simulink model "bu_abslut125_romvect_float"  (R2021b)
settings: Solver=VariableStepAuto  StartTime=0.0  StopTime=350  RelTol=1e-3
undefined symbols (not defined in the file or in its folder): figd2104, xcu250
libraries: hdlBasic x1696, vmcUtilities x1
(part 2 of 8)

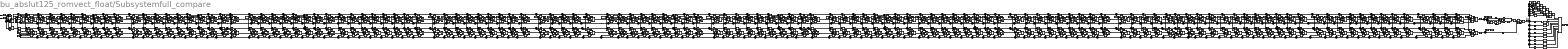
== system bu_abslut125_romvect_float/Subsystemfull_compare ==
  note: 120
  note: 110
  note: 100
  note: 90
  note: 80
  note: 70
  note: 30
  note: 01
  note: 50
  note: 40
  note: 20
  note: 10
  note: tiisai
  note: ooki
  note: 7874no13bit
  note: tmp_2
  note: tmp_3
  note: truthtable_out_x
  note: truthtable_out_y
  note: 1-1000
  note: 1001-2000
  note: 2001-3000
  note: 60
  note: 125
  note: 5001-6000
  note: 3001-4000
  note: 4001-5000
  note: 6001-7000
  note: 7001-7874
  In3 : Inport
  In4 : Inport  Port=2
  AddSub{,1..17,23..95,97..201,205..207,209..211,236,238,249..250,252,254..258,261..269,271..280,282..291,293..299} (248 alike) : hdlBasic/AddSub  mode=Addition  use_carryin=off  use_carryout=off  en=off  latency=1  precision=User Defined  arith_type="Signed  (2's comp)"  n_bits=32  bin_pt=0  quantization=Truncate  overflow=Wrap  use_behavioral_HDL=off  hw_selection=Fabric  pipelined=off  XmcBlockStatus=1  maskContainerNames=tabcontainer1  block_type=addsub  block_config=sysgen:Addsub_config
  AddSub18 : hdlBasic/AddSub  mode=Subtraction  use_carryin=off  use_carryout=off  en=off  latency=1  precision=Full  arith_type=Unsigned  n_bits=5  bin_pt=0  quantization=Truncate  overflow=Wrap  use_behavioral_HDL=off  hw_selection=Fabric  pipelined=off  XmcBlockStatus=1  maskContainerNames=tabcontainer1  block_type=addsub  block_config=sysgen:Addsub_config
  AddSub19 : hdlBasic/AddSub  mode=Addition  use_carryin=off  use_carryout=off  en=off  latency=1  precision=Full  arith_type=Unsigned  n_bits=16  bin_pt=14  quantization=Truncate  overflow=Wrap  use_behavioral_HDL=off  hw_selection=Fabric  pipelined=off  XmcBlockStatus=1  maskContainerNames=tabcontainer1  block_type=addsub  block_config=sysgen:Addsub_config
  AddSub20 : hdlBasic/AddSub  mode=Subtraction  use_carryin=off  use_carryout=off  en=off  latency=1  precision=User Defined  arith_type=Unsigned  n_bits=15  bin_pt=0  quantization="Round  (unbiased: +/- Inf)"  overflow=Saturate  use_behavioral_HDL=off  hw_selection=Fabric  pipelined=off  XmcBlockStatus=1  maskContainerNames=tabcontainer1  block_type=addsub  block_config=sysgen:Addsub_config
  AddSub{96,202..204,208,212} (6 alike) : hdlBasic/AddSub  mode=Addition  use_carryin=off  use_carryout=off  en=off  latency=1  precision=User Defined  arith_type=Unsigned  n_bits=3  bin_pt=0  quantization=Truncate  overflow=Wrap  use_behavioral_HDL=off  hw_selection=Fabric  pipelined=off  XmcBlockStatus=1  maskContainerNames=tabcontainer1  block_type=addsub  block_config=sysgen:Addsub_config
  AddSub21 : hdlBasic/AddSub  mode=Addition  use_carryin=off  use_carryout=off  en=off  latency=1  precision=Full  arith_type=Unsigned  n_bits=16  bin_pt=14  quantization=Truncate  overflow=Wrap  use_behavioral_HDL=off  hw_selection=Fabric  pipelined=off  XmcBlockStatus=1  maskContainerNames=tabcontainer1  block_type=addsub  block_config=sysgen:Addsub_config
  AddSub22 : hdlBasic/AddSub  mode=Subtraction  use_carryin=off  use_carryout=off  en=off  latency=1  precision=Full  arith_type=Unsigned  n_bits=17  bin_pt=0  quantization=Truncate  overflow=Wrap  use_behavioral_HDL=off  hw_selection=Fabric  pipelined=off  XmcBlockStatus=1  maskContainerNames=tabcontainer1  block_type=addsub  block_config=sysgen:Addsub_config
  Constant : hdlBasic/Constant  const=1.0  gui_display_data_type=Fixed-point  arith_type=Unsigned  n_bits=1  bin_pt=0  preci_type=Single  exp_width=8  frac_width=24  explicit_period=on  period=1  XmcBlockStatus=1  maskContainerNames=tabcontainer1  block_type=constant  block_config=sysgen:Constant_config
  Constant1 : hdlBasic/Constant  const=0  gui_display_data_type=Fixed-point  arith_type=Signed (2's comp)  n_bits=32  bin_pt=0  preci_type=Single  exp_width=8  frac_width=24  explicit_period=on  period=1  XmcBlockStatus=1  maskContainerNames=tabcontainer1  block_type=constant  block_config=sysgen:Constant_config
  Constant10 : hdlBasic/Constant  const=3000  gui_display_data_type=Fixed-point  arith_type=Unsigned  n_bits=12  bin_pt=0  preci_type=Single  exp_width=8  frac_width=24  explicit_period=on  period=1  XmcBlockStatus=1  maskContainerNames=tabcontainer1  block_type=constant  block_config=sysgen:Constant_config
  Constant11 : hdlBasic/Constant  const=4000  gui_display_data_type=Fixed-point  arith_type=Unsigned  n_bits=12  bin_pt=0  preci_type=Single  exp_width=8  frac_width=24  explicit_period=on  period=1  XmcBlockStatus=1  maskContainerNames=tabcontainer1  block_type=constant  block_config=sysgen:Constant_config
  Constant12 : hdlBasic/Constant  const=5000  gui_display_data_type=Fixed-point  arith_type=Unsigned  n_bits=13  bin_pt=0  preci_type=Single  exp_width=8  frac_width=24  explicit_period=on  period=1  XmcBlockStatus=1  maskContainerNames=tabcontainer1  block_type=constant  block_config=sysgen:Constant_config
  Constant13 : hdlBasic/Constant  const=6000  gui_display_data_type=Fixed-point  arith_type=Unsigned  n_bits=13  bin_pt=0  preci_type=Single  exp_width=8  frac_width=24  explicit_period=on  period=1  XmcBlockStatus=1  maskContainerNames=tabcontainer1  block_type=constant  block_config=sysgen:Constant_config
  Constant14 : hdlBasic/Constant  const=7000  gui_display_data_type=Fixed-point  arith_type=Unsigned  n_bits=13  bin_pt=0  preci_type=Single  exp_width=8  frac_width=24  explicit_period=on  period=1  XmcBlockStatus=1  maskContainerNames=tabcontainer1  block_type=constant  block_config=sysgen:Constant_config
  Constant2 : hdlBasic/Constant  const=1  gui_display_data_type=Fixed-point  arith_type=Signed (2's comp)  n_bits=32  bin_pt=0  preci_type=Single  exp_width=8  frac_width=24  explicit_period=on  period=1  XmcBlockStatus=1  maskContainerNames=tabcontainer1  block_type=constant  block_config=sysgen:Constant_config
  Constant3 : hdlBasic/Constant  const=248  gui_display_data_type=Fixed-point  arith_type=Unsigned  n_bits=8  bin_pt=0  preci_type=Single  exp_width=8  frac_width=24  explicit_period=on  period=1  XmcBlockStatus=1  maskContainerNames=tabcontainer1  block_type=constant  block_config=sysgen:Constant_config
  Constant4 : hdlBasic/Constant  const=125  gui_display_data_type=Fixed-point  arith_type=Unsigned  n_bits=7  bin_pt=0  preci_type=Single  exp_width=8  frac_width=24  explicit_period=on  period=1  XmcBlockStatus=1  maskContainerNames=tabcontainer1  block_type=constant  block_config=sysgen:Constant_config
  Constant5 : hdlBasic/Constant  const=1.0  gui_display_data_type=Fixed-point  arith_type=Unsigned  n_bits=10  bin_pt=0  preci_type=Single  exp_width=8  frac_width=24  explicit_period=on  period=1  XmcBlockStatus=1  maskContainerNames=tabcontainer1  block_type=constant  block_config=sysgen:Constant_config
  Constant6 : hdlBasic/Constant  const=0  gui_display_data_type=Fixed-point  arith_type=Signed (2's comp)  n_bits=32  bin_pt=0  preci_type=Single  exp_width=8  frac_width=24  explicit_period=on  period=1  XmcBlockStatus=1  maskContainerNames=tabcontainer1  block_type=constant  block_config=sysgen:Constant_config
  Constant7 : hdlBasic/Constant  const=1  gui_display_data_type=Fixed-point  arith_type=Signed (2's comp)  n_bits=32  bin_pt=0  preci_type=Single  exp_width=8  frac_width=24  explicit_period=on  period=1  XmcBlockStatus=1  maskContainerNames=tabcontainer1  block_type=constant  block_config=sysgen:Constant_config
  Constant8 : hdlBasic/Constant  const=1000  gui_display_data_type=Fixed-point  arith_type=Unsigned  n_bits=10  bin_pt=0  preci_type=Single  exp_width=8  frac_width=24  explicit_period=on  period=1  XmcBlockStatus=1  maskContainerNames=tabcontainer1  block_type=constant  block_config=sysgen:Constant_config
  Constant9 : hdlBasic/Constant  const=2000  gui_display_data_type=Fixed-point  arith_type=Unsigned  n_bits=11  bin_pt=0  preci_type=Single  exp_width=8  frac_width=24  explicit_period=on  period=1  XmcBlockStatus=1  maskContainerNames=tabcontainer1  block_type=constant  block_config=sysgen:Constant_config
  Convert23 : hdlBasic/Convert  Commented=on  gui_display_data_type=Fixed-point  arith_type=Unsigned  n_bits=13  bin_pt=0  float_type=Single  exp_bits=8  fraction_bits=24  quantization="Round  (unbiased: +/- Inf)"  overflow=Saturate  en=off  latency=1  pipeline=off  XmcBlockStatus=1  maskContainerNames=group2  block_type=convert  block_config=sysgen:Convert_config
  Delay{1..7,9..10,12..13,15..16,19..20,22..23,25..26,28..29,31..32,34..35,37..38,41..42,44..45,47..48,50..52,54..56,58,62,64..65,67..68,71..72,74..75,77..78,80..82,84..85,87..88,91..92,94..95,97..98,100..103,105..107,109..115,117..118,120..125,127..129,131,133..134,136..138,140..141,143..144,147..148,150..151,153..154,156..158,160..161,163..164,167..168,170..171,173..174,176..180,182..184,186,188..189,191..192,194..196,199..200,202..205,207,209..214,217..218,220..221,224..227,229,231..236,238..240,242..243,245,247..248,251..255,257..258,260..261,263..264,266..267,269..270,272..273,275..276,279..280,282..283,285..286,288..290,292..293,295..296,298..299,302..303,305..306,308..309,311..313,315..316,318..319,321,323..324,326..327,329..330,332..333,335..338,340,342..343,345..347,350..351,353..354,357..358,360..362,364..365,367..369,371..373,375..376,379..380,383..384,386..387,389..392,394,396..398,400,402..404,406..407,409..414,416..419,421,423,426..427,429..431,433..435,437..438,440,442..443,446,448..449,451..453,455..456,458..459,461,463,465..466,468..469,472..474,476..477,479..480,482..485,487..488,490..491,493..494,498..499,501..502,504..506,508..510,512..513,515..517,519,521..522,524..525,527,529,531..532,534..535,538..539,541..542,544..545,548..550,553..554,556..558,560..561,563..564,566,568..569,571..572,574..575,578..580,582..583,585..586,588,590..591,593..594,596..597,605,611..614,624..625,636..637,639..640,655..656,658..659,661..662,677..678,680..681,683..686,688,690..692,694,696..697,700..701,703..706,708,710..713,715,717,720..721,724..725,727,729,731..732,734,736..737,742..743,746..747,749..750,752..753,755,757,759..760,762..763,766,768,770..771,773..774,776..777,779,781..782,784..785,787..788,792..793,795..796,798..799,802..804,806..807,809..810,813,815..816,818..819,821,823} (503 alike) : hdlBasic/Delay  rst=off  en=off  latency=1  reg_retiming=off  XmcBlockStatus=1  maskContainerNames=group1  block_type=delay  block_config=sysgen:Delay_config
  Delay{8,11,14,17..18,21,24,27,30,33,36,39..40,43,46,49,53,57,63,66,69..70,73,76,79,83,86,89..90,93,96,99,104,108,116,119,126,130,132,135,139,142,145..146,149,152,155,159,162,165..166,169,172,175,181,185,187,190,193,201,206,215..216,219,222..223,228,230,237,241,244,246,249..250,256,259,262,265,268,271,274,277..278,281,284,287,291,294,297,300..301,304,307,310,314,317,320,322,325,328,331,334,339,341,344,348..349,352,355..356,359,363,366,370,374,377..378,381..382,385,388,393,395,399,401,405,408,415,420,422,424..425,428,432,436,439,441,444..445,447,450,454,457,460,462,464,467,470..471,475,478,481,486,489,492,495..497,500,503,507,511,514,518,520,523,526,528,530,533,536..537,540,543,546..547,551..552,555,559,562,565,567,570,573,576..577,581,584,587,589,592,595,598,606,610,615..617,635,638,657,660,679,682,689,693,695,699,702,709,714,718..719,722,726,730,735,738..739,741,744,748,751,754,758,761,764..765,769,772,775,780,783,786,790..791,794,797,801,805,808,812,814,817,820,824} (247 alike) : hdlBasic/Delay  rst=off  en=off  latency=2  reg_retiming=off  XmcBlockStatus=1  maskContainerNames=group1  block_type=delay  block_config=sysgen:Delay_config
  Delay{197..198,208,599..603} (8 alike) : hdlBasic/Delay  rst=off  en=off  latency=6  reg_retiming=off  XmcBlockStatus=1  maskContainerNames=group1  block_type=delay  block_config=sysgen:Delay_config
  Delay59 : hdlBasic/Delay  rst=off  en=off  latency=3  reg_retiming=off  XmcBlockStatus=1  maskContainerNames=group1  block_type=delay  block_config=sysgen:Delay_config
  Delay60 : hdlBasic/Delay  rst=off  en=off  latency=3  reg_retiming=off  XmcBlockStatus=1  maskContainerNames=group1  block_type=delay  block_config=sysgen:Delay_config
  Delay604 : hdlBasic/Delay  rst=off  en=off  latency=133  reg_retiming=off  XmcBlockStatus=1  maskContainerNames=group1  block_type=delay  block_config=sysgen:Delay_config
  Delay607 : hdlBasic/Delay  rst=off  en=off  latency=3  reg_retiming=off  XmcBlockStatus=1  maskContainerNames=group1  block_type=delay  block_config=sysgen:Delay_config
  Delay608 : hdlBasic/Delay  rst=off  en=off  latency=4  reg_retiming=off  XmcBlockStatus=1  maskContainerNames=group1  block_type=delay  block_config=sysgen:Delay_config
  Delay609 : hdlBasic/Delay  rst=off  en=off  latency=5  reg_retiming=off  XmcBlockStatus=1  maskContainerNames=group1  block_type=delay  block_config=sysgen:Delay_config
  Delay61 : hdlBasic/Delay  rst=off  en=off  latency=5  reg_retiming=off  XmcBlockStatus=1  maskContainerNames=group1  block_type=delay  block_config=sysgen:Delay_config
  Gate_In1 : hdlBasic/Gateway In  gui_display_data_type=Floating-point  arith_type=Floating-point  n_bits=16  bin_pt=15  preci_type=Double  exp_width=8  frac_width=24  rows=1  columns=1  quantization="Round  (unbiased: +/- Inf)"  overflow=Saturate  period=1  UseAsADC=off  ADCChannel='1'  interface=None  automatic_assignment=on  address_offset=hex2dec('00')  intf_name=''  intf_description=''  default_value=0  timing_constraint=None  locs_specified=off  LOCs={}  io_standard={}  inherit_from_input=off  hdl_port=on  XmcBlockStatus=1  maskContainerNames=group4  block_type=gatewayin  block_config=sysgen:gateway_in_config  block_width_w=590  block_height_w=620  block_width=640  block_height=850
  Gate_In2 : hdlBasic/Gateway In  gui_display_data_type=Floating-point  arith_type=Floating-point  n_bits=16  bin_pt=15  preci_type=Double  exp_width=8  frac_width=24  rows=1  columns=1  quantization="Round  (unbiased: +/- Inf)"  overflow=Saturate  period=1  UseAsADC=off  ADCChannel='1'  interface=None  automatic_assignment=on  address_offset=hex2dec('00')  intf_name=''  intf_description=''  default_value=0  timing_constraint=None  locs_specified=off  LOCs={}  io_standard={}  inherit_from_input=off  hdl_port=on  XmcBlockStatus=1  maskContainerNames=group4  block_type=gatewayin  block_config=sysgen:gateway_in_config  block_width_w=590  block_height_w=620  block_width=640  block_height=850
  Gateway Out : hdlBasic/Gateway Out  inherit_from_input=off  hdl_port=on  rows=1  columns=1  UseAsDAC=off  DACChannel='1'  interface=None  automatic_assignment=on  address_offset=hex2dec('00')  intf_name=''  intf_description=''  timing_constraint=None  locs_specified=off  LOCs={}  io_standard={}  XmcBlockStatus=1  maskContainerNames=group4  block_type=gatewayout  block_config=sysgen:gateway_out_config  block_width_w=590  block_height_w=620  block_width=620  block_height=750
  Gateway Out1 : hdlBasic/Gateway Out  inherit_from_input=off  hdl_port=on  rows=1  columns=1  UseAsDAC=off  DACChannel='1'  interface=None  automatic_assignment=on  address_offset=hex2dec('00')  intf_name=''  intf_description=''  timing_constraint=None  locs_specified=off  LOCs={}  io_standard={}  XmcBlockStatus=1  maskContainerNames=group4  block_type=gatewayout  block_config=sysgen:gateway_out_config  block_width_w=590  block_height_w=620  block_width=620  block_height=750
  Gateway Out2 : hdlBasic/Gateway Out  inherit_from_input=off  hdl_port=on  rows=1  columns=1  UseAsDAC=off  DACChannel='1'  interface=None  automatic_assignment=on  address_offset=hex2dec('00')  intf_name=''  intf_description=''  timing_constraint=None  locs_specified=off  LOCs={}  io_standard={}  XmcBlockStatus=1  maskContainerNames=group4  block_type=gatewayout  block_config=sysgen:gateway_out_config  block_width_w=590  block_height_w=620  block_width=620  block_height=750
  Mult : hdlBasic/Mult  precision=Full  arith_type="Signed  (2's comp)"  n_bits=30  bin_pt=16  quantization="Round  (unbiased: +/- Inf)"  overflow=Saturate  en=off  latency=1  use_behavioral_HDL=off  opt=Area  use_embedded=off  optimum_pipeline=off  pipeline=on  use_rpm=on  placement_style=Triangular  XmcBlockStatus=1  maskContainerNames=group1  block_type=mult  block_config=sysgen:Mult_config
  Mult1 : hdlBasic/Mult  precision=Full  arith_type="Signed  (2's comp)"  n_bits=16  bin_pt=14  quantization=Truncate  overflow=Wrap  en=off  latency=1  use_behavioral_HDL=off  opt=Area  use_embedded=off  optimum_pipeline=off  pipeline=on  use_rpm=on  placement_style=Triangular  XmcBlockStatus=1  maskContainerNames=group1  block_type=mult  block_config=sysgen:Mult_config
  Mux{,1..92,95..117,119..200,204..207,237..238,247..249,254..260,262..271,273..282,284..293,295..300} (250 alike) : hdlBasic/Mux  inputs=2  en=off  latency=1  precision=Full  arith_type=Unsigned  n_bits=16  bin_pt=14  quantization=Truncate  overflow=Wrap  XmcBlockStatus=1  maskContainerNames=tabcontainer1  block_type=mux  block_config=sysgen:Mux_config
  Mux93 : hdlBasic/Mux  inputs=8  en=off  latency=1  precision=Full  arith_type=Unsigned  n_bits=16  bin_pt=14  quantization=Truncate  overflow=Wrap  XmcBlockStatus=1  maskContainerNames=tabcontainer1  block_type=mux  block_config=sysgen:Mux_config
  Negate : hdlBasic/Negate  precision=Full  arith_type=Unsigned  n_bits=16  bin_pt=14  quantization=Truncate  overflow=Wrap  en=off  latency=1  XmcBlockStatus=1  maskContainerNames=tabcontainer1  block_type=negate  block_config=sysgen:Negate_config
  ROM : hdlBasic/ROM  depth=7874  initVector=[1.41421356237310,1.40285497510094,1.39140366620579,1.39159062000793,1.38004584520208,1.36859377003848,1.38042280392127,1.36878383930820,1.35723674105880,1.34578387387117,1.36935388882523,1.35762003300122,1.34597716419517,1.33442766399181,1.32297397770386,1.35838629242896,1.34655686869302,1.33481750556133,1.32317060012862,1.31161861541368,1.30016408153656,1.34752248865841,1.33559684733291,1.32376029217311,1.31201523429647,1.30036415295138,1.28880959683697,1.27735418536925,1.33676500806409,1.32474252892781,1.31280811258869,1.30096418258553,1.28921323279952,1.27755782892341,1.26600060988325,1.25454428920194,1.32611643813513,1.31399653297018,1.30196361745875,1.29002012584225,1.27816856491348,1.26641151564217,1.25475163475979,1.24319165629311,1.23173439303463,1.31557942351002,1.30336153876367,1.29122951997583,1.27918581025151,1.26723292744615,1.25537346595420,1.24361009846460,1.23194557767279,1.22038273793722,1.20892449686732,1.30515666607380,1.29284028563560,1.28060859621156,1.26846404780850,1.25640916736454,1.24444656070712,1.23257891448663,1.22080899807524,1.20913966541879,1.19757385682881,1.18611460070002,1.29485092493073,1.28243557302479,1.27010368532968,1.25785771666743,1.24570020094514,1.23363375328858,1.22166107216123,1.20978494145801,1.19800823256193,1.18633390635054,1.17476501513743,1.16330470453271,1.28466501624128,1.27215026043297,1.25971768966236,1.24736976135389,1.23510901413398,1.22293807014628,1.21085963736280,1.19887651188052,1.18699158019188,1.17520782141593,1.16352830947558,1.15195621520446,1.14049480836540,1.27460181291164,1.26198726722700,1.24945357463641,1.23700319282671,1.22463866275666,1.21236261115911,1.20017775305069,1.18808689423890,1.17609293381511,1.16419886662055,1.15240778567073,1.14072288452174,1.12914745956046,1.11768491219809,1.26466424412340,1.25194957227903,1.23931436853539,1.22676108837461,1.21429227256250,1.20191054984267,1.18961863965070,1.17741935483871,1.16531560439925,1.15331039617579,1.14140683954543,1.12960814805762,1.11791764201055,1.10633875094468,1.09487501603078,1.25485529469096,1.24204021343087,1.22930316208331,1.21664659133201,1.20407303908639,1.19158513337186,1.17918559525382,1.16687724178619,1.15466298897390,1.14254585473709,1.13052896186291,1.11861554092901,1.10680893318050,1.09511259333987,1.08353009232700,1.07206511986348,1.24517800423347,1.23226228676865,1.21942310783457,1.20666291059794,1.19398422731108,1.18138968240193,1.16888199561248,1.15646398517699,1.14413857103021,1.13190877803373,1.11977773920708,1.10774869894792,1.09582501622342,1.08401016771268,1.07230775087707,1.06072148693273,1.04925522369617,1.23563546614805,1.22261894569337,1.20967741935484,1.19681331994124,1.18402917111180,1.17132759066873,1.15871129391367,1.14618309706064,1.13374592069613,1.12140279327540,1.10915685464221,1.09701135955690,1.08496968121562,1.07303531474064,1.06121188061910,1.04950312806435,1.03791293827072,1.02644532752886,1.22623082637085,1.21311339977250,1.20006937017666,1.18710115707466,1.17421127246460,1.16140232434804,1.14867702030741,1.13603817115744,1.12348869466245,1.11103161930932,1.09867008812428,1.08640736251928,1.07424682615140,1.06219198877593,1.05024649007095,1.03841410340773,1.02669873953804,1.01510445016513,1.00363543136155,1.21696728191211,1.20374891335776,1.19060229251359,1.17752982248026,1.16453400039901,1.15161742115315,1.13878278116799,1.12603288230368,1.11337063583370,1.10079906650010,1.08832131663467,1.07594065033277,1.06366045766436,1.05148425890365,1.03941570875600,1.02745860055697,1.01561687041491,1.00389460126422,0.992296026791744,0.980825535194243,1.20784807915155,1.19452880395390,1.18127957571616,1.16810277796774,1.15500088967536,1.14197648914896,1.12903225806452,1.11617098559974,1.10339557267659,1.09070903630301,1.07811451400441,1.06561526833283,1.05321469143965,1.04091630969436,1.02872378832916,1.01664093608512,1.00467170983209,0.992820219129832,0.981090730693261,0.969487672719272,0.958015639026935,1.19887651188052,1.18545644032342,1.17210466445317 ...(+27333 chars)]  distributed_mem=Block RAM  rst=off  init_reg=0  en=off  latency=1  gui_display_data_type=Floating-point  arith_type=Floating-point  n_bits=16  bin_pt=15  preci_type=Double  exp_width=8  frac_width=24  optimize=Area  use_rpm=on  simulation_type=fast_sim  XmcBlockStatus=1  maskContainerNames=tabcontainer1  block_type=sprom  block_config=sysgen:SPROM_config
  ROM1 : hdlBasic/ROM  depth=7874  initVector=[0,0,0,0,0,0,0,0,0,0,0,0,0,0,0,0,0,0,0,0,0,0,0,0,0,0,0,0,0,0,0,0,0,0,0,0,0,0,0,0,0,0,0,0,0,0,0,0,0,0,0,0,0,0,0,0,0,0,0,0,0,0,0,0,0,0,0,0,0,0,0,0,0,0,0,0,0,0,0,0,0,0,0,0,0,0,0,0,0,0,0,0,0,0,0,0,0,0,0,0,0,0,0,0,0,0,0,0,0,0,0,0,0,0,0,0,0,0,0,0,0,0,0,0,0,0,0,0,0,0,0,0,0,0,0,0,0,0,0,0,0,0,0,0,0,0,0,0,0,0,0,0,0,0,0,0,0,0,0,0,0,0,0,0,0,0,0,0,0,0,0,0,0,0,0,0,0,0,0,0,0,0,0,0,0,0,0,0,0,0,0,0,0,0,0,0,0,0,0,0,0,0,0,0,0,0,0,0,0,0,0,0,0,0,0,0,0,0,0,0,0,0,0,0,0,0,0,0,0,0,0,0,0,0,0,0,0,0,0,0,0,0,0,0,0,0,0,0,0,0,0,0,0,0,0,0,0,0,0,0,0,0,0,0,0,0,0,0,0,0,0,0,0,0,0,0,0,0,0,0,0,0,0,0,0,0,0,0,0,0,0,0,0,0,0,0,0,0,0,0,0,0,0,0,0,0,0,0,0,0,0,0,0,0,0,0,0,0,0,0,0,0,0,0,0,0,0,0,0,0,0,0,0,0,0,0,0,0,0,0,0,0,0,0,0,0,0,0,0,0,0,0,0,0,0,0,0,0,0,0,0,0,0,0,0,0,0,0,0,0,0,0,0,0,0,0,0,0,0,0,0,0,0,0,0,0,0,0,0,0,0,0,0,0,0,0,0,0,0,0,0,0,0,0,0,0,0,0,0,0,0,0,0,0,0,0,0,0,0,0,0,0,0,0,0,0,0,0,0,0,0,0,0,0,0,0,0,0,0,0,0,0,0,0,0,0,0,0,0,0,0,0,0,0,0,0,0,0,0,0,0,0,0,0,0,0,0,0,0,0,0,0,0,0,0,0,0,0,0,0,0,0,0,0,0,0,0,0,0,0,0,0,0,0,0,0,0,0,0,0,0,0,0,0,0,0,0,0,0,0,0,0,0,0,0,0,0,0,0,0,0,0,0,0,0,0,0,0,0,0,0,0,0,0,0,0,0,0,0,0,0,0,0,0,0,0,0,0,0,0,0,0,0,0,0,0,0,0,0,0,0,0,0,0,0,0,0,0,0,0,0,0,0,0,0,0,0,0,0,0,0,0,0,0,0,0,0,0,0,0,0,0,0,0,0,0,0,0,0,0,0,0,0,0,0,0,0,0,0,0,0,0,0,0,0,0,0,0,0,0,0,0,0,0,0,0,0,0,0,0,0,0,0,0,0,0,0,0,0,0,0,0,0,0,0,0,0,0,0,0,0,0,0,0,0,0,0,0,0,0,0,0,0,0,0,0,0,0,0,0,0,0,0,0,0,0,0,0,0,0,0,0,0,0,0,0,0,0,0,0,0,0,0,0,0,0,0,0,0,0,0,0,0,0,0,0,0,0,0,0,0,0,0,0,0,0,0,0,0,0,0,0,0,0,0,0,0,0,0,0,0,0,0,0,0,0,0,0,0,0,0,0,0,0,0,0,0,0,0,0,0,0,0,0,0,0,0,0,0,0,0,0,0,0,0,0,0,0,0,0,0,0,0,0,0,0,0,0,0,0,0,0,0,0,0,0,0,0,0,0,0,0,0,0,0,0,0,0,0,0,0,0,0,0,0,0,0,0,0,0,0,0,0,0,0,0,0,0,0,0,0,0,0,0,0,0,0,0,0,0,0,0,0,0,0,0,0,0,0,0,0,0,0,0,0,0,0,0,0,0,0,0,0,0,0,0,0,0,0,0,0,0,0,0,0,0,0,0,0,0,0,0,0,0,0,0,0,0,0,0,0,0,0,0,0,0,0,0,0,0,0,0,0,0,0,0,0,0,0,0,0,0,0,0,0,0,0,0,0,0,0,0,0,0,0,0,0,0,0,0,0,0,0,0,0,0,0,0,0,0,0,0,0,0,0,0,0,0,0,0,0,0,0,0,0,0,0,0,0,0,0,0,0,0,0,0,0,0,0,0,0,0,0,0,0,0,0,0,0,0,0,0,0,0,0,0,0,0,0,0,0,0,0,0,0,0,0,0,0,0,0,0,0,0,0,0,0,0,0,0,0.887536547883716,0.872310792450965,0.857118081005576,0.841960202331496,0.826839072127503,0.811756744010427,0.796715421627643,0.781717472003396,0.766765440258369,0.751862065858495,0.737010300567475,0.722213328298004,0.707474587079397,0.692797793384340,0.678186969084795,0.663646471336806,0.649181025725745,0.634795763037240,0.620496260053914,0.606288584813307,0.592179346796317,0.578175752546288,0.564285667243094,0.550517682770194,0.536881192809459,0.523386475470579,0.510044783898126,0.496868445185463,0.483870967741935,0.471067156984201,0.458473238824255,0.446106989869011,0.433987872486249,0.422137171880723,0.410578131011544,1.03690988131906,1.02136388380565,1.00583624694638,0.990327834387661,0.974839563629779,0.959372410191165,0.943927412154809,0.928505675137049,0.913108377723752,0.897736777424242,0.882392217199350,0.867076132626814,0.851790059774896,0.836535643863867,0.821314648804775,0.806128967716116,0.790980634531563,0.775871836826174,0.760804930004565,0.745782453012703,0.730807145755432,0.715881968424908,0.701010122970991,0.686195076973634,0.671440590209634,0.656750744242011,0.642129975399819,0.627583111559475,0.613115413185426,0.598732619137761,0.584440997806240,0.570247404182700,0.556159343534409,0.542185042386181,0.528333527553523,0.514614713985285,0.501039502161583,0.487619885736483,0.474369069995250,0.461301601486293,0.448433508853479,0.435782454390526,0.423367895109893,0.411211251096192,0.399336077520643,0.387768234844236,1.03276197377949,1.01715258228565,1.00155965782323,0.985983981650189,0.970426384289763,0.954887749394560,0.939369017971680,0.923871193007722,0.908395344537337,0.892942615204284,0.877514226370029,0.862111484831792,0.846735790219786,0.831388643152250,0.816071654237001,0.800786554019768,0.785535203992640,0.770319608790939,0.755141929723847,0.740004499803514,0.724909840459491,0.709860680150496,0.694859975114130,0.679910932527677,0.665017036389945,0.650182076475690,0.635410180761039,0.620705851770770,0.606074007356643,0.591520026480395 ...(+27729 chars)]  distributed_mem=Block RAM  rst=off  init_reg=0  en=off  latency=1  gui_display_data_type=Floating-point  arith_type=Floating-point  n_bits=16  bin_pt=15  preci_type=Double  exp_width=8  frac_width=24  optimize=Area  use_rpm=on  simulation_type=fast_sim  XmcBlockStatus=1  maskContainerNames=tabcontainer1  block_type=sprom  block_config=sysgen:SPROM_config
  ROM2 : hdlBasic/ROM  depth=7874  initVector=[0,0,0,0,0,0,0,0,0,0,0,0,0,0,0,0,0,0,0,0,0,0,0,0,0,0,0,0,0,0,0,0,0,0,0,0,0,0,0,0,0,0,0,0,0,0,0,0,0,0,0,0,0,0,0,0,0,0,0,0,0,0,0,0,0,0,0,0,0,0,0,0,0,0,0,0,0,0,0,0,0,0,0,0,0,0,0,0,0,0,0,0,0,0,0,0,0,0,0,0,0,0,0,0,0,0,0,0,0,0,0,0,0,0,0,0,0,0,0,0,0,0,0,0,0,0,0,0,0,0,0,0,0,0,0,0,0,0,0,0,0,0,0,0,0,0,0,0,0,0,0,0,0,0,0,0,0,0,0,0,0,0,0,0,0,0,0,0,0,0,0,0,0,0,0,0,0,0,0,0,0,0,0,0,0,0,0,0,0,0,0,0,0,0,0,0,0,0,0,0,0,0,0,0,0,0,0,0,0,0,0,0,0,0,0,0,0,0,0,0,0,0,0,0,0,0,0,0,0,0,0,0,0,0,0,0,0,0,0,0,0,0,0,0,0,0,0,0,0,0,0,0,0,0,0,0,0,0,0,0,0,0,0,0,0,0,0,0,0,0,0,0,0,0,0,0,0,0,0,0,0,0,0,0,0,0,0,0,0,0,0,0,0,0,0,0,0,0,0,0,0,0,0,0,0,0,0,0,0,0,0,0,0,0,0,0,0,0,0,0,0,0,0,0,0,0,0,0,0,0,0,0,0,0,0,0,0,0,0,0,0,0,0,0,0,0,0,0,0,0,0,0,0,0,0,0,0,0,0,0,0,0,0,0,0,0,0,0,0,0,0,0,0,0,0,0,0,0,0,0,0,0,0,0,0,0,0,0,0,0,0,0,0,0,0,0,0,0,0,0,0,0,0,0,0,0,0,0,0,0,0,0,0,0,0,0,0,0,0,0,0,0,0,0,0,0,0,0,0,0,0,0,0,0,0,0,0,0,0,0,0,0,0,0,0,0,0,0,0,0,0,0,0,0,0,0,0,0,0,0,0,0,0,0,0,0,0,0,0,0,0,0,0,0,0,0,0,0,0,0,0,0,0,0,0,0,0,0,0,0,0,0,0,0,0,0,0,0,0,0,0,0,0,0,0,0,0,0,0,0,0,0,0,0,0,0,0,0,0,0,0,0,0,0,0,0,0,0,0,0,0,0,0,0,0,0,0,0,0,0,0,0,0,0,0,0,0,0,0,0,0,0,0,0,0,0,0,0,0,0,0,0,0,0,0,0,0,0,0,0,0,0,0,0,0,0,0,0,0,0,0,0,0,0,0,0,0,0,0,0,0,0,0,0,0,0,0,0,0,0,0,0,0,0,0,0,0,0,0,0,0,0,0,0,0,0,0,0,0,0,0,0,0,0,0,0,0,0,0,0,0,0,0,0,0,0,0,0,0,0,0,0,0,0,0,0,0,0,0,0,0,0,0,0,0,0,0,0,0,0,0,0,0,0,0,0,0,0,0,0,0,0,0,0,0,0,0,0,0,0,0,0,0,0,0,0,0,0,0,0,0,0,0,0,0,0,0,0,0,0,0,0,0,0,0,0,0,0,0,0,0,0,0,0,0,0,0,0,0,0,0,0,0,0,0,0,0,0,0,0,0,0,0,0,0,0,0,0,0,0,0,0,0,0,0,0,0,0,0,0,0,0,0,0,0,0,0,0,0,0,0,0,0,0,0,0,0,0,0,0,0,0,0,0,0,0,0,0,0,0,0,0,0,0,0,0,0,0,0,0,0,0,0,0,0,0,0,0,0,0,0,0,0,0,0,0,0,0,0,0,0,0,0,0,0,0,0,0,0,0,0,0,0,0,0,0,0,0,0,0,0,0,0,0,0,0,0,0,0,0,0,0,0,0,0,0,0,0,0,0,0,0,0,0,0,0,0,0,0,0,0,0,0,0,0,0,0,0,0,0,0,0,0,0,0,0,0,0,0,0,0,0,0,0,0,0,0,0,0,0,0,0,0,0,0,0,0,0,0,0,0,0,0,0,0,0,0,0,0,0,0,0,0,0,0,0,0,0,0,0,0,0,0,0,0,0,0,0,0,0,0,0,0,0,0,0,0,0,0,0,0,0,0,0,0,0,0,0,0,0,0,0,0,0,0,0,0,0,0,0,0,0,0,0,0,0,0,0,0,0,0,0,0,0,0,0,0,0,0,0,0,0,0,0,0,0,0,0,0,0,0,0,0,0,0,0,0,0,0,0,0,0,0,0,0,0,0,0,0,0,0,0,0,0,0,0,0,0,0,0,0,0,0,0,0,0,0,0,0,0,0,0,0,0,0,0,0,0,0,0,0,0,0,0,0,0,0,0,0,0,0,0,0,0,0,0,0,0,0,0,0,0,0,0,0,0,0,0,0,0,0,0,0,0,0,0,0,0,0,0,0,0,0,0,0,0,0,0,0,0,0,0,0,0,0,0,0,0,0,0,0,0,0,0,0,0,0,0,0,0,0,0,0,0,0,0,0,0,0,0,0,0,0,0,0,0,0,0,0,0,0,0,0,0,0,0,0,0,0,0,0,0,0,0,0,0,0,0,0,0,0,0,0,0,0,0,0,0,0,0,0,0,0,0,0,0,0,0,0,0,0,0,0,0,0,0,0,0,0,0,0,0,0,0,0,0,0,0,0,0,0,0,0,0,0,0,0,0,0,0,0,0,0,0,0,0,0,0,0,0,0,0,0,0,0,0,0,0,0,0,0,0,0,0,0,0,0,0,0,0,0,0,0,0,0,0,0,0,0,0,0,0,0,0,0,0,0,0,0,0,0,0,0,0,0,0,0,0,0,0,0,0,0,0,0,0,0,0,0,0,0,0,0,0,0,0,0,0,0,0,0,0,0,0,0,0,0,0,0,0,0,0,0,0,0,0,0,0,0,0,0,0,0,0,0,0,0,0,0,0,0,0,0,0,0,0,0,0,0,0,0,0,0,0,0,0,0,0,0,0,0,0,0,0,0,0,0,0,0,0,0,0,0,0,0,0,0,0,0,0,0,0,0,0,0,0,0,0,0,0,0,0,0,0,0,0,0,0,0,0,0,0,0,0,0,0,0,0,0,0,0,0,0,0,0,0,0,0,0,0,0,0,0,0,0,0,0,0,0,0,0,0,0,0,0,0,0,0,0,0,0,0,0,0,0,0,0,0,0,0,0,0,0,0,0,0,0,0,0,0,0,0,0,0,0,0,0,0,0,0,0,0,0,0,0,0,0,0,0,0,0,0,0,0,0,0,0,0,0,0,0,0,0,0,0,0,0,0,0,0,0,0,0,0,0,0,0,0,0,0,0,0,0,0,0,0,0,0,0,0,0,0,0,0,0,0,0,0,0,0,0,0,0,0,0,0,0,0,0,0,0,0,0,0,0,0,0,0,0,0,0,0,0,0,0,0,0,0,0,0,0,0,0,0,0,0,0,0,0,0,0,0,0,0,0,0,0,0,0,0,0,0,0,0,0,0,0,0,0,0,0,0,0,0,0,0,0,0,0,0,0,0,0,0,0,0,0,0,0,0,0,0,0,0,0,0,0,0,0,0,0,0,0,0,0,0,0,0,0,0,0,0,0,0,0,0,0,0,0,0,0,0,0,0,0,0,0,0,0,0,0,0,0,0,0,0,0,0,0,0,0,0,0,0,0,0,0,0,0,0,0,0,0,0,0,0,0,0,0,0,0,0,0,0,0,0,0,0,0,0,0,0,0,0,0,0,0,0,0,0,0,0,0,0,0,0,0,0,0,0,0,0,0,0,0,0,0,0,0,0,0,0,0,0,0,0,0,0,0,0,0,0,0,0,0,0,0,0,0,0,0,0,0,0,0,0,0,0,0,0,0,0,0,0,0,0,0,0,0,0,0,0,0,0,0,0,0,0,0,0,0,0,0,0,0,0,0,0,0,0,0,0,0,0,0,0,0,0,0,0,0,0,0,0,0,0,0,0,0,0,0,0,0,0,0,0,0,0,0,0,0,0,0,0,0,0,0,0,0,0,0,0,0,0,0,0,0,0,0,0,0,0,0,0,0,0,0,0,0,0,0,0,0,0,0,0,0,0,0,0,0,0,0,0,0,0,0,0,0,0,0,0,0,0,0,0,0,0,0,0,0,0,0,0,0,0,0,0,0,0,0,0,0,0,0,0,0,0,0,0,0,0,0,0,0,0,0,0,0,0,0,0,0,0,0,0,0,0,0,0,0,0,0,0,0,0,0,0,0,0,0,0,0,0,0,0,0,0,0,0,0,0,0,0,0,0,0,0,0,0,0,0,0,0,0,0,0,0,0,0,0,0,0,0,0,0,0,0,0,0,0,0,0,0,0,0,0,0,0,0,0,0,0,0,0,0,0,0,0,0,0,0,0,0,0,0,0,0,0,0,0,0,0,0,0,0,0,0,0,0,0,0,0,0,0,0,0,0,0,0,0,0,0,0,0,0,0,0,0,0,0,0,0,0,0,0,0,0,0 ...(+27783 chars)]  distributed_mem=Block RAM  rst=off  init_reg=0  en=off  latency=1  gui_display_data_type=Floating-point  arith_type=Floating-point  n_bits=16  bin_pt=15  preci_type=Double  exp_width=8  frac_width=24  optimize=Area  use_rpm=on  simulation_type=fast_sim  XmcBlockStatus=1  maskContainerNames=tabcontainer1  block_type=sprom  block_config=sysgen:SPROM_config
  ROM3 : hdlBasic/ROM  depth=7874  initVector=[0,0,0,0,0,0,0,0,0,0,0,0,0,0,0,0,0,0,0,0,0,0,0,0,0,0,0,0,0,0,0,0,0,0,0,0,0,0,0,0,0,0,0,0,0,0,0,0,0,0,0,0,0,0,0,0,0,0,0,0,0,0,0,0,0,0,0,0,0,0,0,0,0,0,0,0,0,0,0,0,0,0,0,0,0,0,0,0,0,0,0,0,0,0,0,0,0,0,0,0,0,0,0,0,0,0,0,0,0,0,0,0,0,0,0,0,0,0,0,0,0,0,0,0,0,0,0,0,0,0,0,0,0,0,0,0,0,0,0,0,0,0,0,0,0,0,0,0,0,0,0,0,0,0,0,0,0,0,0,0,0,0,0,0,0,0,0,0,0,0,0,0,0,0,0,0,0,0,0,0,0,0,0,0,0,0,0,0,0,0,0,0,0,0,0,0,0,0,0,0,0,0,0,0,0,0,0,0,0,0,0,0,0,0,0,0,0,0,0,0,0,0,0,0,0,0,0,0,0,0,0,0,0,0,0,0,0,0,0,0,0,0,0,0,0,0,0,0,0,0,0,0,0,0,0,0,0,0,0,0,0,0,0,0,0,0,0,0,0,0,0,0,0,0,0,0,0,0,0,0,0,0,0,0,0,0,0,0,0,0,0,0,0,0,0,0,0,0,0,0,0,0,0,0,0,0,0,0,0,0,0,0,0,0,0,0,0,0,0,0,0,0,0,0,0,0,0,0,0,0,0,0,0,0,0,0,0,0,0,0,0,0,0,0,0,0,0,0,0,0,0,0,0,0,0,0,0,0,0,0,0,0,0,0,0,0,0,0,0,0,0,0,0,0,0,0,0,0,0,0,0,0,0,0,0,0,0,0,0,0,0,0,0,0,0,0,0,0,0,0,0,0,0,0,0,0,0,0,0,0,0,0,0,0,0,0,0,0,0,0,0,0,0,0,0,0,0,0,0,0,0,0,0,0,0,0,0,0,0,0,0,0,0,0,0,0,0,0,0,0,0,0,0,0,0,0,0,0,0,0,0,0,0,0,0,0,0,0,0,0,0,0,0,0,0,0,0,0,0,0,0,0,0,0,0,0,0,0,0,0,0,0,0,0,0,0,0,0,0,0,0,0,0,0,0,0,0,0,0,0,0,0,0,0,0,0,0,0,0,0,0,0,0,0,0,0,0,0,0,0,0,0,0,0,0,0,0,0,0,0,0,0,0,0,0,0,0,0,0,0,0,0,0,0,0,0,0,0,0,0,0,0,0,0,0,0,0,0,0,0,0,0,0,0,0,0,0,0,0,0,0,0,0,0,0,0,0,0,0,0,0,0,0,0,0,0,0,0,0,0,0,0,0,0,0,0,0,0,0,0,0,0,0,0,0,0,0,0,0,0,0,0,0,0,0,0,0,0,0,0,0,0,0,0,0,0,0,0,0,0,0,0,0,0,0,0,0,0,0,0,0,0,0,0,0,0,0,0,0,0,0,0,0,0,0,0,0,0,0,0,0,0,0,0,0,0,0,0,0,0,0,0,0,0,0,0,0,0,0,0,0,0,0,0,0,0,0,0,0,0,0,0,0,0,0,0,0,0,0,0,0,0,0,0,0,0,0,0,0,0,0,0,0,0,0,0,0,0,0,0,0,0,0,0,0,0,0,0,0,0,0,0,0,0,0,0,0,0,0,0,0,0,0,0,0,0,0,0,0,0,0,0,0,0,0,0,0,0,0,0,0,0,0,0,0,0,0,0,0,0,0,0,0,0,0,0,0,0,0,0,0,0,0,0,0,0,0,0,0,0,0,0,0,0,0,0,0,0,0,0,0,0,0,0,0,0,0,0,0,0,0,0,0,0,0,0,0,0,0,0,0,0,0,0,0,0,0,0,0,0,0,0,0,0,0,0,0,0,0,0,0,0,0,0,0,0,0,0,0,0,0,0,0,0,0,0,0,0,0,0,0,0,0,0,0,0,0,0,0,0,0,0,0,0,0,0,0,0,0,0,0,0,0,0,0,0,0,0,0,0,0,0,0,0,0,0,0,0,0,0,0,0,0,0,0,0,0,0,0,0,0,0,0,0,0,0,0,0,0,0,0,0,0,0,0,0,0,0,0,0,0,0,0,0,0,0,0,0,0,0,0,0,0,0,0,0,0,0,0,0,0,0,0,0,0,0,0,0,0,0,0,0,0,0,0,0,0,0,0,0,0,0,0,0,0,0,0,0,0,0,0,0,0,0,0,0,0,0,0,0,0,0,0,0,0,0,0,0,0,0,0,0,0,0,0,0,0,0,0,0,0,0,0,0,0,0,0,0,0,0,0,0,0,0,0,0,0,0,0,0,0,0,0,0,0,0,0,0,0,0,0,0,0,0,0,0,0,0,0,0,0,0,0,0,0,0,0,0,0,0,0,0,0,0,0,0,0,0,0,0,0,0,0,0,0,0,0,0,0,0,0,0,0,0,0,0,0,0,0,0,0,0,0,0,0,0,0,0,0,0,0,0,0,0,0,0,0,0,0,0,0,0,0,0,0,0,0,0,0,0,0,0,0,0,0,0,0,0,0,0,0,0,0,0,0,0,0,0,0,0,0,0,0,0,0,0,0,0,0,0,0,0,0,0,0,0,0,0,0,0,0,0,0,0,0,0,0,0,0,0,0,0,0,0,0,0,0,0,0,0,0,0,0,0,0,0,0,0,0,0,0,0,0,0,0,0,0,0,0,0,0,0,0,0,0,0,0,0,0,0,0,0,0,0,0,0,0,0,0,0,0,0,0,0,0,0,0,0,0,0,0,0,0,0,0,0,0,0,0,0,0,0,0,0,0,0,0,0,0,0,0,0,0,0,0,0,0,0,0,0,0,0,0,0,0,0,0,0,0,0,0,0,0,0,0,0,0,0,0,0,0,0,0,0,0,0,0,0,0,0,0,0,0,0,0,0,0,0,0,0,0,0,0,0,0,0,0,0,0,0,0,0,0,0,0,0,0,0,0,0,0,0,0,0,0,0,0,0,0,0,0,0,0,0,0,0,0,0,0,0,0,0,0,0,0,0,0,0,0,0,0,0,0,0,0,0,0,0,0,0,0,0,0,0,0,0,0,0,0,0,0,0,0,0,0,0,0,0,0,0,0,0,0,0,0,0,0,0,0,0,0,0,0,0,0,0,0,0,0,0,0,0,0,0,0,0,0,0,0,0,0,0,0,0,0,0,0,0,0,0,0,0,0,0,0,0,0,0,0,0,0,0,0,0,0,0,0,0,0,0,0,0,0,0,0,0,0,0,0,0,0,0,0,0,0,0,0,0,0,0,0,0,0,0,0,0,0,0,0,0,0,0,0,0,0,0,0,0,0,0,0,0,0,0,0,0,0,0,0,0,0,0,0,0,0,0,0,0,0,0,0,0,0,0,0,0,0,0,0,0,0,0,0,0,0,0,0,0,0,0,0,0,0,0,0,0,0,0,0,0,0,0,0,0,0,0,0,0,0,0,0,0,0,0,0,0,0,0,0,0,0,0,0,0,0,0,0,0,0,0,0,0,0,0,0,0,0,0,0,0,0,0,0,0,0,0,0,0,0,0,0,0,0,0,0,0,0,0,0,0,0,0,0,0,0,0,0,0,0,0,0,0,0,0,0,0,0,0,0,0,0,0,0,0,0,0,0,0,0,0,0,0,0,0,0,0,0,0,0,0,0,0,0,0,0,0,0,0,0,0,0,0,0,0,0,0,0,0,0,0,0,0,0,0,0,0,0,0,0,0,0,0,0,0,0,0,0,0,0,0,0,0,0,0,0,0,0,0,0,0,0,0,0,0,0,0,0,0,0,0,0,0,0,0,0,0,0,0,0,0,0,0,0,0,0,0,0,0,0,0,0,0,0,0,0,0,0,0,0,0,0,0,0,0,0,0,0,0,0,0,0,0,0,0,0,0,0,0,0,0,0,0,0,0,0,0,0,0,0,0,0,0,0,0,0,0,0,0,0,0,0,0,0,0,0,0,0,0,0,0,0,0,0,0,0,0,0,0,0,0,0,0,0,0,0,0,0,0,0,0,0,0,0,0,0,0,0,0,0,0,0,0,0,0,0,0,0,0,0,0,0,0,0,0,0,0,0,0,0,0,0,0,0,0,0,0,0,0,0,0,0,0,0,0,0,0,0,0,0,0,0,0,0,0,0,0,0,0,0,0,0,0,0,0,0,0,0,0,0,0,0,0,0,0,0,0,0,0,0,0,0,0,0,0,0,0,0,0,0,0,0,0,0,0,0,0,0,0,0,0,0,0,0,0,0,0,0,0,0,0,0,0,0,0,0,0,0,0,0,0,0,0,0,0,0,0,0,0,0,0,0,0,0,0,0,0,0,0,0,0,0,0,0,0,0,0,0,0,0,0,0,0,0,0,0,0,0,0,0,0,0,0,0,0,0,0,0,0,0,0,0,0,0,0,0,0,0,0,0,0,0,0,0,0,0,0,0,0,0,0,0,0,0,0,0,0,0,0,0 ...(+27701 chars)]  distributed_mem=Block RAM  rst=off  init_reg=0  en=off  latency=1  gui_display_data_type=Floating-point  arith_type=Floating-point  n_bits=16  bin_pt=15  preci_type=Double  exp_width=8  frac_width=24  optimize=Area  use_rpm=on  simulation_type=fast_sim  XmcBlockStatus=1  maskContainerNames=tabcontainer1  block_type=sprom  block_config=sysgen:SPROM_config
  ROM4 : hdlBasic/ROM  depth=7874  initVector=[0,0,0,0,0,0,0,0,0,0,0,0,0,0,0,0,0,0,0,0,0,0,0,0,0,0,0,0,0,0,0,0,0,0,0,0,0,0,0,0,0,0,0,0,0,0,0,0,0,0,0,0,0,0,0,0,0,0,0,0,0,0,0,0,0,0,0,0,0,0,0,0,0,0,0,0,0,0,0,0,0,0,0,0,0,0,0,0,0,0,0,0,0,0,0,0,0,0,0,0,0,0,0,0,0,0,0,0,0,0,0,0,0,0,0,0,0,0,0,0,0,0,0,0,0,0,0,0,0,0,0,0,0,0,0,0,0,0,0,0,0,0,0,0,0,0,0,0,0,0,0,0,0,0,0,0,0,0,0,0,0,0,0,0,0,0,0,0,0,0,0,0,0,0,0,0,0,0,0,0,0,0,0,0,0,0,0,0,0,0,0,0,0,0,0,0,0,0,0,0,0,0,0,0,0,0,0,0,0,0,0,0,0,0,0,0,0,0,0,0,0,0,0,0,0,0,0,0,0,0,0,0,0,0,0,0,0,0,0,0,0,0,0,0,0,0,0,0,0,0,0,0,0,0,0,0,0,0,0,0,0,0,0,0,0,0,0,0,0,0,0,0,0,0,0,0,0,0,0,0,0,0,0,0,0,0,0,0,0,0,0,0,0,0,0,0,0,0,0,0,0,0,0,0,0,0,0,0,0,0,0,0,0,0,0,0,0,0,0,0,0,0,0,0,0,0,0,0,0,0,0,0,0,0,0,0,0,0,0,0,0,0,0,0,0,0,0,0,0,0,0,0,0,0,0,0,0,0,0,0,0,0,0,0,0,0,0,0,0,0,0,0,0,0,0,0,0,0,0,0,0,0,0,0,0,0,0,0,0,0,0,0,0,0,0,0,0,0,0,0,0,0,0,0,0,0,0,0,0,0,0,0,0,0,0,0,0,0,0,0,0,0,0,0,0,0,0,0,0,0,0,0,0,0,0,0,0,0,0,0,0,0,0,0,0,0,0,0,0,0,0,0,0,0,0,0,0,0,0,0,0,0,0,0,0,0,0,0,0,0,0,0,0,0,0,0,0,0,0,0,0,0,0,0,0,0,0,0,0,0,0,0,0,0,0,0,0,0,0,0,0,0,0,0,0,0,0,0,0,0,0,0,0,0,0,0,0,0,0,0,0,0,0,0,0,0,0,0,0,0,0,0,0,0,0,0,0,0,0,0,0,0,0,0,0,0,0,0,0,0,0,0,0,0,0,0,0,0,0,0,0,0,0,0,0,0,0,0,0,0,0,0,0,0,0,0,0,0,0,0,0,0,0,0,0,0,0,0,0,0,0,0,0,0,0,0,0,0,0,0,0,0,0,0,0,0,0,0,0,0,0,0,0,0,0,0,0,0,0,0,0,0,0,0,0,0,0,0,0,0,0,0,0,0,0,0,0,0,0,0,0,0,0,0,0,0,0,0,0,0,0,0,0,0,0,0,0,0,0,0,0,0,0,0,0,0,0,0,0,0,0,0,0,0,0,0,0,0,0,0,0,0,0,0,0,0,0,0,0,0,0,0,0,0,0,0,0,0,0,0,0,0,0,0,0,0,0,0,0,0,0,0,0,0,0,0,0,0,0,0,0,0,0,0,0,0,0,0,0,0,0,0,0,0,0,0,0,0,0,0,0,0,0,0,0,0,0,0,0,0,0,0,0,0,0,0,0,0,0,0,0,0,0,0,0,0,0,0,0,0,0,0,0,0,0,0,0,0,0,0,0,0,0,0,0,0,0,0,0,0,0,0,0,0,0,0,0,0,0,0,0,0,0,0,0,0,0,0,0,0,0,0,0,0,0,0,0,0,0,0,0,0,0,0,0,0,0,0,0,0,0,0,0,0,0,0,0,0,0,0,0,0,0,0,0,0,0,0,0,0,0,0,0,0,0,0,0,0,0,0,0,0,0,0,0,0,0,0,0,0,0,0,0,0,0,0,0,0,0,0,0,0,0,0,0,0,0,0,0,0,0,0,0,0,0,0,0,0,0,0,0,0,0,0,0,0,0,0,0,0,0,0,0,0,0,0,0,0,0,0,0,0,0,0,0,0,0,0,0,0,0,0,0,0,0,0,0,0,0,0,0,0,0,0,0,0,0,0,0,0,0,0,0,0,0,0,0,0,0,0,0,0,0,0,0,0,0,0,0,0,0,0,0,0,0,0,0,0,0,0,0,0,0,0,0,0,0,0,0,0,0,0,0,0,0,0,0,0,0,0,0,0,0,0,0,0,0,0,0,0,0,0,0,0,0,0,0,0,0,0,0,0,0,0,0,0,0,0,0,0,0,0,0,0,0,0,0,0,0,0,0,0,0,0,0,0,0,0,0,0,0,0,0,0,0,0,0,0,0,0,0,0,0,0,0,0,0,0,0,0,0,0,0,0,0,0,0,0,0,0,0,0,0,0,0,0,0,0,0,0,0,0,0,0,0,0,0,0,0,0,0,0,0,0,0,0,0,0,0,0,0,0,0,0,0,0,0,0,0,0,0,0,0,0,0,0,0,0,0,0,0,0,0,0,0,0,0,0,0,0,0,0,0,0,0,0,0,0,0,0,0,0,0,0,0,0,0,0,0,0,0,0,0,0,0,0,0,0,0,0,0,0,0,0,0,0,0,0,0,0,0,0,0,0,0,0,0,0,0,0,0,0,0,0,0,0,0,0,0,0,0,0,0,0,0,0,0,0,0,0,0,0,0,0,0,0,0,0,0,0,0,0,0,0,0,0,0,0,0,0,0,0,0,0,0,0,0,0,0,0,0,0,0,0,0,0,0,0,0,0,0,0,0,0,0,0,0,0,0,0,0,0,0,0,0,0,0,0,0,0,0,0,0,0,0,0,0,0,0,0,0,0,0,0,0,0,0,0,0,0,0,0,0,0,0,0,0,0,0,0,0,0,0,0,0,0,0,0,0,0,0,0,0,0,0,0,0,0,0,0,0,0,0,0,0,0,0,0,0,0,0,0,0,0,0,0,0,0,0,0,0,0,0,0,0,0,0,0,0,0,0,0,0,0,0,0,0,0,0,0,0,0,0,0,0,0,0,0,0,0,0,0,0,0,0,0,0,0,0,0,0,0,0,0,0,0,0,0,0,0,0,0,0,0,0,0,0,0,0,0,0,0,0,0,0,0,0,0,0,0,0,0,0,0,0,0,0,0,0,0,0,0,0,0,0,0,0,0,0,0,0,0,0,0,0,0,0,0,0,0,0,0,0,0,0,0,0,0,0,0,0,0,0,0,0,0,0,0,0,0,0,0,0,0,0,0,0,0,0,0,0,0,0,0,0,0,0,0,0,0,0,0,0,0,0,0,0,0,0,0,0,0,0,0,0,0,0,0,0,0,0,0,0,0,0,0,0,0,0,0,0,0,0,0,0,0,0,0,0,0,0,0,0,0,0,0,0,0,0,0,0,0,0,0,0,0,0,0,0,0,0,0,0,0,0,0,0,0,0,0,0,0,0,0,0,0,0,0,0,0,0,0,0,0,0,0,0,0,0,0,0,0,0,0,0,0,0,0,0,0,0,0,0,0,0,0,0,0,0,0,0,0,0,0,0,0,0,0,0,0,0,0,0,0,0,0,0,0,0,0,0,0,0,0,0,0,0,0,0,0,0,0,0,0,0,0,0,0,0,0,0,0,0,0,0,0,0,0,0,0,0,0,0,0,0,0,0,0,0,0,0,0,0,0,0,0,0,0,0,0,0,0,0,0,0,0,0,0,0,0,0,0,0,0,0,0,0,0,0,0,0,0,0,0,0,0,0,0,0,0,0,0,0,0,0,0,0,0,0,0,0,0,0,0,0,0,0,0,0,0,0,0,0,0,0,0,0,0,0,0,0,0,0,0,0,0,0,0,0,0,0,0,0,0,0,0,0,0,0,0,0,0,0,0,0,0,0,0,0,0,0,0,0,0,0,0,0,0,0,0,0,0,0,0,0,0,0,0,0,0,0,0,0,0,0,0,0,0,0,0,0,0,0,0,0,0,0,0,0,0,0,0,0,0,0,0,0,0,0,0,0,0,0,0,0,0,0,0,0,0,0,0,0,0,0,0,0,0,0,0,0,0,0,0,0,0,0,0,0,0,0,0,0,0,0,0,0,0,0,0,0,0,0,0,0,0,0,0,0,0,0,0,0,0,0,0,0,0,0,0,0,0,0,0,0,0,0,0,0,0,0,0,0,0,0,0,0,0,0,0,0,0,0,0,0,0,0,0,0,0,0,0,0,0,0,0,0,0,0,0,0,0,0,0,0,0,0,0,0,0,0,0,0,0,0,0,0,0,0,0,0,0,0,0,0,0,0,0,0,0,0,0,0,0,0,0,0,0,0,0,0,0,0,0,0,0,0,0,0,0,0,0,0,0,0,0,0,0,0,0,0,0,0,0,0,0,0,0,0,0,0,0,0,0,0,0,0,0,0,0,0,0,0,0,0,0,0,0,0,0,0,0,0,0,0,0,0,0,0 ...(+27645 chars)]  distributed_mem=Block RAM  rst=off  init_reg=0  en=off  latency=1  gui_display_data_type=Floating-point  arith_type=Floating-point  n_bits=16  bin_pt=15  preci_type=Double  exp_width=8  frac_width=24  optimize=Area  use_rpm=on  simulation_type=fast_sim  XmcBlockStatus=1  maskContainerNames=tabcontainer1  block_type=sprom  block_config=sysgen:SPROM_config
  ROM5 : hdlBasic/ROM  depth=7874  initVector=[0,0,0,0,0,0,0,0,0,0,0,0,0,0,0,0,0,0,0,0,0,0,0,0,0,0,0,0,0,0,0,0,0,0,0,0,0,0,0,0,0,0,0,0,0,0,0,0,0,0,0,0,0,0,0,0,0,0,0,0,0,0,0,0,0,0,0,0,0,0,0,0,0,0,0,0,0,0,0,0,0,0,0,0,0,0,0,0,0,0,0,0,0,0,0,0,0,0,0,0,0,0,0,0,0,0,0,0,0,0,0,0,0,0,0,0,0,0,0,0,0,0,0,0,0,0,0,0,0,0,0,0,0,0,0,0,0,0,0,0,0,0,0,0,0,0,0,0,0,0,0,0,0,0,0,0,0,0,0,0,0,0,0,0,0,0,0,0,0,0,0,0,0,0,0,0,0,0,0,0,0,0,0,0,0,0,0,0,0,0,0,0,0,0,0,0,0,0,0,0,0,0,0,0,0,0,0,0,0,0,0,0,0,0,0,0,0,0,0,0,0,0,0,0,0,0,0,0,0,0,0,0,0,0,0,0,0,0,0,0,0,0,0,0,0,0,0,0,0,0,0,0,0,0,0,0,0,0,0,0,0,0,0,0,0,0,0,0,0,0,0,0,0,0,0,0,0,0,0,0,0,0,0,0,0,0,0,0,0,0,0,0,0,0,0,0,0,0,0,0,0,0,0,0,0,0,0,0,0,0,0,0,0,0,0,0,0,0,0,0,0,0,0,0,0,0,0,0,0,0,0,0,0,0,0,0,0,0,0,0,0,0,0,0,0,0,0,0,0,0,0,0,0,0,0,0,0,0,0,0,0,0,0,0,0,0,0,0,0,0,0,0,0,0,0,0,0,0,0,0,0,0,0,0,0,0,0,0,0,0,0,0,0,0,0,0,0,0,0,0,0,0,0,0,0,0,0,0,0,0,0,0,0,0,0,0,0,0,0,0,0,0,0,0,0,0,0,0,0,0,0,0,0,0,0,0,0,0,0,0,0,0,0,0,0,0,0,0,0,0,0,0,0,0,0,0,0,0,0,0,0,0,0,0,0,0,0,0,0,0,0,0,0,0,0,0,0,0,0,0,0,0,0,0,0,0,0,0,0,0,0,0,0,0,0,0,0,0,0,0,0,0,0,0,0,0,0,0,0,0,0,0,0,0,0,0,0,0,0,0,0,0,0,0,0,0,0,0,0,0,0,0,0,0,0,0,0,0,0,0,0,0,0,0,0,0,0,0,0,0,0,0,0,0,0,0,0,0,0,0,0,0,0,0,0,0,0,0,0,0,0,0,0,0,0,0,0,0,0,0,0,0,0,0,0,0,0,0,0,0,0,0,0,0,0,0,0,0,0,0,0,0,0,0,0,0,0,0,0,0,0,0,0,0,0,0,0,0,0,0,0,0,0,0,0,0,0,0,0,0,0,0,0,0,0,0,0,0,0,0,0,0,0,0,0,0,0,0,0,0,0,0,0,0,0,0,0,0,0,0,0,0,0,0,0,0,0,0,0,0,0,0,0,0,0,0,0,0,0,0,0,0,0,0,0,0,0,0,0,0,0,0,0,0,0,0,0,0,0,0,0,0,0,0,0,0,0,0,0,0,0,0,0,0,0,0,0,0,0,0,0,0,0,0,0,0,0,0,0,0,0,0,0,0,0,0,0,0,0,0,0,0,0,0,0,0,0,0,0,0,0,0,0,0,0,0,0,0,0,0,0,0,0,0,0,0,0,0,0,0,0,0,0,0,0,0,0,0,0,0,0,0,0,0,0,0,0,0,0,0,0,0,0,0,0,0,0,0,0,0,0,0,0,0,0,0,0,0,0,0,0,0,0,0,0,0,0,0,0,0,0,0,0,0,0,0,0,0,0,0,0,0,0,0,0,0,0,0,0,0,0,0,0,0,0,0,0,0,0,0,0,0,0,0,0,0,0,0,0,0,0,0,0,0,0,0,0,0,0,0,0,0,0,0,0,0,0,0,0,0,0,0,0,0,0,0,0,0,0,0,0,0,0,0,0,0,0,0,0,0,0,0,0,0,0,0,0,0,0,0,0,0,0,0,0,0,0,0,0,0,0,0,0,0,0,0,0,0,0,0,0,0,0,0,0,0,0,0,0,0,0,0,0,0,0,0,0,0,0,0,0,0,0,0,0,0,0,0,0,0,0,0,0,0,0,0,0,0,0,0,0,0,0,0,0,0,0,0,0,0,0,0,0,0,0,0,0,0,0,0,0,0,0,0,0,0,0,0,0,0,0,0,0,0,0,0,0,0,0,0,0,0,0,0,0,0,0,0,0,0,0,0,0,0,0,0,0,0,0,0,0,0,0,0,0,0,0,0,0,0,0,0,0,0,0,0,0,0,0,0,0,0,0,0,0,0,0,0,0,0,0,0,0,0,0,0,0,0,0,0,0,0,0,0,0,0,0,0,0,0,0,0,0,0,0,0,0,0,0,0,0,0,0,0,0,0,0,0,0,0,0,0,0,0,0,0,0,0,0,0,0,0,0,0,0,0,0,0,0,0,0,0,0,0,0,0,0,0,0,0,0,0,0,0,0,0,0,0,0,0,0,0,0,0,0,0,0,0,0,0,0,0,0,0,0,0,0,0,0,0,0,0,0,0,0,0,0,0,0,0,0,0,0,0,0,0,0,0,0,0,0,0,0,0,0,0,0,0,0,0,0,0,0,0,0,0,0,0,0,0,0,0,0,0,0,0,0,0,0,0,0,0,0,0,0,0,0,0,0,0,0,0,0,0,0,0,0,0,0,0,0,0,0,0,0,0,0,0,0,0,0,0,0,0,0,0,0,0,0,0,0,0,0,0,0,0,0,0,0,0,0,0,0,0,0,0,0,0,0,0,0,0,0,0,0,0,0,0,0,0,0,0,0,0,0,0,0,0,0,0,0,0,0,0,0,0,0,0,0,0,0,0,0,0,0,0,0,0,0,0,0,0,0,0,0,0,0,0,0,0,0,0,0,0,0,0,0,0,0,0,0,0,0,0,0,0,0,0,0,0,0,0,0,0,0,0,0,0,0,0,0,0,0,0,0,0,0,0,0,0,0,0,0,0,0,0,0,0,0,0,0,0,0,0,0,0,0,0,0,0,0,0,0,0,0,0,0,0,0,0,0,0,0,0,0,0,0,0,0,0,0,0,0,0,0,0,0,0,0,0,0,0,0,0,0,0,0,0,0,0,0,0,0,0,0,0,0,0,0,0,0,0,0,0,0,0,0,0,0,0,0,0,0,0,0,0,0,0,0,0,0,0,0,0,0,0,0,0,0,0,0,0,0,0,0,0,0,0,0,0,0,0,0,0,0,0,0,0,0,0,0,0,0,0,0,0,0,0,0,0,0,0,0,0,0,0,0,0,0,0,0,0,0,0,0,0,0,0,0,0,0,0,0,0,0,0,0,0,0,0,0,0,0,0,0,0,0,0,0,0,0,0,0,0,0,0,0,0,0,0,0,0,0,0,0,0,0,0,0,0,0,0,0,0,0,0,0,0,0,0,0,0,0,0,0,0,0,0,0,0,0,0,0,0,0,0,0,0,0,0,0,0,0,0,0,0,0,0,0,0,0,0,0,0,0,0,0,0,0,0,0,0,0,0,0,0,0,0,0,0,0,0,0,0,0,0,0,0,0,0,0,0,0,0,0,0,0,0,0,0,0,0,0,0,0,0,0,0,0,0,0,0,0,0,0,0,0,0,0,0,0,0,0,0,0,0,0,0,0,0,0,0,0,0,0,0,0,0,0,0,0,0,0,0,0,0,0,0,0,0,0,0,0,0,0,0,0,0,0,0,0,0,0,0,0,0,0,0,0,0,0,0,0,0,0,0,0,0,0,0,0,0,0,0,0,0,0,0,0,0,0,0,0,0,0,0,0,0,0,0,0,0,0,0,0,0,0,0,0,0,0,0,0,0,0,0,0,0,0,0,0,0,0,0,0,0,0,0,0,0,0,0,0,0,0,0,0,0,0,0,0,0,0,0,0,0,0,0,0,0,0,0,0,0,0,0,0,0,0,0,0,0,0,0,0,0,0,0,0,0,0,0,0,0,0,0,0,0,0,0,0,0,0,0,0,0,0,0,0,0,0,0,0,0,0,0,0,0,0,0,0,0,0,0,0,0,0,0,0,0,0,0,0,0,0,0,0,0,0,0,0,0,0,0,0,0,0,0,0,0,0,0,0,0,0,0,0,0,0,0,0,0,0,0,0,0,0,0,0,0,0,0,0,0,0,0,0,0,0,0,0,0,0,0,0,0,0,0,0,0,0,0,0,0,0,0,0,0,0,0,0,0,0,0,0,0,0,0,0,0,0,0,0,0,0,0,0,0,0,0,0,0,0,0,0,0,0,0,0,0,0,0,0,0,0,0,0,0,0,0,0,0,0,0,0,0,0,0,0,0,0,0,0,0,0,0,0,0,0,0,0,0,0,0,0,0,0,0,0,0,0,0,0,0,0,0,0,0,0,0,0,0,0,0,0,0,0,0,0 ...(+27581 chars)]  distributed_mem=Block RAM  rst=off  init_reg=0  en=off  latency=1  gui_display_data_type=Floating-point  arith_type=Floating-point  n_bits=16  bin_pt=15  preci_type=Double  exp_width=8  frac_width=24  optimize=Area  use_rpm=on  simulation_type=fast_sim  XmcBlockStatus=1  maskContainerNames=tabcontainer1  block_type=sprom  block_config=sysgen:SPROM_config
  ROM6 : hdlBasic/ROM  depth=7874  initVector=[0,0,0,0,0,0,0,0,0,0,0,0,0,0,0,0,0,0,0,0,0,0,0,0,0,0,0,0,0,0,0,0,0,0,0,0,0,0,0,0,0,0,0,0,0,0,0,0,0,0,0,0,0,0,0,0,0,0,0,0,0,0,0,0,0,0,0,0,0,0,0,0,0,0,0,0,0,0,0,0,0,0,0,0,0,0,0,0,0,0,0,0,0,0,0,0,0,0,0,0,0,0,0,0,0,0,0,0,0,0,0,0,0,0,0,0,0,0,0,0,0,0,0,0,0,0,0,0,0,0,0,0,0,0,0,0,0,0,0,0,0,0,0,0,0,0,0,0,0,0,0,0,0,0,0,0,0,0,0,0,0,0,0,0,0,0,0,0,0,0,0,0,0,0,0,0,0,0,0,0,0,0,0,0,0,0,0,0,0,0,0,0,0,0,0,0,0,0,0,0,0,0,0,0,0,0,0,0,0,0,0,0,0,0,0,0,0,0,0,0,0,0,0,0,0,0,0,0,0,0,0,0,0,0,0,0,0,0,0,0,0,0,0,0,0,0,0,0,0,0,0,0,0,0,0,0,0,0,0,0,0,0,0,0,0,0,0,0,0,0,0,0,0,0,0,0,0,0,0,0,0,0,0,0,0,0,0,0,0,0,0,0,0,0,0,0,0,0,0,0,0,0,0,0,0,0,0,0,0,0,0,0,0,0,0,0,0,0,0,0,0,0,0,0,0,0,0,0,0,0,0,0,0,0,0,0,0,0,0,0,0,0,0,0,0,0,0,0,0,0,0,0,0,0,0,0,0,0,0,0,0,0,0,0,0,0,0,0,0,0,0,0,0,0,0,0,0,0,0,0,0,0,0,0,0,0,0,0,0,0,0,0,0,0,0,0,0,0,0,0,0,0,0,0,0,0,0,0,0,0,0,0,0,0,0,0,0,0,0,0,0,0,0,0,0,0,0,0,0,0,0,0,0,0,0,0,0,0,0,0,0,0,0,0,0,0,0,0,0,0,0,0,0,0,0,0,0,0,0,0,0,0,0,0,0,0,0,0,0,0,0,0,0,0,0,0,0,0,0,0,0,0,0,0,0,0,0,0,0,0,0,0,0,0,0,0,0,0,0,0,0,0,0,0,0,0,0,0,0,0,0,0,0,0,0,0,0,0,0,0,0,0,0,0,0,0,0,0,0,0,0,0,0,0,0,0,0,0,0,0,0,0,0,0,0,0,0,0,0,0,0,0,0,0,0,0,0,0,0,0,0,0,0,0,0,0,0,0,0,0,0,0,0,0,0,0,0,0,0,0,0,0,0,0,0,0,0,0,0,0,0,0,0,0,0,0,0,0,0,0,0,0,0,0,0,0,0,0,0,0,0,0,0,0,0,0,0,0,0,0,0,0,0,0,0,0,0,0,0,0,0,0,0,0,0,0,0,0,0,0,0,0,0,0,0,0,0,0,0,0,0,0,0,0,0,0,0,0,0,0,0,0,0,0,0,0,0,0,0,0,0,0,0,0,0,0,0,0,0,0,0,0,0,0,0,0,0,0,0,0,0,0,0,0,0,0,0,0,0,0,0,0,0,0,0,0,0,0,0,0,0,0,0,0,0,0,0,0,0,0,0,0,0,0,0,0,0,0,0,0,0,0,0,0,0,0,0,0,0,0,0,0,0,0,0,0,0,0,0,0,0,0,0,0,0,0,0,0,0,0,0,0,0,0,0,0,0,0,0,0,0,0,0,0,0,0,0,0,0,0,0,0,0,0,0,0,0,0,0,0,0,0,0,0,0,0,0,0,0,0,0,0,0,0,0,0,0,0,0,0,0,0,0,0,0,0,0,0,0,0,0,0,0,0,0,0,0,0,0,0,0,0,0,0,0,0,0,0,0,0,0,0,0,0,0,0,0,0,0,0,0,0,0,0,0,0,0,0,0,0,0,0,0,0,0,0,0,0,0,0,0,0,0,0,0,0,0,0,0,0,0,0,0,0,0,0,0,0,0,0,0,0,0,0,0,0,0,0,0,0,0,0,0,0,0,0,0,0,0,0,0,0,0,0,0,0,0,0,0,0,0,0,0,0,0,0,0,0,0,0,0,0,0,0,0,0,0,0,0,0,0,0,0,0,0,0,0,0,0,0,0,0,0,0,0,0,0,0,0,0,0,0,0,0,0,0,0,0,0,0,0,0,0,0,0,0,0,0,0,0,0,0,0,0,0,0,0,0,0,0,0,0,0,0,0,0,0,0,0,0,0,0,0,0,0,0,0,0,0,0,0,0,0,0,0,0,0,0,0,0,0,0,0,0,0,0,0,0,0,0,0,0,0,0,0,0,0,0,0,0,0,0,0,0,0,0,0,0,0,0,0,0,0,0,0,0,0,0,0,0,0,0,0,0,0,0,0,0,0,0,0,0,0,0,0,0,0,0,0,0,0,0,0,0,0,0,0,0,0,0,0,0,0,0,0,0,0,0,0,0,0,0,0,0,0,0,0,0,0,0,0,0,0,0,0,0,0,0,0,0,0,0,0,0,0,0,0,0,0,0,0,0,0,0,0,0,0,0,0,0,0,0,0,0,0,0,0,0,0,0,0,0,0,0,0,0,0,0,0,0,0,0,0,0,0,0,0,0,0,0,0,0,0,0,0,0,0,0,0,0,0,0,0,0,0,0,0,0,0,0,0,0,0,0,0,0,0,0,0,0,0,0,0,0,0,0,0,0,0,0,0,0,0,0,0,0,0,0,0,0,0,0,0,0,0,0,0,0,0,0,0,0,0,0,0,0,0,0,0,0,0,0,0,0,0,0,0,0,0,0,0,0,0,0,0,0,0,0,0,0,0,0,0,0,0,0,0,0,0,0,0,0,0,0,0,0,0,0,0,0,0,0,0,0,0,0,0,0,0,0,0,0,0,0,0,0,0,0,0,0,0,0,0,0,0,0,0,0,0,0,0,0,0,0,0,0,0,0,0,0,0,0,0,0,0,0,0,0,0,0,0,0,0,0,0,0,0,0,0,0,0,0,0,0,0,0,0,0,0,0,0,0,0,0,0,0,0,0,0,0,0,0,0,0,0,0,0,0,0,0,0,0,0,0,0,0,0,0,0,0,0,0,0,0,0,0,0,0,0,0,0,0,0,0,0,0,0,0,0,0,0,0,0,0,0,0,0,0,0,0,0,0,0,0,0,0,0,0,0,0,0,0,0,0,0,0,0,0,0,0,0,0,0,0,0,0,0,0,0,0,0,0,0,0,0,0,0,0,0,0,0,0,0,0,0,0,0,0,0,0,0,0,0,0,0,0,0,0,0,0,0,0,0,0,0,0,0,0,0,0,0,0,0,0,0,0,0,0,0,0,0,0,0,0,0,0,0,0,0,0,0,0,0,0,0,0,0,0,0,0,0,0,0,0,0,0,0,0,0,0,0,0,0,0,0,0,0,0,0,0,0,0,0,0,0,0,0,0,0,0,0,0,0,0,0,0,0,0,0,0,0,0,0,0,0,0,0,0,0,0,0,0,0,0,0,0,0,0,0,0,0,0,0,0,0,0,0,0,0,0,0,0,0,0,0,0,0,0,0,0,0,0,0,0,0,0,0,0,0,0,0,0,0,0,0,0,0,0,0,0,0,0,0,0,0,0,0,0,0,0,0,0,0,0,0,0,0,0,0,0,0,0,0,0,0,0,0,0,0,0,0,0,0,0,0,0,0,0,0,0,0,0,0,0,0,0,0,0,0,0,0,0,0,0,0,0,0,0,0,0,0,0,0,0,0,0,0,0,0,0,0,0,0,0,0,0,0,0,0,0,0,0,0,0,0,0,0,0,0,0,0,0,0,0,0,0,0,0,0,0,0,0,0,0,0,0,0,0,0,0,0,0,0,0,0,0,0,0,0,0,0,0,0,0,0,0,0,0,0,0,0,0,0,0,0,0,0,0,0,0,0,0,0,0,0,0,0,0,0,0,0,0,0,0,0,0,0,0,0,0,0,0,0,0,0,0,0,0,0,0,0,0,0,0,0,0,0,0,0,0,0,0,0,0,0,0,0,0,0,0,0,0,0,0,0,0,0,0,0,0,0,0,0,0,0,0,0,0,0,0,0,0,0,0,0,0,0,0,0,0,0,0,0,0,0,0,0,0,0,0,0,0,0,0,0,0,0,0,0,0,0,0,0,0,0,0,0,0,0,0,0,0,0,0,0,0,0,0,0,0,0,0,0,0,0,0,0,0,0,0,0,0,0,0,0,0,0,0,0,0,0,0,0,0,0,0,0,0,0,0,0,0,0,0,0,0,0,0,0,0,0,0,0,0,0,0,0,0,0,0,0,0,0,0,0,0,0,0,0,0,0,0,0,0,0,0,0,0,0,0,0,0,0,0,0,0,0,0,0,0,0,0,0,0,0,0,0,0,0,0,0,0,0,0,0,0,0,0,0,0,0,0,0,0,0,0,0,0,0,0,0,0,0,0,0,0,0,0,0,0,0,0,0,0,0,0,0,0,0 ...(+27379 chars)]  distributed_mem=Block RAM  rst=off  init_reg=0  en=off  latency=1  gui_display_data_type=Floating-point  arith_type=Floating-point  n_bits=16  bin_pt=15  preci_type=Double  exp_width=8  frac_width=24  optimize=Area  use_rpm=on  simulation_type=fast_sim  XmcBlockStatus=1  maskContainerNames=tabcontainer1  block_type=sprom  block_config=sysgen:SPROM_config
  ROM7 : hdlBasic/ROM  depth=7874  initVector=[0,0,0,0,0,0,0,0,0,0,0,0,0,0,0,0,0,0,0,0,0,0,0,0,0,0,0,0,0,0,0,0,0,0,0,0,0,0,0,0,0,0,0,0,0,0,0,0,0,0,0,0,0,0,0,0,0,0,0,0,0,0,0,0,0,0,0,0,0,0,0,0,0,0,0,0,0,0,0,0,0,0,0,0,0,0,0,0,0,0,0,0,0,0,0,0,0,0,0,0,0,0,0,0,0,0,0,0,0,0,0,0,0,0,0,0,0,0,0,0,0,0,0,0,0,0,0,0,0,0,0,0,0,0,0,0,0,0,0,0,0,0,0,0,0,0,0,0,0,0,0,0,0,0,0,0,0,0,0,0,0,0,0,0,0,0,0,0,0,0,0,0,0,0,0,0,0,0,0,0,0,0,0,0,0,0,0,0,0,0,0,0,0,0,0,0,0,0,0,0,0,0,0,0,0,0,0,0,0,0,0,0,0,0,0,0,0,0,0,0,0,0,0,0,0,0,0,0,0,0,0,0,0,0,0,0,0,0,0,0,0,0,0,0,0,0,0,0,0,0,0,0,0,0,0,0,0,0,0,0,0,0,0,0,0,0,0,0,0,0,0,0,0,0,0,0,0,0,0,0,0,0,0,0,0,0,0,0,0,0,0,0,0,0,0,0,0,0,0,0,0,0,0,0,0,0,0,0,0,0,0,0,0,0,0,0,0,0,0,0,0,0,0,0,0,0,0,0,0,0,0,0,0,0,0,0,0,0,0,0,0,0,0,0,0,0,0,0,0,0,0,0,0,0,0,0,0,0,0,0,0,0,0,0,0,0,0,0,0,0,0,0,0,0,0,0,0,0,0,0,0,0,0,0,0,0,0,0,0,0,0,0,0,0,0,0,0,0,0,0,0,0,0,0,0,0,0,0,0,0,0,0,0,0,0,0,0,0,0,0,0,0,0,0,0,0,0,0,0,0,0,0,0,0,0,0,0,0,0,0,0,0,0,0,0,0,0,0,0,0,0,0,0,0,0,0,0,0,0,0,0,0,0,0,0,0,0,0,0,0,0,0,0,0,0,0,0,0,0,0,0,0,0,0,0,0,0,0,0,0,0,0,0,0,0,0,0,0,0,0,0,0,0,0,0,0,0,0,0,0,0,0,0,0,0,0,0,0,0,0,0,0,0,0,0,0,0,0,0,0,0,0,0,0,0,0,0,0,0,0,0,0,0,0,0,0,0,0,0,0,0,0,0,0,0,0,0,0,0,0,0,0,0,0,0,0,0,0,0,0,0,0,0,0,0,0,0,0,0,0,0,0,0,0,0,0,0,0,0,0,0,0,0,0,0,0,0,0,0,0,0,0,0,0,0,0,0,0,0,0,0,0,0,0,0,0,0,0,0,0,0,0,0,0,0,0,0,0,0,0,0,0,0,0,0,0,0,0,0,0,0,0,0,0,0,0,0,0,0,0,0,0,0,0,0,0,0,0,0,0,0,0,0,0,0,0,0,0,0,0,0,0,0,0,0,0,0,0,0,0,0,0,0,0,0,0,0,0,0,0,0,0,0,0,0,0,0,0,0,0,0,0,0,0,0,0,0,0,0,0,0,0,0,0,0,0,0,0,0,0,0,0,0,0,0,0,0,0,0,0,0,0,0,0,0,0,0,0,0,0,0,0,0,0,0,0,0,0,0,0,0,0,0,0,0,0,0,0,0,0,0,0,0,0,0,0,0,0,0,0,0,0,0,0,0,0,0,0,0,0,0,0,0,0,0,0,0,0,0,0,0,0,0,0,0,0,0,0,0,0,0,0,0,0,0,0,0,0,0,0,0,0,0,0,0,0,0,0,0,0,0,0,0,0,0,0,0,0,0,0,0,0,0,0,0,0,0,0,0,0,0,0,0,0,0,0,0,0,0,0,0,0,0,0,0,0,0,0,0,0,0,0,0,0,0,0,0,0,0,0,0,0,0,0,0,0,0,0,0,0,0,0,0,0,0,0,0,0,0,0,0,0,0,0,0,0,0,0,0,0,0,0,0,0,0,0,0,0,0,0,0,0,0,0,0,0,0,0,0,0,0,0,0,0,0,0,0,0,0,0,0,0,0,0,0,0,0,0,0,0,0,0,0,0,0,0,0,0,0,0,0,0,0,0,0,0,0,0,0,0,0,0,0,0,0,0,0,0,0,0,0,0,0,0,0,0,0,0,0,0,0,0,0,0,0,0,0,0,0,0,0,0,0,0,0,0,0,0,0,0,0,0,0,0,0,0,0,0,0,0,0,0,0,0,0,0,0,0,0,0,0,0,0,0,0,0,0,0,0,0,0,0,0,0,0,0,0,0,0,0,0,0,0,0,0,0,0,0,0,0,0,0,0,0,0,0,0,0,0,0,0,0,0,0,0,0,0,0,0,0,0,0,0,0,0,0,0,0,0,0,0,0,0,0,0,0,0,0,0,0,0,0,0,0,0,0,0,0,0,0,0,0,0,0,0,0,0,0,0,0,0,0,0,0,0,0,0,0,0,0,0,0,0,0,0,0,0,0,0,0,0,0,0,0,0,0,0,0,0,0,0,0,0,0,0,0,0,0,0,0,0,0,0,0,0,0,0,0,0,0,0,0,0,0,0,0,0,0,0,0,0,0,0,0,0,0,0,0,0,0,0,0,0,0,0,0,0,0,0,0,0,0,0,0,0,0,0,0,0,0,0,0,0,0,0,0,0,0,0,0,0,0,0,0,0,0,0,0,0,0,0,0,0,0,0,0,0,0,0,0,0,0,0,0,0,0,0,0,0,0,0,0,0,0,0,0,0,0,0,0,0,0,0,0,0,0,0,0,0,0,0,0,0,0,0,0,0,0,0,0,0,0,0,0,0,0,0,0,0,0,0,0,0,0,0,0,0,0,0,0,0,0,0,0,0,0,0,0,0,0,0,0,0,0,0,0,0,0,0,0,0,0,0,0,0,0,0,0,0,0,0,0,0,0,0,0,0,0,0,0,0,0,0,0,0,0,0,0,0,0,0,0,0,0,0,0,0,0,0,0,0,0,0,0,0,0,0,0,0,0,0,0,0,0,0,0,0,0,0,0,0,0,0,0,0,0,0,0,0,0,0,0,0,0,0,0,0,0,0,0,0,0,0,0,0,0,0,0,0,0,0,0,0,0,0,0,0,0,0,0,0,0,0,0,0,0,0,0,0,0,0,0,0,0,0,0,0,0,0,0,0,0,0,0,0,0,0,0,0,0,0,0,0,0,0,0,0,0,0,0,0,0,0,0,0,0,0,0,0,0,0,0,0,0,0,0,0,0,0,0,0,0,0,0,0,0,0,0,0,0,0,0,0,0,0,0,0,0,0,0,0,0,0,0,0,0,0,0,0,0,0,0,0,0,0,0,0,0,0,0,0,0,0,0,0,0,0,0,0,0,0,0,0,0,0,0,0,0,0,0,0,0,0,0,0,0,0,0,0,0,0,0,0,0,0,0,0,0,0,0,0,0,0,0,0,0,0,0,0,0,0,0,0,0,0,0,0,0,0,0,0,0,0,0,0,0,0,0,0,0,0,0,0,0,0,0,0,0,0,0,0,0,0,0,0,0,0,0,0,0,0,0,0,0,0,0,0,0,0,0,0,0,0,0,0,0,0,0,0,0,0,0,0,0,0,0,0,0,0,0,0,0,0,0,0,0,0,0,0,0,0,0,0,0,0,0,0,0,0,0,0,0,0,0,0,0,0,0,0,0,0,0,0,0,0,0,0,0,0,0,0,0,0,0,0,0,0,0,0,0,0,0,0,0,0,0,0,0,0,0,0,0,0,0,0,0,0,0,0,0,0,0,0,0,0,0,0,0,0,0,0,0,0,0,0,0,0,0,0,0,0,0,0,0,0,0,0,0,0,0,0,0,0,0,0,0,0,0,0,0,0,0,0,0,0,0,0,0,0,0,0,0,0,0,0,0,0,0,0,0,0,0,0,0,0,0,0,0,0,0,0,0,0,0,0,0,0,0,0,0,0,0,0,0,0,0,0,0,0,0,0,0,0,0,0,0,0,0,0,0,0,0,0,0,0,0,0,0,0,0,0,0,0,0,0,0,0,0,0,0,0,0,0,0,0,0,0,0,0,0,0,0,0,0,0,0,0,0,0,0,0,0,0,0,0,0,0,0,0,0,0,0,0,0,0,0,0,0,0,0,0,0,0,0,0,0,0,0,0,0,0,0,0,0,0,0,0,0,0,0,0,0,0,0,0,0,0,0,0,0,0,0,0,0,0,0,0,0,0,0,0,0,0,0,0,0,0,0,0,0,0,0,0,0,0,0,0,0,0,0,0,0,0,0,0,0,0,0,0,0,0,0,0,0,0,0,0,0,0,0,0,0,0,0,0,0,0,0,0,0,0,0,0,0,0,0,0,0,0,0,0,0,0,0,0,0,0,0,0,0,0,0,0,0,0,0,0,0,0,0,0,0,0,0,0,0,0,0,0,0,0,0,0,0,0,0,0,0,0 ...(+25083 chars)]  distributed_mem=Block RAM  rst=off  init_reg=0  en=off  latency=1  gui_display_data_type=Floating-point  arith_type=Floating-point  n_bits=16  bin_pt=15  preci_type=Double  exp_width=8  frac_width=24  optimize=Area  use_rpm=on  simulation_type=fast_sim  XmcBlockStatus=1  maskContainerNames=tabcontainer1  block_type=sprom  block_config=sysgen:SPROM_config
  Relational : hdlBasic/Relational  mode=a<b  op_type=Bool  en=off  latency=1  XmcBlockStatus=1  maskContainerNames=tabcontainer1  block_type=relational  block_config=sysgen:Relational_config
  Relational{1..92,95..118,120..122,124..208,210,238..239,250,253,258..262,264..273,275..284,286..295,297..302} (250 alike) : hdlBasic/Relational  mode=a>=b  op_type=Bool  en=off  latency=1  XmcBlockStatus=1  maskContainerNames=tabcontainer1  block_type=relational  block_config=sysgen:Relational_config
  Relational{93..94,119,123,209,211..212} (7 alike) : hdlBasic/Relational  mode=a>b  op_type=Unsigned Fix  en=off  latency=1  XmcBlockStatus=1  maskContainerNames=tabcontainer1  block_type=relational  block_config=sysgen:Relational_config
  Slice : hdlBasic/Slice  nbits=7  boolean_output=off  mode=Lower Bit Location + Width  bit1=-1  base1=MSB of Input  bit0=0  base0=LSB of Input  XmcBlockStatus=1  maskContainerNames=group1  block_type=slice  block_config=sysgen:Slice_config
  Slice1 : hdlBasic/Slice  nbits=7  boolean_output=off  mode=Lower Bit Location + Width  bit1=-1  base1=MSB of Input  bit0=0  base0=LSB of Input  XmcBlockStatus=1  maskContainerNames=group1  block_type=slice  block_config=sysgen:Slice_config
  Slice2 : hdlBasic/Slice  nbits=21  boolean_output=off  mode=Two Bit Locations  bit1=-1  base1=MSB of Input  bit0=1  base0=LSB of Input  XmcBlockStatus=1  maskContainerNames=group1  block_type=slice  block_config=sysgen:Slice_config
  Slice3 : hdlBasic/Slice  nbits=21  boolean_output=off  mode=Two Bit Locations  bit1=-4  base1=MSB of Input  bit0=0  base0=LSB of Input  XmcBlockStatus=1  maskContainerNames=group1  block_type=slice  block_config=sysgen:Slice_config
  To Workspace1 : ToWorkspace  VariableName=xx  SaveFormat=Structure With Time  SampleTime=1
  To Workspace3 : ToWorkspace  VariableName=yy  SaveFormat=Structure With Time  SampleTime=1
  logi_b0 : hdlBasic/Constant  const=-1.0000000000000000000000000000000000000000000000000000000  gui_display_data_type=Floating-point  arith_type=Floating-point  n_bits=8  bin_pt=8  preci_type=Double  exp_width=8  frac_width=24  explicit_period=on  period=1  XmcBlockStatus=1  maskContainerNames=tabcontainer1  block_type=constant  block_config=sysgen:Constant_config
  logi_b1 : hdlBasic/Constant  const=-0.9838709677419354981964261241955682635307312011718750000  gui_display_data_type=Floating-point  arith_type=Floating-point  n_bits=8  bin_pt=8  preci_type=Double  exp_width=8  frac_width=24  explicit_period=on  period=1  XmcBlockStatus=1  maskContainerNames=tabcontainer1  block_type=constant  block_config=sysgen:Constant_config
  logi_b10 : hdlBasic/Constant  const=-0.8387096774193547599196563169243745505809783935546875000  gui_display_data_type=Floating-point  arith_type=Floating-point  n_bits=8  bin_pt=8  preci_type=Double  exp_width=8  frac_width=24  explicit_period=on  period=1  XmcBlockStatus=1  maskContainerNames=tabcontainer1  block_type=constant  block_config=sysgen:Constant_config
  logi_b100 : hdlBasic/Constant  const=0.6129032258064516236473195931466761976480484008789062500  gui_display_data_type=Floating-point  arith_type=Floating-point  n_bits=8  bin_pt=8  preci_type=Double  exp_width=8  frac_width=24  explicit_period=on  period=1  XmcBlockStatus=1  maskContainerNames=tabcontainer1  block_type=constant  block_config=sysgen:Constant_config
  logi_b101 : hdlBasic/Constant  const=0.6290322580645161254508934689511079341173171997070312500  gui_display_data_type=Floating-point  arith_type=Floating-point  n_bits=8  bin_pt=8  preci_type=Double  exp_width=8  frac_width=24  explicit_period=on  period=1  XmcBlockStatus=1  maskContainerNames=tabcontainer1  block_type=constant  block_config=sysgen:Constant_config
  logi_b102 : hdlBasic/Constant  const=0.6451612903225806272544673447555396705865859985351562500  gui_display_data_type=Floating-point  arith_type=Floating-point  n_bits=8  bin_pt=8  preci_type=Double  exp_width=8  frac_width=24  explicit_period=on  period=1  XmcBlockStatus=1  maskContainerNames=tabcontainer1  block_type=constant  block_config=sysgen:Constant_config
  logi_b103 : hdlBasic/Constant  const=0.6612903225806451290580412205599714070558547973632812500  gui_display_data_type=Floating-point  arith_type=Floating-point  n_bits=8  bin_pt=8  preci_type=Double  exp_width=8  frac_width=24  explicit_period=on  period=1  XmcBlockStatus=1  maskContainerNames=tabcontainer1  block_type=constant  block_config=sysgen:Constant_config
  logi_b104 : hdlBasic/Constant  const=0.6774193548387096308616150963644031435251235961914062500  gui_display_data_type=Floating-point  arith_type=Floating-point  n_bits=8  bin_pt=8  preci_type=Double  exp_width=8  frac_width=24  explicit_period=on  period=1  XmcBlockStatus=1  maskContainerNames=tabcontainer1  block_type=constant  block_config=sysgen:Constant_config
  logi_b105 : hdlBasic/Constant  const=0.6935483870967741326651889721688348799943923950195312500  gui_display_data_type=Floating-point  arith_type=Floating-point  n_bits=8  bin_pt=8  preci_type=Double  exp_width=8  frac_width=24  explicit_period=on  period=1  XmcBlockStatus=1  maskContainerNames=tabcontainer1  block_type=constant  block_config=sysgen:Constant_config
  logi_b106 : hdlBasic/Constant  const=0.7096774193548387454910653104889206588268280029296875000  gui_display_data_type=Floating-point  arith_type=Floating-point  n_bits=8  bin_pt=8  preci_type=Double  exp_width=8  frac_width=24  explicit_period=on  period=1  XmcBlockStatus=1  maskContainerNames=tabcontainer1  block_type=constant  block_config=sysgen:Constant_config
  logi_b107 : hdlBasic/Constant  const=0.7258064516129032472946391862933523952960968017578125000  gui_display_data_type=Floating-point  arith_type=Floating-point  n_bits=8  bin_pt=8  preci_type=Double  exp_width=8  frac_width=24  explicit_period=on  period=1  XmcBlockStatus=1  maskContainerNames=tabcontainer1  block_type=constant  block_config=sysgen:Constant_config
  logi_b108 : hdlBasic/Constant  const=0.7419354838709677490982130620977841317653656005859375000  gui_display_data_type=Floating-point  arith_type=Floating-point  n_bits=8  bin_pt=8  preci_type=Double  exp_width=8  frac_width=24  explicit_period=on  period=1  XmcBlockStatus=1  maskContainerNames=tabcontainer1  block_type=constant  block_config=sysgen:Constant_config
  logi_b109 : hdlBasic/Constant  const=0.7580645161290322509017869379022158682346343994140625000  gui_display_data_type=Floating-point  arith_type=Floating-point  n_bits=8  bin_pt=8  preci_type=Double  exp_width=8  frac_width=24  explicit_period=on  period=1  XmcBlockStatus=1  maskContainerNames=tabcontainer1  block_type=constant  block_config=sysgen:Constant_config
  logi_b11 : hdlBasic/Constant  const=-0.8225806451612902581160824411199428141117095947265625000  gui_display_data_type=Floating-point  arith_type=Floating-point  n_bits=8  bin_pt=8  preci_type=Double  exp_width=8  frac_width=24  explicit_period=on  period=1  XmcBlockStatus=1  maskContainerNames=tabcontainer1  block_type=constant  block_config=sysgen:Constant_config
  logi_b110 : hdlBasic/Constant  const=0.7741935483870967527053608137066476047039031982421875000  gui_display_data_type=Floating-point  arith_type=Floating-point  n_bits=8  bin_pt=8  preci_type=Double  exp_width=8  frac_width=24  explicit_period=on  period=1  XmcBlockStatus=1  maskContainerNames=tabcontainer1  block_type=constant  block_config=sysgen:Constant_config
  logi_b111 : hdlBasic/Constant  const=0.7903225806451612545089346895110793411731719970703125000  gui_display_data_type=Floating-point  arith_type=Floating-point  n_bits=8  bin_pt=8  preci_type=Double  exp_width=8  frac_width=24  explicit_period=on  period=1  XmcBlockStatus=1  maskContainerNames=tabcontainer1  block_type=constant  block_config=sysgen:Constant_config
  logi_b112 : hdlBasic/Constant  const=0.8064516129032257563125085653155110776424407958984375000  gui_display_data_type=Floating-point  arith_type=Floating-point  n_bits=8  bin_pt=8  preci_type=Double  exp_width=8  frac_width=24  explicit_period=on  period=1  XmcBlockStatus=1  maskContainerNames=tabcontainer1  block_type=constant  block_config=sysgen:Constant_config
  logi_b113 : hdlBasic/Constant  const=0.8225806451612902581160824411199428141117095947265625000  gui_display_data_type=Floating-point  arith_type=Floating-point  n_bits=8  bin_pt=8  preci_type=Double  exp_width=8  frac_width=24  explicit_period=on  period=1  XmcBlockStatus=1  maskContainerNames=tabcontainer1  block_type=constant  block_config=sysgen:Constant_config
  logi_b114 : hdlBasic/Constant  const=0.8387096774193547599196563169243745505809783935546875000  gui_display_data_type=Floating-point  arith_type=Floating-point  n_bits=8  bin_pt=8  preci_type=Double  exp_width=8  frac_width=24  explicit_period=on  period=1  XmcBlockStatus=1  maskContainerNames=tabcontainer1  block_type=constant  block_config=sysgen:Constant_config
  logi_b115 : hdlBasic/Constant  const=0.8548387096774193727455326552444603294134140014648437500  gui_display_data_type=Floating-point  arith_type=Floating-point  n_bits=8  bin_pt=8  preci_type=Double  exp_width=8  frac_width=24  explicit_period=on  period=1  XmcBlockStatus=1  maskContainerNames=tabcontainer1  block_type=constant  block_config=sysgen:Constant_config
  logi_b116 : hdlBasic/Constant  const=0.8709677419354838745491065310488920658826828002929687500  gui_display_data_type=Floating-point  arith_type=Floating-point  n_bits=8  bin_pt=8  preci_type=Double  exp_width=8  frac_width=24  explicit_period=on  period=1  XmcBlockStatus=1  maskContainerNames=tabcontainer1  block_type=constant  block_config=sysgen:Constant_config
  logi_b117 : hdlBasic/Constant  const=0.8870967741935483763526804068533238023519515991210937500  gui_display_data_type=Floating-point  arith_type=Floating-point  n_bits=8  bin_pt=8  preci_type=Double  exp_width=8  frac_width=24  explicit_period=on  period=1  XmcBlockStatus=1  maskContainerNames=tabcontainer1  block_type=constant  block_config=sysgen:Constant_config
  logi_b118 : hdlBasic/Constant  const=0.9032258064516128781562542826577555388212203979492187500  gui_display_data_type=Floating-point  arith_type=Floating-point  n_bits=8  bin_pt=8  preci_type=Double  exp_width=8  frac_width=24  explicit_period=on  period=1  XmcBlockStatus=1  maskContainerNames=tabcontainer1  block_type=constant  block_config=sysgen:Constant_config
  logi_b119 : hdlBasic/Constant  const=0.9193548387096773799598281584621872752904891967773437500  gui_display_data_type=Floating-point  arith_type=Floating-point  n_bits=8  bin_pt=8  preci_type=Double  exp_width=8  frac_width=24  explicit_period=on  period=1  XmcBlockStatus=1  maskContainerNames=tabcontainer1  block_type=constant  block_config=sysgen:Constant_config
  logi_b12 : hdlBasic/Constant  const=-0.8064516129032257563125085653155110776424407958984375000  gui_display_data_type=Floating-point  arith_type=Floating-point  n_bits=8  bin_pt=8  preci_type=Double  exp_width=8  frac_width=24  explicit_period=on  period=1  XmcBlockStatus=1  maskContainerNames=tabcontainer1  block_type=constant  block_config=sysgen:Constant_config
  logi_b120 : hdlBasic/Constant  const=0.9354838709677418817634020342666190117597579956054687500  gui_display_data_type=Floating-point  arith_type=Floating-point  n_bits=8  bin_pt=8  preci_type=Double  exp_width=8  frac_width=24  explicit_period=on  period=1  XmcBlockStatus=1  maskContainerNames=tabcontainer1  block_type=constant  block_config=sysgen:Constant_config
  logi_b121 : hdlBasic/Constant  const=0.9516129032258063835669759100710507482290267944335937500  gui_display_data_type=Floating-point  arith_type=Floating-point  n_bits=8  bin_pt=8  preci_type=Double  exp_width=8  frac_width=24  explicit_period=on  period=1  XmcBlockStatus=1  maskContainerNames=tabcontainer1  block_type=constant  block_config=sysgen:Constant_config
  logi_b122 : hdlBasic/Constant  const=0.9677419354838709963928522483911365270614624023437500000  gui_display_data_type=Floating-point  arith_type=Floating-point  n_bits=8  bin_pt=8  preci_type=Double  exp_width=8  frac_width=24  explicit_period=on  period=1  XmcBlockStatus=1  maskContainerNames=tabcontainer1  block_type=constant  block_config=sysgen:Constant_config
  logi_b123 : hdlBasic/Constant  const=0.9838709677419354981964261241955682635307312011718750000  gui_display_data_type=Floating-point  arith_type=Floating-point  n_bits=8  bin_pt=8  preci_type=Double  exp_width=8  frac_width=24  explicit_period=on  period=1  XmcBlockStatus=1  maskContainerNames=tabcontainer1  block_type=constant  block_config=sysgen:Constant_config
  logi_b124 : hdlBasic/Constant  const=1.0000000000000000000000000000000000000000000000000000000  gui_display_data_type=Floating-point  arith_type=Floating-point  n_bits=8  bin_pt=8  preci_type=Double  exp_width=8  frac_width=24  explicit_period=on  period=1  XmcBlockStatus=1  maskContainerNames=tabcontainer1  block_type=constant  block_config=sysgen:Constant_config
  logi_b13 : hdlBasic/Constant  const=-0.7903225806451612545089346895110793411731719970703125000  gui_display_data_type=Floating-point  arith_type=Floating-point  n_bits=8  bin_pt=8  preci_type=Double  exp_width=8  frac_width=24  explicit_period=on  period=1  XmcBlockStatus=1  maskContainerNames=tabcontainer1  block_type=constant  block_config=sysgen:Constant_config
  logi_b14 : hdlBasic/Constant  const=-0.7741935483870967527053608137066476047039031982421875000  gui_display_data_type=Floating-point  arith_type=Floating-point  n_bits=8  bin_pt=8  preci_type=Double  exp_width=8  frac_width=24  explicit_period=on  period=1  XmcBlockStatus=1  maskContainerNames=tabcontainer1  block_type=constant  block_config=sysgen:Constant_config
  logi_b15 : hdlBasic/Constant  const=-0.7580645161290322509017869379022158682346343994140625000  gui_display_data_type=Floating-point  arith_type=Floating-point  n_bits=8  bin_pt=8  preci_type=Double  exp_width=8  frac_width=24  explicit_period=on  period=1  XmcBlockStatus=1  maskContainerNames=tabcontainer1  block_type=constant  block_config=sysgen:Constant_config
  logi_b16 : hdlBasic/Constant  const=-0.7419354838709677490982130620977841317653656005859375000  gui_display_data_type=Floating-point  arith_type=Floating-point  n_bits=8  bin_pt=8  preci_type=Double  exp_width=8  frac_width=24  explicit_period=on  period=1  XmcBlockStatus=1  maskContainerNames=tabcontainer1  block_type=constant  block_config=sysgen:Constant_config
  logi_b17 : hdlBasic/Constant  const=-0.7258064516129032472946391862933523952960968017578125000  gui_display_data_type=Floating-point  arith_type=Floating-point  n_bits=8  bin_pt=8  preci_type=Double  exp_width=8  frac_width=24  explicit_period=on  period=1  XmcBlockStatus=1  maskContainerNames=tabcontainer1  block_type=constant  block_config=sysgen:Constant_config
  logi_b18 : hdlBasic/Constant  const=-0.7096774193548387454910653104889206588268280029296875000  gui_display_data_type=Floating-point  arith_type=Floating-point  n_bits=8  bin_pt=8  preci_type=Double  exp_width=8  frac_width=24  explicit_period=on  period=1  XmcBlockStatus=1  maskContainerNames=tabcontainer1  block_type=constant  block_config=sysgen:Constant_config
  logi_b19 : hdlBasic/Constant  const=-0.6935483870967741326651889721688348799943923950195312500  gui_display_data_type=Floating-point  arith_type=Floating-point  n_bits=8  bin_pt=8  preci_type=Double  exp_width=8  frac_width=24  explicit_period=on  period=1  XmcBlockStatus=1  maskContainerNames=tabcontainer1  block_type=constant  block_config=sysgen:Constant_config
  logi_b2 : hdlBasic/Constant  const=-0.9677419354838709963928522483911365270614624023437500000  gui_display_data_type=Floating-point  arith_type=Floating-point  n_bits=8  bin_pt=8  preci_type=Double  exp_width=8  frac_width=24  explicit_period=on  period=1  XmcBlockStatus=1  maskContainerNames=tabcontainer1  block_type=constant  block_config=sysgen:Constant_config
  logi_b20 : hdlBasic/Constant  const=-0.6774193548387096308616150963644031435251235961914062500  gui_display_data_type=Floating-point  arith_type=Floating-point  n_bits=8  bin_pt=8  preci_type=Double  exp_width=8  frac_width=24  explicit_period=on  period=1  XmcBlockStatus=1  maskContainerNames=tabcontainer1  block_type=constant  block_config=sysgen:Constant_config
  logi_b21 : hdlBasic/Constant  const=-0.6612903225806451290580412205599714070558547973632812500  gui_display_data_type=Floating-point  arith_type=Floating-point  n_bits=8  bin_pt=8  preci_type=Double  exp_width=8  frac_width=24  explicit_period=on  period=1  XmcBlockStatus=1  maskContainerNames=tabcontainer1  block_type=constant  block_config=sysgen:Constant_config
  logi_b22 : hdlBasic/Constant  const=-0.6451612903225806272544673447555396705865859985351562500  gui_display_data_type=Floating-point  arith_type=Floating-point  n_bits=8  bin_pt=8  preci_type=Double  exp_width=8  frac_width=24  explicit_period=on  period=1  XmcBlockStatus=1  maskContainerNames=tabcontainer1  block_type=constant  block_config=sysgen:Constant_config
  logi_b23 : hdlBasic/Constant  const=-0.6290322580645161254508934689511079341173171997070312500  gui_display_data_type=Floating-point  arith_type=Floating-point  n_bits=8  bin_pt=8  preci_type=Double  exp_width=8  frac_width=24  explicit_period=on  period=1  XmcBlockStatus=1  maskContainerNames=tabcontainer1  block_type=constant  block_config=sysgen:Constant_config
  logi_b24 : hdlBasic/Constant  const=-0.6129032258064516236473195931466761976480484008789062500  gui_display_data_type=Floating-point  arith_type=Floating-point  n_bits=8  bin_pt=8  preci_type=Double  exp_width=8  frac_width=24  explicit_period=on  period=1  XmcBlockStatus=1  maskContainerNames=tabcontainer1  block_type=constant  block_config=sysgen:Constant_config
  logi_b25 : hdlBasic/Constant  const=-0.5967741935483871218437457173422444611787796020507812500  gui_display_data_type=Floating-point  arith_type=Floating-point  n_bits=8  bin_pt=8  preci_type=Double  exp_width=8  frac_width=24  explicit_period=on  period=1  XmcBlockStatus=1  maskContainerNames=tabcontainer1  block_type=constant  block_config=sysgen:Constant_config
  logi_b26 : hdlBasic/Constant  const=-0.5806451612903225090178693790221586823463439941406250000  gui_display_data_type=Floating-point  arith_type=Floating-point  n_bits=8  bin_pt=8  preci_type=Double  exp_width=8  frac_width=24  explicit_period=on  period=1  XmcBlockStatus=1  maskContainerNames=tabcontainer1  block_type=constant  block_config=sysgen:Constant_config
  logi_b27 : hdlBasic/Constant  const=-0.5645161290322580072142955032177269458770751953125000000  gui_display_data_type=Floating-point  arith_type=Floating-point  n_bits=8  bin_pt=8  preci_type=Double  exp_width=8  frac_width=24  explicit_period=on  period=1  XmcBlockStatus=1  maskContainerNames=tabcontainer1  block_type=constant  block_config=sysgen:Constant_config
  logi_b28 : hdlBasic/Constant  const=-0.5483870967741935054107216274132952094078063964843750000  gui_display_data_type=Floating-point  arith_type=Floating-point  n_bits=8  bin_pt=8  preci_type=Double  exp_width=8  frac_width=24  explicit_period=on  period=1  XmcBlockStatus=1  maskContainerNames=tabcontainer1  block_type=constant  block_config=sysgen:Constant_config
  logi_b29 : hdlBasic/Constant  const=-0.5322580645161290036071477516088634729385375976562500000  gui_display_data_type=Floating-point  arith_type=Floating-point  n_bits=8  bin_pt=8  preci_type=Double  exp_width=8  frac_width=24  explicit_period=on  period=1  XmcBlockStatus=1  maskContainerNames=tabcontainer1  block_type=constant  block_config=sysgen:Constant_config
  logi_b3 : hdlBasic/Constant  const=-0.9516129032258063835669759100710507482290267944335937500  gui_display_data_type=Floating-point  arith_type=Floating-point  n_bits=8  bin_pt=8  preci_type=Double  exp_width=8  frac_width=24  explicit_period=on  period=1  XmcBlockStatus=1  maskContainerNames=tabcontainer1  block_type=constant  block_config=sysgen:Constant_config
  logi_b30 : hdlBasic/Constant  const=-0.5161290322580645018035738758044317364692687988281250000  gui_display_data_type=Floating-point  arith_type=Floating-point  n_bits=8  bin_pt=8  preci_type=Double  exp_width=8  frac_width=24  explicit_period=on  period=1  XmcBlockStatus=1  maskContainerNames=tabcontainer1  block_type=constant  block_config=sysgen:Constant_config
  logi_b31 : hdlBasic/Constant  const=-0.5000000000000000000000000000000000000000000000000000000  gui_display_data_type=Floating-point  arith_type=Floating-point  n_bits=8  bin_pt=8  preci_type=Double  exp_width=8  frac_width=24  explicit_period=on  period=1  XmcBlockStatus=1  maskContainerNames=tabcontainer1  block_type=constant  block_config=sysgen:Constant_config
  logi_b32 : hdlBasic/Constant  const=-0.4838709677419354981964261241955682635307312011718750000  gui_display_data_type=Floating-point  arith_type=Floating-point  n_bits=8  bin_pt=8  preci_type=Double  exp_width=8  frac_width=24  explicit_period=on  period=1  XmcBlockStatus=1  maskContainerNames=tabcontainer1  block_type=constant  block_config=sysgen:Constant_config
  logi_b33 : hdlBasic/Constant  const=-0.4677419354838709408817010171333095058798789978027343750  gui_display_data_type=Floating-point  arith_type=Floating-point  n_bits=8  bin_pt=8  preci_type=Double  exp_width=8  frac_width=24  explicit_period=on  period=1  XmcBlockStatus=1  maskContainerNames=tabcontainer1  block_type=constant  block_config=sysgen:Constant_config
  logi_b34 : hdlBasic/Constant  const=-0.4516129032258064390781271413288777694106101989746093750  gui_display_data_type=Floating-point  arith_type=Floating-point  n_bits=8  bin_pt=8  preci_type=Double  exp_width=8  frac_width=24  explicit_period=on  period=1  XmcBlockStatus=1  maskContainerNames=tabcontainer1  block_type=constant  block_config=sysgen:Constant_config
  logi_b35 : hdlBasic/Constant  const=-0.4354838709677419372745532655244460329413414001464843750  gui_display_data_type=Floating-point  arith_type=Floating-point  n_bits=8  bin_pt=8  preci_type=Double  exp_width=8  frac_width=24  explicit_period=on  period=1  XmcBlockStatus=1  maskContainerNames=tabcontainer1  block_type=constant  block_config=sysgen:Constant_config
  logi_b36 : hdlBasic/Constant  const=-0.4193548387096773799598281584621872752904891967773437500  gui_display_data_type=Floating-point  arith_type=Floating-point  n_bits=8  bin_pt=8  preci_type=Double  exp_width=8  frac_width=24  explicit_period=on  period=1  XmcBlockStatus=1  maskContainerNames=tabcontainer1  block_type=constant  block_config=sysgen:Constant_config
  logi_b37 : hdlBasic/Constant  const=-0.4032258064516128781562542826577555388212203979492187500  gui_display_data_type=Floating-point  arith_type=Floating-point  n_bits=8  bin_pt=8  preci_type=Double  exp_width=8  frac_width=24  explicit_period=on  period=1  XmcBlockStatus=1  maskContainerNames=tabcontainer1  block_type=constant  block_config=sysgen:Constant_config
  logi_b38 : hdlBasic/Constant  const=-0.3870967741935483763526804068533238023519515991210937500  gui_display_data_type=Floating-point  arith_type=Floating-point  n_bits=8  bin_pt=8  preci_type=Double  exp_width=8  frac_width=24  explicit_period=on  period=1  XmcBlockStatus=1  maskContainerNames=tabcontainer1  block_type=constant  block_config=sysgen:Constant_config
  logi_b39 : hdlBasic/Constant  const=-0.3709677419354838745491065310488920658826828002929687500  gui_display_data_type=Floating-point  arith_type=Floating-point  n_bits=8  bin_pt=8  preci_type=Double  exp_width=8  frac_width=24  explicit_period=on  period=1  XmcBlockStatus=1  maskContainerNames=tabcontainer1  block_type=constant  block_config=sysgen:Constant_config
  logi_b4 : hdlBasic/Constant  const=-0.9354838709677418817634020342666190117597579956054687500  gui_display_data_type=Floating-point  arith_type=Floating-point  n_bits=8  bin_pt=8  preci_type=Double  exp_width=8  frac_width=24  explicit_period=on  period=1  XmcBlockStatus=1  maskContainerNames=tabcontainer1  block_type=constant  block_config=sysgen:Constant_config
  logi_b40 : hdlBasic/Constant  const=-0.3548387096774193727455326552444603294134140014648437500  gui_display_data_type=Floating-point  arith_type=Floating-point  n_bits=8  bin_pt=8  preci_type=Double  exp_width=8  frac_width=24  explicit_period=on  period=1  XmcBlockStatus=1  maskContainerNames=tabcontainer1  block_type=constant  block_config=sysgen:Constant_config
  logi_b41 : hdlBasic/Constant  const=-0.3387096774193548154308075481822015717625617980957031250  gui_display_data_type=Floating-point  arith_type=Floating-point  n_bits=8  bin_pt=8  preci_type=Double  exp_width=8  frac_width=24  explicit_period=on  period=1  XmcBlockStatus=1  maskContainerNames=tabcontainer1  block_type=constant  block_config=sysgen:Constant_config
  logi_b42 : hdlBasic/Constant  const=-0.3225806451612903136272336723777698352932929992675781250  gui_display_data_type=Floating-point  arith_type=Floating-point  n_bits=8  bin_pt=8  preci_type=Double  exp_width=8  frac_width=24  explicit_period=on  period=1  XmcBlockStatus=1  maskContainerNames=tabcontainer1  block_type=constant  block_config=sysgen:Constant_config
  logi_b43 : hdlBasic/Constant  const=-0.3064516129032258118236597965733380988240242004394531250  gui_display_data_type=Floating-point  arith_type=Floating-point  n_bits=8  bin_pt=8  preci_type=Double  exp_width=8  frac_width=24  explicit_period=on  period=1  XmcBlockStatus=1  maskContainerNames=tabcontainer1  block_type=constant  block_config=sysgen:Constant_config
  logi_b44 : hdlBasic/Constant  const=-0.2903225806451612545089346895110793411731719970703125000  gui_display_data_type=Floating-point  arith_type=Floating-point  n_bits=8  bin_pt=8  preci_type=Double  exp_width=8  frac_width=24  explicit_period=on  period=1  XmcBlockStatus=1  maskContainerNames=tabcontainer1  block_type=constant  block_config=sysgen:Constant_config
  logi_b45 : hdlBasic/Constant  const=-0.2741935483870967527053608137066476047039031982421875000  gui_display_data_type=Floating-point  arith_type=Floating-point  n_bits=8  bin_pt=8  preci_type=Double  exp_width=8  frac_width=24  explicit_period=on  period=1  XmcBlockStatus=1  maskContainerNames=tabcontainer1  block_type=constant  block_config=sysgen:Constant_config
  logi_b46 : hdlBasic/Constant  const=-0.2580645161290322509017869379022158682346343994140625000  gui_display_data_type=Floating-point  arith_type=Floating-point  n_bits=8  bin_pt=8  preci_type=Double  exp_width=8  frac_width=24  explicit_period=on  period=1  XmcBlockStatus=1  maskContainerNames=tabcontainer1  block_type=constant  block_config=sysgen:Constant_config
  logi_b47 : hdlBasic/Constant  const=-0.2419354838709677490982130620977841317653656005859375000  gui_display_data_type=Floating-point  arith_type=Floating-point  n_bits=8  bin_pt=8  preci_type=Double  exp_width=8  frac_width=24  explicit_period=on  period=1  XmcBlockStatus=1  maskContainerNames=tabcontainer1  block_type=constant  block_config=sysgen:Constant_config
  logi_b48 : hdlBasic/Constant  const=-0.2258064516129032195390635706644388847053050994873046875  gui_display_data_type=Floating-point  arith_type=Floating-point  n_bits=8  bin_pt=8  preci_type=Double  exp_width=8  frac_width=24  explicit_period=on  period=1  XmcBlockStatus=1  maskContainerNames=tabcontainer1  block_type=constant  block_config=sysgen:Constant_config
  logi_b49 : hdlBasic/Constant  const=-0.2096774193548386899799140792310936376452445983886718750  gui_display_data_type=Floating-point  arith_type=Floating-point  n_bits=8  bin_pt=8  preci_type=Double  exp_width=8  frac_width=24  explicit_period=on  period=1  XmcBlockStatus=1  maskContainerNames=tabcontainer1  block_type=constant  block_config=sysgen:Constant_config
  logi_b5 : hdlBasic/Constant  const=-0.9193548387096773799598281584621872752904891967773437500  gui_display_data_type=Floating-point  arith_type=Floating-point  n_bits=8  bin_pt=8  preci_type=Double  exp_width=8  frac_width=24  explicit_period=on  period=1  XmcBlockStatus=1  maskContainerNames=tabcontainer1  block_type=constant  block_config=sysgen:Constant_config
  logi_b50 : hdlBasic/Constant  const=-0.1935483870967741881763402034266619011759757995605468750  gui_display_data_type=Floating-point  arith_type=Floating-point  n_bits=8  bin_pt=8  preci_type=Double  exp_width=8  frac_width=24  explicit_period=on  period=1  XmcBlockStatus=1  maskContainerNames=tabcontainer1  block_type=constant  block_config=sysgen:Constant_config
  logi_b51 : hdlBasic/Constant  const=-0.1774193548387096863727663276222301647067070007324218750  gui_display_data_type=Floating-point  arith_type=Floating-point  n_bits=8  bin_pt=8  preci_type=Double  exp_width=8  frac_width=24  explicit_period=on  period=1  XmcBlockStatus=1  maskContainerNames=tabcontainer1  block_type=constant  block_config=sysgen:Constant_config
  logi_b52 : hdlBasic/Constant  const=-0.1612903225806451568136168361888849176466464996337890625  gui_display_data_type=Floating-point  arith_type=Floating-point  n_bits=8  bin_pt=8  preci_type=Double  exp_width=8  frac_width=24  explicit_period=on  period=1  XmcBlockStatus=1  maskContainerNames=tabcontainer1  block_type=constant  block_config=sysgen:Constant_config
  logi_b53 : hdlBasic/Constant  const=-0.1451612903225806272544673447555396705865859985351562500  gui_display_data_type=Floating-point  arith_type=Floating-point  n_bits=8  bin_pt=8  preci_type=Double  exp_width=8  frac_width=24  explicit_period=on  period=1  XmcBlockStatus=1  maskContainerNames=tabcontainer1  block_type=constant  block_config=sysgen:Constant_config
  logi_b54 : hdlBasic/Constant  const=-0.1290322580645161254508934689511079341173171997070312500  gui_display_data_type=Floating-point  arith_type=Floating-point  n_bits=8  bin_pt=8  preci_type=Double  exp_width=8  frac_width=24  explicit_period=on  period=1  XmcBlockStatus=1  maskContainerNames=tabcontainer1  block_type=constant  block_config=sysgen:Constant_config
  logi_b55 : hdlBasic/Constant  const=-0.1129032258064516097695317853322194423526525497436523438  gui_display_data_type=Floating-point  arith_type=Floating-point  n_bits=8  bin_pt=8  preci_type=Double  exp_width=8  frac_width=24  explicit_period=on  period=1  XmcBlockStatus=1  maskContainerNames=tabcontainer1  block_type=constant  block_config=sysgen:Constant_config
  logi_b56 : hdlBasic/Constant  const=-0.0967741935483870940881701017133309505879878997802734375  gui_display_data_type=Floating-point  arith_type=Floating-point  n_bits=8  bin_pt=8  preci_type=Double  exp_width=8  frac_width=24  explicit_period=on  period=1  XmcBlockStatus=1  maskContainerNames=tabcontainer1  block_type=constant  block_config=sysgen:Constant_config
  logi_b57 : hdlBasic/Constant  const=-0.0806451612903225784068084180944424588233232498168945312  gui_display_data_type=Floating-point  arith_type=Floating-point  n_bits=8  bin_pt=8  preci_type=Double  exp_width=8  frac_width=24  explicit_period=on  period=1  XmcBlockStatus=1  maskContainerNames=tabcontainer1  block_type=constant  block_config=sysgen:Constant_config
  logi_b58 : hdlBasic/Constant  const=-0.0645161290322580627254467344755539670586585998535156250  gui_display_data_type=Floating-point  arith_type=Floating-point  n_bits=8  bin_pt=8  preci_type=Double  exp_width=8  frac_width=24  explicit_period=on  period=1  XmcBlockStatus=1  maskContainerNames=tabcontainer1  block_type=constant  block_config=sysgen:Constant_config
  logi_b59 : hdlBasic/Constant  const=-0.0483870967741935470440850508566654752939939498901367188  gui_display_data_type=Floating-point  arith_type=Floating-point  n_bits=8  bin_pt=8  preci_type=Double  exp_width=8  frac_width=24  explicit_period=on  period=1  XmcBlockStatus=1  maskContainerNames=tabcontainer1  block_type=constant  block_config=sysgen:Constant_config
  logi_b6 : hdlBasic/Constant  const=-0.9032258064516128781562542826577555388212203979492187500  gui_display_data_type=Floating-point  arith_type=Floating-point  n_bits=8  bin_pt=8  preci_type=Double  exp_width=8  frac_width=24  explicit_period=on  period=1  XmcBlockStatus=1  maskContainerNames=tabcontainer1  block_type=constant  block_config=sysgen:Constant_config
  logi_b60 : hdlBasic/Constant  const=-0.0322580645161290313627233672377769835293292999267578125  gui_display_data_type=Floating-point  arith_type=Floating-point  n_bits=8  bin_pt=8  preci_type=Double  exp_width=8  frac_width=24  explicit_period=on  period=1  XmcBlockStatus=1  maskContainerNames=tabcontainer1  block_type=constant  block_config=sysgen:Constant_config
  logi_b61 : hdlBasic/Constant  const=-0.0161290322580645156813616836188884917646646499633789062  gui_display_data_type=Floating-point  arith_type=Floating-point  n_bits=8  bin_pt=8  preci_type=Double  exp_width=8  frac_width=24  explicit_period=on  period=1  XmcBlockStatus=1  maskContainerNames=tabcontainer1  block_type=constant  block_config=sysgen:Constant_config
  logi_b62 : hdlBasic/Constant  const=0.0000000000000000000000000000000000000000000000000000000  gui_display_data_type=Floating-point  arith_type=Floating-point  n_bits=8  bin_pt=8  preci_type=Double  exp_width=8  frac_width=24  explicit_period=on  period=1  XmcBlockStatus=1  maskContainerNames=tabcontainer1  block_type=constant  block_config=sysgen:Constant_config
  logi_b63 : hdlBasic/Constant  const=0.0161290322580645156813616836188884917646646499633789062  gui_display_data_type=Floating-point  arith_type=Floating-point  n_bits=8  bin_pt=8  preci_type=Double  exp_width=8  frac_width=24  explicit_period=on  period=1  XmcBlockStatus=1  maskContainerNames=tabcontainer1  block_type=constant  block_config=sysgen:Constant_config
  logi_b64 : hdlBasic/Constant  const=0.0322580645161290313627233672377769835293292999267578125  gui_display_data_type=Floating-point  arith_type=Floating-point  n_bits=8  bin_pt=8  preci_type=Double  exp_width=8  frac_width=24  explicit_period=on  period=1  XmcBlockStatus=1  maskContainerNames=tabcontainer1  block_type=constant  block_config=sysgen:Constant_config
  logi_b65 : hdlBasic/Constant  const=0.0483870967741935470440850508566654752939939498901367188  gui_display_data_type=Floating-point  arith_type=Floating-point  n_bits=8  bin_pt=8  preci_type=Double  exp_width=8  frac_width=24  explicit_period=on  period=1  XmcBlockStatus=1  maskContainerNames=tabcontainer1  block_type=constant  block_config=sysgen:Constant_config
  logi_b66 : hdlBasic/Constant  const=0.0645161290322580627254467344755539670586585998535156250  gui_display_data_type=Floating-point  arith_type=Floating-point  n_bits=8  bin_pt=8  preci_type=Double  exp_width=8  frac_width=24  explicit_period=on  period=1  XmcBlockStatus=1  maskContainerNames=tabcontainer1  block_type=constant  block_config=sysgen:Constant_config
  logi_b67 : hdlBasic/Constant  const=0.0806451612903225784068084180944424588233232498168945312  gui_display_data_type=Floating-point  arith_type=Floating-point  n_bits=8  bin_pt=8  preci_type=Double  exp_width=8  frac_width=24  explicit_period=on  period=1  XmcBlockStatus=1  maskContainerNames=tabcontainer1  block_type=constant  block_config=sysgen:Constant_config
  logi_b68 : hdlBasic/Constant  const=0.0967741935483870940881701017133309505879878997802734375  gui_display_data_type=Floating-point  arith_type=Floating-point  n_bits=8  bin_pt=8  preci_type=Double  exp_width=8  frac_width=24  explicit_period=on  period=1  XmcBlockStatus=1  maskContainerNames=tabcontainer1  block_type=constant  block_config=sysgen:Constant_config
  logi_b69 : hdlBasic/Constant  const=0.1129032258064516097695317853322194423526525497436523438  gui_display_data_type=Floating-point  arith_type=Floating-point  n_bits=8  bin_pt=8  preci_type=Double  exp_width=8  frac_width=24  explicit_period=on  period=1  XmcBlockStatus=1  maskContainerNames=tabcontainer1  block_type=constant  block_config=sysgen:Constant_config
  logi_b7 : hdlBasic/Constant  const=-0.8870967741935483763526804068533238023519515991210937500  gui_display_data_type=Floating-point  arith_type=Floating-point  n_bits=8  bin_pt=8  preci_type=Double  exp_width=8  frac_width=24  explicit_period=on  period=1  XmcBlockStatus=1  maskContainerNames=tabcontainer1  block_type=constant  block_config=sysgen:Constant_config
  logi_b70 : hdlBasic/Constant  const=0.1290322580645161254508934689511079341173171997070312500  gui_display_data_type=Floating-point  arith_type=Floating-point  n_bits=8  bin_pt=8  preci_type=Double  exp_width=8  frac_width=24  explicit_period=on  period=1  XmcBlockStatus=1  maskContainerNames=tabcontainer1  block_type=constant  block_config=sysgen:Constant_config
  logi_b71 : hdlBasic/Constant  const=0.1451612903225806272544673447555396705865859985351562500  gui_display_data_type=Floating-point  arith_type=Floating-point  n_bits=8  bin_pt=8  preci_type=Double  exp_width=8  frac_width=24  explicit_period=on  period=1  XmcBlockStatus=1  maskContainerNames=tabcontainer1  block_type=constant  block_config=sysgen:Constant_config
  logi_b72 : hdlBasic/Constant  const=0.1612903225806451568136168361888849176466464996337890625  gui_display_data_type=Floating-point  arith_type=Floating-point  n_bits=8  bin_pt=8  preci_type=Double  exp_width=8  frac_width=24  explicit_period=on  period=1  XmcBlockStatus=1  maskContainerNames=tabcontainer1  block_type=constant  block_config=sysgen:Constant_config
  logi_b73 : hdlBasic/Constant  const=0.1774193548387096863727663276222301647067070007324218750  gui_display_data_type=Floating-point  arith_type=Floating-point  n_bits=8  bin_pt=8  preci_type=Double  exp_width=8  frac_width=24  explicit_period=on  period=1  XmcBlockStatus=1  maskContainerNames=tabcontainer1  block_type=constant  block_config=sysgen:Constant_config
  logi_b74 : hdlBasic/Constant  const=0.1935483870967741881763402034266619011759757995605468750  gui_display_data_type=Floating-point  arith_type=Floating-point  n_bits=8  bin_pt=8  preci_type=Double  exp_width=8  frac_width=24  explicit_period=on  period=1  XmcBlockStatus=1  maskContainerNames=tabcontainer1  block_type=constant  block_config=sysgen:Constant_config
  logi_b75 : hdlBasic/Constant  const=0.2096774193548386899799140792310936376452445983886718750  gui_display_data_type=Floating-point  arith_type=Floating-point  n_bits=8  bin_pt=8  preci_type=Double  exp_width=8  frac_width=24  explicit_period=on  period=1  XmcBlockStatus=1  maskContainerNames=tabcontainer1  block_type=constant  block_config=sysgen:Constant_config
  logi_b76 : hdlBasic/Constant  const=0.2258064516129032195390635706644388847053050994873046875  gui_display_data_type=Floating-point  arith_type=Floating-point  n_bits=8  bin_pt=8  preci_type=Double  exp_width=8  frac_width=24  explicit_period=on  period=1  XmcBlockStatus=1  maskContainerNames=tabcontainer1  block_type=constant  block_config=sysgen:Constant_config
  logi_b77 : hdlBasic/Constant  const=0.2419354838709677490982130620977841317653656005859375000  gui_display_data_type=Floating-point  arith_type=Floating-point  n_bits=8  bin_pt=8  preci_type=Double  exp_width=8  frac_width=24  explicit_period=on  period=1  XmcBlockStatus=1  maskContainerNames=tabcontainer1  block_type=constant  block_config=sysgen:Constant_config
  logi_b78 : hdlBasic/Constant  const=0.2580645161290322509017869379022158682346343994140625000  gui_display_data_type=Floating-point  arith_type=Floating-point  n_bits=8  bin_pt=8  preci_type=Double  exp_width=8  frac_width=24  explicit_period=on  period=1  XmcBlockStatus=1  maskContainerNames=tabcontainer1  block_type=constant  block_config=sysgen:Constant_config
  logi_b79 : hdlBasic/Constant  const=0.2741935483870967527053608137066476047039031982421875000  gui_display_data_type=Floating-point  arith_type=Floating-point  n_bits=8  bin_pt=8  preci_type=Double  exp_width=8  frac_width=24  explicit_period=on  period=1  XmcBlockStatus=1  maskContainerNames=tabcontainer1  block_type=constant  block_config=sysgen:Constant_config
  logi_b8 : hdlBasic/Constant  const=-0.8709677419354838745491065310488920658826828002929687500  gui_display_data_type=Floating-point  arith_type=Floating-point  n_bits=8  bin_pt=8  preci_type=Double  exp_width=8  frac_width=24  explicit_period=on  period=1  XmcBlockStatus=1  maskContainerNames=tabcontainer1  block_type=constant  block_config=sysgen:Constant_config
  logi_b80 : hdlBasic/Constant  const=0.2903225806451612545089346895110793411731719970703125000  gui_display_data_type=Floating-point  arith_type=Floating-point  n_bits=8  bin_pt=8  preci_type=Double  exp_width=8  frac_width=24  explicit_period=on  period=1  XmcBlockStatus=1  maskContainerNames=tabcontainer1  block_type=constant  block_config=sysgen:Constant_config
  logi_b81 : hdlBasic/Constant  const=0.3064516129032258118236597965733380988240242004394531250  gui_display_data_type=Floating-point  arith_type=Floating-point  n_bits=8  bin_pt=8  preci_type=Double  exp_width=8  frac_width=24  explicit_period=on  period=1  XmcBlockStatus=1  maskContainerNames=tabcontainer1  block_type=constant  block_config=sysgen:Constant_config
  logi_b82 : hdlBasic/Constant  const=0.3225806451612903136272336723777698352932929992675781250  gui_display_data_type=Floating-point  arith_type=Floating-point  n_bits=8  bin_pt=8  preci_type=Double  exp_width=8  frac_width=24  explicit_period=on  period=1  XmcBlockStatus=1  maskContainerNames=tabcontainer1  block_type=constant  block_config=sysgen:Constant_config
  logi_b83 : hdlBasic/Constant  const=0.3387096774193548154308075481822015717625617980957031250  gui_display_data_type=Floating-point  arith_type=Floating-point  n_bits=8  bin_pt=8  preci_type=Double  exp_width=8  frac_width=24  explicit_period=on  period=1  XmcBlockStatus=1  maskContainerNames=tabcontainer1  block_type=constant  block_config=sysgen:Constant_config
  logi_b84 : hdlBasic/Constant  const=0.3548387096774193727455326552444603294134140014648437500  gui_display_data_type=Floating-point  arith_type=Floating-point  n_bits=8  bin_pt=8  preci_type=Double  exp_width=8  frac_width=24  explicit_period=on  period=1  XmcBlockStatus=1  maskContainerNames=tabcontainer1  block_type=constant  block_config=sysgen:Constant_config
  logi_b85 : hdlBasic/Constant  const=0.3709677419354838745491065310488920658826828002929687500  gui_display_data_type=Floating-point  arith_type=Floating-point  n_bits=8  bin_pt=8  preci_type=Double  exp_width=8  frac_width=24  explicit_period=on  period=1  XmcBlockStatus=1  maskContainerNames=tabcontainer1  block_type=constant  block_config=sysgen:Constant_config
  logi_b86 : hdlBasic/Constant  const=0.3870967741935483763526804068533238023519515991210937500  gui_display_data_type=Floating-point  arith_type=Floating-point  n_bits=8  bin_pt=8  preci_type=Double  exp_width=8  frac_width=24  explicit_period=on  period=1  XmcBlockStatus=1  maskContainerNames=tabcontainer1  block_type=constant  block_config=sysgen:Constant_config
  logi_b87 : hdlBasic/Constant  const=0.4032258064516128781562542826577555388212203979492187500  gui_display_data_type=Floating-point  arith_type=Floating-point  n_bits=8  bin_pt=8  preci_type=Double  exp_width=8  frac_width=24  explicit_period=on  period=1  XmcBlockStatus=1  maskContainerNames=tabcontainer1  block_type=constant  block_config=sysgen:Constant_config
  logi_b88 : hdlBasic/Constant  const=0.4193548387096773799598281584621872752904891967773437500  gui_display_data_type=Floating-point  arith_type=Floating-point  n_bits=8  bin_pt=8  preci_type=Double  exp_width=8  frac_width=24  explicit_period=on  period=1  XmcBlockStatus=1  maskContainerNames=tabcontainer1  block_type=constant  block_config=sysgen:Constant_config
  logi_b89 : hdlBasic/Constant  const=0.4354838709677419372745532655244460329413414001464843750  gui_display_data_type=Floating-point  arith_type=Floating-point  n_bits=8  bin_pt=8  preci_type=Double  exp_width=8  frac_width=24  explicit_period=on  period=1  XmcBlockStatus=1  maskContainerNames=tabcontainer1  block_type=constant  block_config=sysgen:Constant_config
  logi_b9 : hdlBasic/Constant  const=-0.8548387096774193727455326552444603294134140014648437500  gui_display_data_type=Floating-point  arith_type=Floating-point  n_bits=8  bin_pt=8  preci_type=Double  exp_width=8  frac_width=24  explicit_period=on  period=1  XmcBlockStatus=1  maskContainerNames=tabcontainer1  block_type=constant  block_config=sysgen:Constant_config
  logi_b90 : hdlBasic/Constant  const=0.4516129032258064390781271413288777694106101989746093750  gui_display_data_type=Floating-point  arith_type=Floating-point  n_bits=8  bin_pt=8  preci_type=Double  exp_width=8  frac_width=24  explicit_period=on  period=1  XmcBlockStatus=1  maskContainerNames=tabcontainer1  block_type=constant  block_config=sysgen:Constant_config
  logi_b91 : hdlBasic/Constant  const=0.4677419354838709408817010171333095058798789978027343750  gui_display_data_type=Floating-point  arith_type=Floating-point  n_bits=8  bin_pt=8  preci_type=Double  exp_width=8  frac_width=24  explicit_period=on  period=1  XmcBlockStatus=1  maskContainerNames=tabcontainer1  block_type=constant  block_config=sysgen:Constant_config
  logi_b92 : hdlBasic/Constant  const=0.4838709677419354981964261241955682635307312011718750000  gui_display_data_type=Floating-point  arith_type=Floating-point  n_bits=8  bin_pt=8  preci_type=Double  exp_width=8  frac_width=24  explicit_period=on  period=1  XmcBlockStatus=1  maskContainerNames=tabcontainer1  block_type=constant  block_config=sysgen:Constant_config
  logi_b93 : hdlBasic/Constant  const=0.5000000000000000000000000000000000000000000000000000000  gui_display_data_type=Floating-point  arith_type=Floating-point  n_bits=8  bin_pt=8  preci_type=Double  exp_width=8  frac_width=24  explicit_period=on  period=1  XmcBlockStatus=1  maskContainerNames=tabcontainer1  block_type=constant  block_config=sysgen:Constant_config
  logi_b94 : hdlBasic/Constant  const=0.5161290322580645018035738758044317364692687988281250000  gui_display_data_type=Floating-point  arith_type=Floating-point  n_bits=8  bin_pt=8  preci_type=Double  exp_width=8  frac_width=24  explicit_period=on  period=1  XmcBlockStatus=1  maskContainerNames=tabcontainer1  block_type=constant  block_config=sysgen:Constant_config
  logi_b95 : hdlBasic/Constant  const=0.5322580645161290036071477516088634729385375976562500000  gui_display_data_type=Floating-point  arith_type=Floating-point  n_bits=8  bin_pt=8  preci_type=Double  exp_width=8  frac_width=24  explicit_period=on  period=1  XmcBlockStatus=1  maskContainerNames=tabcontainer1  block_type=constant  block_config=sysgen:Constant_config
  logi_b96 : hdlBasic/Constant  const=0.5483870967741935054107216274132952094078063964843750000  gui_display_data_type=Floating-point  arith_type=Floating-point  n_bits=8  bin_pt=8  preci_type=Double  exp_width=8  frac_width=24  explicit_period=on  period=1  XmcBlockStatus=1  maskContainerNames=tabcontainer1  block_type=constant  block_config=sysgen:Constant_config
  logi_b97 : hdlBasic/Constant  const=0.5645161290322580072142955032177269458770751953125000000  gui_display_data_type=Floating-point  arith_type=Floating-point  n_bits=8  bin_pt=8  preci_type=Double  exp_width=8  frac_width=24  explicit_period=on  period=1  XmcBlockStatus=1  maskContainerNames=tabcontainer1  block_type=constant  block_config=sysgen:Constant_config
  logi_b98 : hdlBasic/Constant  const=0.5806451612903225090178693790221586823463439941406250000  gui_display_data_type=Floating-point  arith_type=Floating-point  n_bits=8  bin_pt=8  preci_type=Double  exp_width=8  frac_width=24  explicit_period=on  period=1  XmcBlockStatus=1  maskContainerNames=tabcontainer1  block_type=constant  block_config=sysgen:Constant_config
  logi_b99 : hdlBasic/Constant  const=0.5967741935483871218437457173422444611787796020507812500  gui_display_data_type=Floating-point  arith_type=Floating-point  n_bits=8  bin_pt=8  preci_type=Double  exp_width=8  frac_width=24  explicit_period=on  period=1  XmcBlockStatus=1  maskContainerNames=tabcontainer1  block_type=constant  block_config=sysgen:Constant_config
  logical_x0 : hdlBasic/Mux  inputs=2  en=off  latency=1  precision=Full  arith_type=Unsigned  n_bits=16  bin_pt=14  quantization=Truncate  overflow=Wrap  XmcBlockStatus=1  maskContainerNames=tabcontainer1  block_type=mux  block_config=sysgen:Mux_config
  logical_y0 : hdlBasic/Mux  inputs=2  en=off  latency=1  precision=Full  arith_type=Unsigned  n_bits=16  bin_pt=14  quantization=Truncate  overflow=Wrap  XmcBlockStatus=1  maskContainerNames=tabcontainer1  block_type=mux  block_config=sysgen:Mux_config
  Output : Outport
  wires:
  Mux1/1 -> AddSub1/1, Delay10/1
  AddSub4/1 -> Mux5/3
  In4/1 -> Gate_In2/1
  Mux3/1 -> AddSub3/1, Delay16/1
  Relational3/1 -> Delay9/1
  Mux2/1 -> AddSub2/1, Delay13/1
  Gate_In2/1 -> Relational/2, Delay3/1, Delay2/1
  Mux6/1 -> AddSub6/1, Delay26/1
  AddSub6/1 -> Mux7/3
  In3/1 -> Gate_In1/1
  AddSub/1 -> Mux1/3
  Relational6/1 -> Delay19/1
  AddSub2/1 -> Mux3/3
  Mux/1 -> Delay7/1, AddSub/1
  AddSub1/1 -> Mux2/3
  Relational7/1 -> Delay22/1
  Mux4/1 -> AddSub4/1, Delay20/1
  Relational2/1 -> Mux/1
  AddSub3/1 -> Mux4/3
  Mux7/1 -> AddSub7/1, Delay29/1
  Relational5/1 -> Delay15/1
  Relational4/1 -> Delay12/1
  AddSub5/1 -> Mux6/3
  Mux5/1 -> AddSub5/1, Delay23/1
  AddSub7/1 -> Mux8/3
  Relational8/1 -> Delay25/1
  Gate_In1/1 -> Relational/1, Delay4/1, Delay1/1
  Relational1/1 -> Delay6/1
  Relational9/1 -> Delay28/1
  logical_y0/1 -> Relational2/1, Delay5/1
  Relational/1 -> logical_x0/1, logical_y0/1
  Constant3/1 -> AddSub19/2
  Constant/1 -> AddSub18/2
  AddSub19/1 -> Mult/2
  AddSub18/1 -> Negate/1
  Constant4/1 -> Mult1/2
  AddSub22/1 -> Slice3/1
  AddSub21/1 -> AddSub22/1
  AddSub20/1 -> AddSub21/1
  Mult1/1 -> AddSub20/1
  Negate/1 -> AddSub19/1
  Mult/1 -> Slice2/1
  Delay1/1 -> logical_y0/2
  Delay2/1 -> logical_y0/3
  Delay3/1 -> logical_x0/2
  Delay4/1 -> logical_x0/3
  Delay5/1 -> Relational1/1, Delay8/1
  Delay6/1 -> Mux1/1
  Delay7/1 -> Mux1/2
  Delay8/1 -> Relational3/1, Delay11/1
  Delay9/1 -> Mux2/1
  Delay10/1 -> Mux2/2
  Delay11/1 -> Relational4/1, Delay14/1
  Delay12/1 -> Mux3/1
  Delay13/1 -> Mux3/2
  Delay14/1 -> Relational5/1, Delay17/1
  Delay15/1 -> Mux4/1
  Delay16/1 -> Mux4/2
  Delay17/1 -> Delay18/1, Relational6/1
  Delay18/1 -> Delay21/1, Relational7/1
  Delay19/1 -> Mux5/1
  Delay20/1 -> Mux5/2
  Delay21/1 -> Delay24/1, Relational8/1
  Delay22/1 -> Mux6/1
  Delay23/1 -> Mux6/2
  Delay24/1 -> Relational9/1, Delay27/1
  Delay25/1 -> Mux7/1
  Delay26/1 -> Mux7/2
  Delay28/1 -> Mux8/1
  Delay29/1 -> Mux8/2
  Delay32/1 -> Mux22/2
  Delay48/1 -> Mux27/2
  Relational30/1 -> Delay50/1
  Delay50/1 -> Mux28/1
  Delay36/1 -> Relational26/1, Delay39/1
  Mux24/1 -> AddSub27/1, Delay42/1
  Delay37/1 -> Mux24/1
  logi_b3/1 -> Relational25/2, Relational4/2
  AddSub24/1 -> Mux22/3
  AddSub28/1 -> Mux26/3
  Delay46/1 -> Relational30/1, Delay49/1
  Delay54/1 -> Delay57/1, Relational21/1
  Delay41/1 -> Mux25/1
  logi_b1/1 -> Relational21/2, Relational1/2
  Relational23/1 -> Mux20/1
  AddSub25/1 -> Mux23/3
  Delay35/1 -> Mux23/2
  Delay44/1 -> Mux26/1
  Relational27/1 -> Delay41/1
  logi_b4/1 -> Relational26/2, Relational5/2
  Delay38/1 -> Mux24/2
  logi_b7/1 -> Relational29/2, Relational8/2
  Delay47/1 -> Mux27/1
  Relational24/1 -> Delay58/1
  logi_b0/1 -> Relational23/2, Relational2/2
  Delay51/1 -> Mux28/2
  Delay57/1 -> Delay33/1, Relational24/1
  logi_b5/1 -> Relational27/2, Relational6/2
  Delay56/1 -> Mux21/2
  Delay34/1 -> Mux23/1
  Mux21/1 -> AddSub24/1, Delay32/1
  Relational21/1 -> Delay55/1
  Delay33/1 -> Relational25/1, Delay36/1
  Delay40/1 -> Delay43/1, Relational28/1
  Delay45/1 -> Mux26/2
  Delay43/1 -> Delay46/1, Relational29/1
  Delay58/1 -> Mux22/1
  logi_b2/1 -> Relational3/2, Relational24/2
  AddSub26/1 -> Mux24/3
  Mux22/1 -> AddSub25/1, Delay35/1
  AddSub29/1 -> Mux27/3
  Relational26/1 -> Delay37/1
  Delay42/1 -> Mux25/2
  logi_b6/1 -> Relational28/2, Relational7/2
  Delay55/1 -> Mux21/1
  Delay39/1 -> Delay40/1, Relational27/1
  Mux23/1 -> AddSub26/1, Delay38/1
  Mux20/1 -> Delay56/1, AddSub23/1
  Mux25/1 -> AddSub28/1, Delay45/1
  Mux27/1 -> AddSub30/1, Delay51/1
  Relational29/1 -> Delay47/1
  AddSub27/1 -> Mux25/3
  AddSub30/1 -> Mux28/3
  Relational28/1 -> Delay44/1
  logi_b8/1 -> Relational30/2, Relational9/2
  AddSub23/1 -> Mux21/3
  Mux26/1 -> AddSub29/1, Delay48/1
  logical_x0/1 -> Relational23/1, Delay54/1
  Constant6/1 -> Mux20/2
  Relational25/1 -> Delay34/1
  Constant1/1 -> Mux/2
  Delay59/1 -> Mult1/1
  Delay60/1 -> Mult/1
  Delay61/1 -> AddSub21/2
  Delay100/1 -> Mux31/1
  Delay94/1 -> Mux19/1
  Delay75/1 -> Mux35/2
  Delay87/1 -> Mux17/1
  Delay73/1 -> Delay76/1, Relational35/1
  Delay91/1 -> Mux18/1
  Mux32/1 -> AddSub33/1, Delay68/1
  Delay92/1 -> Mux18/2
  Relational18/1 -> Delay97/1
  AddSub16/1 -> Mux18/3
  Mux12/1 -> AddSub11/1, Delay65/1
  Delay105/1 -> Mux15/1
  Relational14/1 -> Delay84/1
  Delay85/1 -> Mux16/2
  Delay104/1 -> Delay83/1, Relational13/1
  Delay93/1 -> Delay96/1, Relational18/1
  Mux29/1 -> Delay107/1, AddSub9/1
  Relational13/1 -> Delay105/1
  Mux15/1 -> AddSub14/1, Delay85/1
  Relational12/1 -> Delay102/1
  Mux18/1 -> AddSub17/1, Delay95/1
  AddSub9/1 -> Mux11/3
  Delay96/1 -> Relational20/1, Delay99/1
  AddSub33/1 -> Mux33/3
  Delay108/1 -> Delay63/1, Relational19/1
  Relational19/1 -> Delay109/1
  Mux30/1 -> AddSub34/1, Delay101/1
  logi_b11/1 -> Relational13/2, Relational19/2
  Mux11/1 -> AddSub10/1, Delay62/1
  Delay80/1 -> Mux37/1
  Delay71/1 -> Mux34/1
  AddSub32/1 -> Mux30/3
  Delay97/1 -> Mux30/1
  Delay67/1 -> Mux33/1
  Relational16/1 -> Delay91/1
  Relational17/1 -> Delay94/1
  logi_b13/1 -> Relational15/2, Relational32/2
  Delay69/1 -> Delay70/1, Relational33/1
  logi_b15/1 -> Relational17/2, Relational34/2
  Mux19/1 -> AddSub32/1, Delay98/1
  Mux36/1 -> AddSub38/1, Delay81/1
  Relational20/1 -> Delay100/1
  Relational15/1 -> Delay87/1
  Delay76/1 -> Relational36/1, Delay79/1
  Delay84/1 -> Mux16/1
  Mux34/1 -> AddSub36/1, Delay75/1
  AddSub13/1 -> Mux15/3
  logi_b17/1 -> Relational20/2, Relational36/2
  AddSub36/1 -> Mux35/3
  Mux33/1 -> AddSub35/1, Delay72/1
  Mux35/1 -> AddSub37/1, Delay78/1
  Mux17/1 -> AddSub16/1, Delay92/1
  Delay88/1 -> Mux17/2
  Delay66/1 -> Relational32/1, Delay69/1
  AddSub15/1 -> Mux17/3
  Delay89/1 -> Delay90/1, Relational16/1
  Delay109/1 -> Mux12/1
  Delay77/1 -> Mux36/1
  Delay98/1 -> Mux30/2
  AddSub38/1 -> Mux37/3
  Delay72/1 -> Mux34/2
  AddSub35/1 -> Mux34/3
  Mux9/1 -> Delay103/1, AddSub12/1
  AddSub14/1 -> Mux16/3
  Delay95/1 -> Mux19/2
  logi_b12/1 -> Relational14/2, Relational31/2
  Relational34/1 -> Delay74/1
  Delay102/1 -> Mux14/1
  Delay83/1 -> Relational14/1, Delay86/1
  Delay74/1 -> Mux35/1
  Delay81/1 -> Mux37/2
  logi_b10/1 -> Relational12/2, Relational11/2
  logi_b16/1 -> Relational18/2, Relational35/2
  Mux14/1 -> AddSub13/1, Delay82/1
  Delay90/1 -> Delay93/1, Relational17/1
  AddSub12/1 -> Mux14/3
  Relational33/1 -> Delay71/1
  Relational36/1 -> Delay80/1
  Relational11/1 -> Delay106/1
  AddSub34/1 -> Mux31/3
  Delay86/1 -> Relational15/1, Delay89/1
  Delay68/1 -> Mux33/2
  Relational35/1 -> Delay77/1
  Mux16/1 -> AddSub15/1, Delay88/1
  AddSub11/1 -> Mux32/3
  Relational31/1 -> Delay64/1
  Relational32/1 -> Delay67/1
  Delay107/1 -> Mux11/2
  AddSub10/1 -> Mux12/3
  Delay101/1 -> Mux31/2
  Delay103/1 -> Mux14/2
  Delay65/1 -> Mux32/2
  Delay62/1 -> Mux12/2
  AddSub17/1 -> Mux19/3
  AddSub37/1 -> Mux36/3
  Delay70/1 -> Delay73/1, Relational34/1
  logi_b14/1 -> Relational16/2, Relational33/2
  Delay106/1 -> Mux11/1
  Delay82/1 -> Mux15/2
  Delay78/1 -> Mux36/2
  Delay64/1 -> Mux32/1
  Delay63/1 -> Relational31/1, Delay66/1
  Delay111/1 -> Mux39/2
  logi_b49/1 -> Relational38/2, Relational37/2
  Relational37/1 -> Delay110/1
  Delay110/1 -> Mux39/1
  Mux99/1 -> AddSub40/1, Delay111/1
  AddSub39/1 -> Mux38/3
  Delay112/1 -> Mux38/1
  Mux92/1 -> AddSub39/1, Delay113/1
  AddSub40/1 -> Mux39/3
  Relational38/1 -> Delay112/1
  Delay113/1 -> Mux38/2
  AddSub8/1 -> Mux9/3
  AddSub31/1 -> Mux29/3
  Delay49/1 -> Relational10/1, Delay53/1
  Relational10/1 -> Delay114/1
  Delay31/1 -> Mux29/1
  Relational22/1 -> Delay31/1
  Mux28/1 -> AddSub8/1, Delay115/1
  Delay115/1 -> Mux9/2
  Delay52/1 -> Mux29/2
  Delay114/1 -> Mux9/1
  Mux8/1 -> AddSub31/1, Delay52/1
  logi_b9/1 -> Relational10/2, Relational22/2
  Delay27/1 -> Relational22/1, Delay30/1
  AddSub41/1 -> Mux40/3
  AddSub42/1 -> Mux41/3
  Delay99/1 -> Relational39/1, Delay119/1
  Relational39/1 -> Delay120/1
  Delay117/1 -> Mux41/1
  Relational40/1 -> Delay117/1
  Mux31/1 -> AddSub41/1, Delay121/1
  Delay121/1 -> Mux40/2
  Delay118/1 -> Mux41/2
  Delay120/1 -> Mux40/1
  Mux37/1 -> AddSub42/1, Delay118/1
  logi_b18/1 -> Relational39/2, Relational40/2
  Delay79/1 -> Relational40/1, Delay116/1
  Delay30/1 -> Relational11/1, Delay108/1
  Delay53/1 -> Relational12/1, Delay104/1
  Delay116/1 -> Relational41/1, Delay130/1
  Delay154/1 -> Mux54/2
  AddSub50/1 -> Mux47/3
  Delay125/1 -> Mux42/2
  AddSub56/1 -> Mux54/3
  Relational58/1 -> Delay133/1
  Delay123/1 -> Mux49/2
  Mux43/1 -> AddSub47/1, Delay161/1
  Relational42/1 -> Delay124/1
  Delay140/1 -> Mux50/1
  Relational52/1 -> Delay143/1
  Mux53/1 -> AddSub56/1, Delay154/1
  Relational55/1 -> Delay153/1
  Delay144/1 -> Mux51/2
  Relational51/1 -> Delay140/1
  AddSub53/1 -> Mux49/3
  Relational41/1 -> Delay128/1
  Delay145/1 -> Delay146/1, Relational53/1
  logi_b25/1 -> Relational48/2, Relational55/2
  Relational43/1 -> Delay127/1
  Delay142/1 -> Relational52/1, Delay145/1
  Mux45/1 -> AddSub49/1, Delay168/1
  Mux51/1 -> AddSub54/1, Delay148/1
  Delay170/1 -> Mux47/1
  Delay138/1 -> Mux13/2
  Delay162/1 -> Relational45/1, Delay165/1
  logi_b26/1 -> Relational50/2, Relational56/2
  AddSub46/1 -> Mux43/3
  Relational56/1 -> Delay156/1
  Relational53/1 -> Delay147/1
  Delay167/1 -> Mux46/1
  Relational57/1 -> Delay136/1
  Delay130/1 -> Delay139/1, Relational49/1
  Delay134/1 -> Mux57/2
  Delay164/1 -> Mux45/2
  Delay173/1 -> Mux48/1
  AddSub58/1 -> Mux56/3
  Relational45/1 -> Delay163/1
  logi_b22/1 -> Relational45/2, Relational52/2
  Relational50/1 -> Delay122/1
  Relational47/1 -> Delay170/1
  AddSub59/1 -> Mux57/3
  Delay122/1 -> Mux49/1
  Delay137/1 -> Mux56/2
  Relational46/1 -> Delay167/1
  AddSub51/1 -> Mux48/3
  Mux10/1 -> AddSub43/1, Delay138/1
  Delay128/1 -> Mux10/1
  Delay129/1 -> Mux10/2
  AddSub55/1 -> Mux53/3
  Mux54/1 -> AddSub57/1, Delay157/1
  Delay161/1 -> Mux44/2
  logi_b23/1 -> Relational46/2, Relational53/2
  Delay139/1 -> Relational51/1, Delay142/1
  Delay143/1 -> Mux51/1
  Mux48/1 -> AddSub53/1, Delay123/1
  Delay175/1 -> Relational57/1, Delay135/1
  logi_b24/1 -> Relational47/2, Relational54/2
  Mux40/1 -> Delay125/1, AddSub45/1
  AddSub48/1 -> Mux45/3
  Delay168/1 -> Mux46/2
  Delay152/1 -> Relational56/1, Delay155/1
  Mux42/1 -> AddSub46/1, Delay158/1
  AddSub43/1 -> Mux13/3
  Delay133/1 -> Mux57/1
  AddSub52/1 -> Mux51/3
  Delay126/1 -> Delay159/1, Relational43/1
  Mux49/1 -> AddSub58/1, Delay137/1
  AddSub44/1 -> Mux50/3
  Delay165/1 -> Delay166/1, Relational46/1
  Delay147/1 -> Mux52/1
  Mux13/1 -> AddSub44/1, Delay141/1
  AddSub45/1 -> Mux42/3
  logi_b19/1 -> Relational42/2, Relational41/2
  AddSub60/1 -> Mux10/3
  Delay127/1 -> Mux43/1
  Delay166/1 -> Delay169/1, Relational47/1
  logi_b27/1 -> Relational57/2, Relational58/2
  Mux46/1 -> AddSub50/1, Delay171/1
  Delay141/1 -> Mux50/2
  logi_b21/1 -> Relational44/2, Relational51/2
  Relational49/1 -> Delay131/1
  Mux47/1 -> AddSub51/1, Delay174/1
  Delay160/1 -> Mux44/1
  Delay146/1 -> Delay149/1, Relational54/1
  Mux44/1 -> AddSub48/1, Delay164/1
  AddSub47/1 -> Mux44/3
  Mux50/1 -> AddSub52/1, Delay144/1
  Delay157/1 -> Mux55/2
  Delay149/1 -> Delay152/1, Relational55/1
  Mux52/1 -> AddSub55/1, Delay151/1
  Mux41/1 -> Delay129/1, AddSub60/1
  Delay172/1 -> Relational50/1, Delay175/1
  Delay153/1 -> Mux54/1
  Delay156/1 -> Mux55/1
  AddSub49/1 -> Mux46/3
  Delay155/1 -> Relational58/1, Delay132/1
  Relational44/1 -> Delay160/1
  Delay169/1 -> Delay172/1, Relational48/1
  Delay151/1 -> Mux53/2
  Delay163/1 -> Mux45/1
  Relational48/1 -> Delay173/1
  Delay171/1 -> Mux47/2
  Relational54/1 -> Delay150/1
  Delay124/1 -> Mux42/1
  Delay159/1 -> Relational44/1, Delay162/1
  logi_b20/1 -> Relational43/2, Relational49/2
  Delay150/1 -> Mux53/1
  Delay131/1 -> Mux13/1
  Delay174/1 -> Mux48/2
  AddSub57/1 -> Mux55/3
  Delay148/1 -> Mux52/2
  AddSub54/1 -> Mux52/3
  Mux55/1 -> AddSub59/1, Delay134/1
  Delay119/1 -> Relational42/1, Delay126/1
  Delay136/1 -> Mux56/1
  Delay158/1 -> Mux43/2
  AddSub77/1 -> Mux86/3
  Mux75/1 -> AddSub111/1, Delay189/1
  Delay271/1 -> Relational72/1, Delay274/1
  AddSub97/1 -> Mux106/3
  AddSub65/1 -> Mux63/3
  AddSub95/1 -> Mux92/3
  Relational80/1 -> Delay298/1
  Delay268/1 -> Relational60/1, Delay185/1
  Relational65/1 -> Delay323/1
  logi_b45/1 -> Relational89/2, Relational88/2
  Delay298/1 -> Mux81/1
  Delay237/1 -> Relational91/1, Delay241/1
  Delay220/1 -> Mux99/1
  Relational96/1 -> Delay207/1
  Relational62/1 -> Delay182/1
  Delay200/1 -> Mux89/2
  Delay272/1 -> Mux70/1
  Relational89/1 -> Delay199/1
  Delay206/1 -> Delay215/1, Relational96/1
  AddSub79/1 -> Mux76/3
  Delay203/1 -> Mux58/1
  Mux91/1 -> AddSub95/1, Delay243/1
  AddSub100/1 -> Mux99/3
  Delay307/1 -> Relational84/1, Delay310/1
  Mux78/1 -> AddSub82/1, Delay178/1
  AddSub74/1 -> Mux72/3
  Delay239/1 -> Mux91/1
  Mux69/1 -> AddSub72/1, Delay273/1
  Delay243/1 -> Mux92/2
  AddSub68/1 -> Mux66/3
  Relational90/1 -> Delay202/1
  AddSub91/1 -> Mux98/3
  Mux107/1 -> AddSub110/1, Delay267/1
  logi_b47/1 -> Relational91/2, Relational99/2
  Delay304/1 -> Delay307/1, Relational83/1
  logi_b48/1 -> Relational92/2, Relational100/2
  Delay194/1 -> Mux77/1
  AddSub90/1 -> Mux61/3
  Delay262/1 -> Relational110/1, Delay265/1
  Relational79/1 -> Delay295/1
  Delay218/1 -> Mux98/2
  Delay322/1 -> Delay325/1, Relational66/1
  AddSub111/1 -> Mux109/3
  AddSub76/1 -> Mux74/3
  Delay285/1 -> Mux74/1
  Delay294/1 -> Relational79/1, Delay297/1
  Delay202/1 -> Mux90/1
  Delay329/1 -> Mux78/1
  logi_b30/1 -> Relational73/2, Relational97/2
  AddSub109/1 -> Mux58/3
  AddSub70/1 -> Mux77/3
  Delay240/1 -> Mux91/2
  Delay236/1 -> Mux90/2
  Relational60/1 -> Delay183/1
  Delay205/1 -> Mux77/2
  Delay204/1 -> Mux58/2
  Delay191/1 -> Mux88/1
  Mux63/1 -> AddSub66/1, Delay316/1
  Delay328/1 -> Relational69/1, Delay331/1
  Delay266/1 -> Mux108/1
  Delay257/1 -> Mux97/1
  Delay326/1 -> Mux67/1
  Delay331/1 -> Relational85/1, Delay193/1
  Delay287/1 -> Relational59/1, Delay291/1
  AddSub88/1 -> Mux87/3
  Delay309/1 -> Mux84/2
  Relational92/1 -> Delay242/1
  Delay217/1 -> Mux98/1
  Mux70/1 -> AddSub73/1, Delay276/1
  Delay190/1 -> Relational88/1, Delay206/1
  Mux67/1 -> AddSub80/1, Delay330/1
  Delay193/1 -> Relational89/1, Delay201/1
  Delay324/1 -> Mux66/2
  Delay178/1 -> Mux79/2
  Delay177/1 -> Mux79/1
  Mux59/1 -> AddSub62/1, Delay293/1
  Mux64/1 -> AddSub67/1, Delay319/1
  Delay275/1 -> Mux71/1
  Delay219/1 -> Relational100/1, Delay222/1
  logi_b36/1 -> Relational61/2, Relational60/2
  Delay267/1 -> Mux108/2
  Relational85/1 -> Delay195/1
  Delay185/1 -> Delay294/1, Relational68/1
  AddSub92/1 -> Mux89/3
  Mux108/1 -> AddSub79/1, Delay290/1
  Relational88/1 -> Delay203/1
  Mux109/1 -> Delay180/1, AddSub64/1
  Relational91/1 -> Delay239/1
  Relational66/1 -> Delay326/1
  Delay278/1 -> Delay281/1, Relational75/1
  Mux88/1 -> Delay204/1, AddSub109/1
  Mux86/1 -> AddSub87/1, Delay258/1
  Delay310/1 -> Relational87/1, Delay190/1
  Relational99/1 -> Delay217/1
  AddSub63/1 -> Mux80/3
  logi_b40/1 -> Relational65/2, Relational81/2
  AddSub89/1 -> Mux88/3
  Mux82/1 -> AddSub84/1, Delay306/1
  Delay196/1 -> Mux87/2
  Relational69/1 -> Delay177/1
  Mux56/1 -> Delay270/1, AddSub71/1
  Relational64/1 -> Delay318/1
  Mux83/1 -> AddSub85/1, Delay309/1
  Relational75/1 -> Delay282/1
  logi_b39/1 -> Relational64/2, Relational80/2
  Mux62/1 -> AddSub65/1, Delay313/1
  logi_b41/1 -> Relational66/2, Relational82/2
  Delay288/1 -> Mux75/1
  AddSub85/1 -> Mux84/3
  Delay241/1 -> Relational92/1, Delay244/1
  Delay281/1 -> Delay284/1, Relational76/1
  Delay215/1 -> Relational99/1, Delay219/1
  Delay207/1 -> Mux61/1
  Mux87/1 -> Delay200/1, AddSub92/1
  Delay265/1 -> Relational70/1, Delay268/1
  Delay264/1 -> Mux107/2
  Relational61/1 -> Delay179/1
  Delay301/1 -> Delay304/1, Relational82/1
  AddSub72/1 -> Mux70/3
  AddSub80/1 -> Mux78/3
  Delay189/1 -> Mux109/2
  Relational100/1 -> Delay220/1
  AddSub61/1 -> Mux68/3
  AddSub112/1 -> Mux59/3
  Delay199/1 -> Mux89/1
  Delay317/1 -> Relational64/1, Delay320/1
  Delay289/1 -> Mux75/2
  Mux66/1 -> AddSub69/1, Delay327/1
  Delay192/1 -> Mux88/2
  logi_b35/1 -> Relational59/2, Relational70/2
  Delay291/1 -> Relational61/1, Delay181/1
  AddSub71/1 -> Mux69/3
  Mux84/1 -> AddSub86/1, Delay312/1
  Delay259/1 -> Delay262/1, Relational109/1
  Delay302/1 -> Mux82/1
  AddSub64/1 -> Mux62/3
  Delay221/1 -> Mux99/2
  Delay269/1 -> Mux76/1
  Delay305/1 -> Mux83/1
  Mux77/1 -> AddSub77/1, Delay238/1
  Relational68/1 -> Delay186/1
  Delay321/1 -> Mux68/1
  Delay263/1 -> Mux107/1
  AddSub93/1 -> Mux90/3
  AddSub81/1 -> Mux81/3
  Delay315/1 -> Mux64/1
  Delay184/1 -> Mux59/2
  Delay311/1 -> Mux85/1
  Relational81/1 -> Delay302/1
  Delay318/1 -> Mux65/1
  Delay316/1 -> Mux64/2
  Relational70/1 -> Delay269/1
  Mux79/1 -> AddSub88/1, Delay196/1
  logi_b28/1 -> Relational71/2, Relational77/2
  logi_b46/1 -> Relational90/2, Relational96/2
  Delay183/1 -> Mux59/1
  Mux68/1 -> AddSub70/1, Delay205/1
  Delay300/1 -> Delay301/1, Relational81/1
  logi_b42/1 -> Relational67/2, Relational83/2
  Relational107/1 -> Delay257/1
  AddSub94/1 -> Mux91/3
  Delay276/1 -> Mux71/2
  Delay274/1 -> Relational73/1, Delay277/1
  Delay249/1 -> Delay256/1, Relational107/1
  AddSub110/1 -> Mux108/3
  Delay290/1 -> Mux76/2
  Relational73/1 -> Delay275/1
  Mux74/1 -> AddSub78/1, Delay289/1
  Delay258/1 -> Mux97/2
  AddSub87/1 -> Mux97/3
  Mux97/1 -> AddSub97/1, Delay261/1
  Delay312/1 -> Mux85/2
  Delay216/1 -> Relational97/1, Delay249/1
  Delay135/1 -> Delay271/1, Relational71/1
  AddSub73/1 -> Mux71/3
  Delay277/1 -> Delay278/1, Relational74/1
  Relational78/1 -> Delay288/1
  logi_b44/1 -> Relational85/2, Relational87/2
  Delay260/1 -> Mux106/1
  Mux61/1 -> AddSub91/1, Delay218/1
  logi_b32/1 -> Relational75/2, Relational108/2
  Delay214/1 -> Mux61/2
  Delay238/1 -> Mux86/2
  Relational110/1 -> Delay266/1
  Relational84/1 -> Delay311/1
  logi_b43/1 -> Relational69/2, Relational84/2
  AddSub84/1 -> Mux83/3
  Mux81/1 -> AddSub83/1, Delay303/1
  Mux65/1 -> AddSub68/1, Delay324/1
  Delay319/1 -> Mux65/2
  Delay297/1 -> Relational80/1, Delay300/1
  AddSub82/1 -> Mux79/3
  Relational67/1 -> Delay329/1
  Delay299/1 -> Mux81/2
  Relational83/1 -> Delay308/1
  Relational72/1 -> Delay272/1
  Delay292/1 -> Mux69/1
  Delay282/1 -> Mux73/1
  Mux57/1 -> Delay176/1, AddSub61/1
  Delay283/1 -> Mux73/2
  Relational77/1 -> Delay321/1
  Mux89/1 -> AddSub93/1, Delay236/1
  Delay132/1 -> Delay187/1, Relational77/1
  Delay242/1 -> Mux92/1
  Delay303/1 -> Mux82/2
  Mux58/1 -> AddSub90/1, Delay214/1
  Delay284/1 -> Relational78/1, Delay287/1
  Mux98/1 -> AddSub100/1, Delay221/1
  Relational87/1 -> Delay191/1
  Delay201/1 -> Delay237/1, Relational90/1
  Delay306/1 -> Mux83/2
  Mux90/1 -> AddSub94/1, Delay240/1
  Mux76/1 -> Delay184/1, AddSub112/1
  Mux71/1 -> AddSub74/1, Delay280/1
  AddSub78/1 -> Mux75/3
  Delay286/1 -> Mux74/2
  Delay180/1 -> Mux62/2
  Delay296/1 -> Mux80/2
  Delay293/1 -> Mux60/2
  AddSub69/1 -> Mux67/3
  AddSub62/1 -> Mux60/3
  Delay295/1 -> Mux80/1
  Mux60/1 -> AddSub63/1, Delay296/1
  Delay182/1 -> Mux63/1
  AddSub83/1 -> Mux82/3
  Relational59/1 -> Delay188/1
  Relational63/1 -> Delay315/1
  Delay181/1 -> Delay314/1, Relational62/1
  Delay320/1 -> Delay322/1, Relational65/1
  Delay325/1 -> Delay328/1, Relational67/1
  Delay323/1 -> Mux66/1
  Mux80/1 -> AddSub81/1, Delay299/1
  AddSub66/1 -> Mux64/3
  Delay327/1 -> Mux67/2
  logi_b38/1 -> Relational63/2, Relational79/2
  Relational82/1 -> Delay305/1
  Delay179/1 -> Mux62/1
  Delay314/1 -> Relational63/1, Delay317/1
  logi_b37/1 -> Relational62/2, Relational68/2
  AddSub67/1 -> Mux65/3
  Delay186/1 -> Mux60/1
  Delay308/1 -> Mux84/1
  Delay330/1 -> Mux78/2
  AddSub86/1 -> Mux85/3
  Mux85/1 -> AddSub89/1, Delay192/1
  Relational71/1 -> Delay292/1
  Delay227/1 -> Mux86/1
  Mux73/1 -> AddSub76/1, Delay286/1
  logi_b34/1 -> Relational78/2, Relational110/2
  Delay280/1 -> Mux72/2
  Mux72/1 -> AddSub75/1, Delay283/1
  Delay273/1 -> Mux70/2
  Relational109/1 -> Delay263/1
  logi_b29/1 -> Relational72/2, Relational86/2
  Delay261/1 -> Mux106/2
  Relational76/1 -> Delay285/1
  Delay313/1 -> Mux63/2
  logi_b33/1 -> Relational76/2, Relational109/2
  Relational108/1 -> Delay260/1
  Delay195/1 -> Mux87/1
  Relational86/1 -> Delay194/1
  Relational97/1 -> Delay227/1
  Mux106/1 -> AddSub108/1, Delay264/1
  Delay176/1 -> Mux68/2
  AddSub75/1 -> Mux73/3
  Delay256/1 -> Delay259/1, Relational108/1
  logi_b31/1 -> Relational74/2, Relational107/2
  Delay270/1 -> Mux69/2
  AddSub108/1 -> Mux107/3
  Delay188/1 -> Mux109/1
  Delay187/1 -> Relational86/1, Delay216/1
  Delay279/1 -> Mux72/1
  Relational74/1 -> Delay279/1
  Mux93/1 -> Gateway Out/1
  ROM2/1 -> Mux93/4
  Constant8/1 -> Relational93/2
  Relational94/1 -> AddSub96/2
  Relational93/1 -> AddSub96/1
  Delay208/1 -> ROM2/1
  Constant9/1 -> Relational94/2
  ROM1/1 -> Mux93/3
  Delay197/1 -> ROM/1
  ROM/1 -> Mux93/2
  Delay198/1 -> ROM1/1
  Slice2/1 -> AddSub20/2
  AddSub201/1 -> Mux100/3
  Mux114/1 -> AddSub118/1, Delay591/1
  logi_b56/1 -> Relational129/2, Relational185/2
  logi_b84/1 -> Relational162/2, Relational175/2
  AddSub161/1 -> Mux172/3
  Delay335/1 -> Mux143/1
  logi_b83/1 -> Relational183/2, Relational106/2
  AddSub99/1 -> Mux117/3
  Relational159/1 -> Delay367/1
  Delay453/1 -> Mux100/2
  AddSub122/1 -> Mux120/3
  Relational164/1 -> Delay397/1
  AddSub193/1 -> Mux192/3
  Delay563/1 -> Mux132/1
  Delay224/1 -> Mux112/1
  Relational118/1 -> Delay229/1
  Delay440/1 -> Mux196/2
  AddSub101/1 -> Mux105/3
  Delay466/1 -> Mux173/2
  Delay376/1 -> Mux145/2
  Relational131/1 -> Delay548/1
  Delay235/1 -> Mux194/1
  Relational117/1 -> Delay596/1
  logi_b66/1 -> Relational120/2, Relational137/2
  Mux161/1 -> AddSub161/1, Delay451/1
  AddSub119/1 -> Mux116/3
  Mux117/1 -> AddSub120/1, Delay338/1
  AddSub102/1 -> Mux200/3
  Delay347/1 -> Mux110/2
  Delay254/1 -> Mux149/1
  logi_b60/1 -> Relational112/2, Relational118/2
  Delay464/1 -> Relational177/1, Delay467/1
  AddSub152/1 -> Mux148/3
  Relational102/1 -> Delay448/1
  Delay226/1 -> Mux104/2
  Delay233/1 -> Mux137/1
  Delay424/1 -> Relational202/1, Delay428/1
  Delay351/1 -> Mux151/2
  Delay549/1 -> Mux126/2
  AddSub128/1 -> Mux139/3
  Relational127/1 -> Delay538/1
  Mux181/1 -> AddSub186/1, Delay391/1
  AddSub190/1 -> Mux189/3
  Relational183/1 -> Delay482/1
  logi_b94/1 -> Relational195/2, Relational194/2
  logi_b95/1 -> Relational197/2, Relational200/2
  Delay368/1 -> Mux156/2
  Relational192/1 -> Delay409/1
  Delay469/1 -> Mux174/2
  Mux136/1 -> AddSub142/1, Delay248/1
  Delay373/1 -> Mux144/2
  AddSub169/1 -> Mux167/3
  Delay364/1 -> Mux155/1
  Delay359/1 -> Delay363/1, Relational158/1
  Mux124/1 -> AddSub127/1, Delay545/1
  Delay421/1 -> Mux163/1
  Delay411/1 -> Mux191/2
  AddSub137/1 -> Mux136/3
  Relational190/1 -> Delay508/1
  Delay491/1 -> Mux184/2
  logi_b89/1 -> Relational169/2, Relational187/2
  Mux186/1 -> AddSub188/1, Delay502/1
  logi_b62/1 -> Relational114/2, Relational133/2
  Delay493/1 -> Mux185/1
  Delay520/1 -> Delay523/1, Relational170/1
  AddSub151/1 -> Mux147/3
  Delay443/1 -> Mux197/2
  AddSub184/1 -> Mux181/3
  Delay427/1 -> Mux199/2
  Delay255/1 -> Mux149/2
  Relational114/1 -> Delay585/1
  logi_b79/1 -> Relational178/2, Relational201/2
  logi_b64/1 -> Relational116/2, Relational135/2
  AddSub155/1 -> Mux153/3
  Delay494/1 -> Mux185/2
  Delay379/1 -> Mux146/1
  AddSub164/1 -> Mux162/3
  AddSub171/1 -> Mux169/3
  AddSub166/1 -> Mux164/3
  Mux163/1 -> AddSub196/1, Delay427/1
  Relational157/1 -> Delay361/1
  Mux125/1 -> AddSub129/1, Delay549/1
  Delay213/1 -> Mux111/2
  Relational126/1 -> Delay534/1
  Constant7/1 -> AddSub12/2, AddSub45/2, AddSub64/2, AddSub92/2, AddSub121/2, AddSub114/2, AddSub145/2, AddSub166/2, AddSub197/2, AddSub236/2, AddSub298/2, AddSub297/2, AddSub296/2, AddSub295/2, AddSub290/2, AddSub284/2, AddSub282/2, AddSub269/2, AddSub268/2, AddSub267/2, AddSub266/2, AddSub265/2, AddSub264/2, AddSub210/2, AddSub279/2, AddSub277/2, AddSub276/2, AddSub275/2, AddSub274/2, AddSub273/2, AddSub272/2, AddSub257/2, AddSub252/2, AddSub250/2, AddSub249/2, AddSub138/2, AddSub200/2, AddSub199/2, AddSub198/2, AddSub192/2, AddSub186/2, AddSub184/2, AddSub171/2, AddSub170/2, AddSub169/2, AddSub168/2, AddSub167/2, AddSub107/2, AddSub181/2, AddSub179/2, AddSub178/2, AddSub177/2, AddSub176/2, AddSub175/2, AddSub174/2, AddSub159/2, AddSub154/2, AddSub152/2, AddSub151/2, AddSub149/2, AddSub148/2, AddSub147/2, AddSub146/2, AddSub141/2, AddSub133/2, AddSub131/2, AddSub119/2, AddSub118/2, AddSub117/2, AddSub116/2, AddSub115/2, AddSub183/2, AddSub129/2, AddSub127/2, AddSub126/2, AddSub125/2, AddSub124/2, AddSub123/2, AddSub122/2, AddSub39/2, AddSub95/2, AddSub94/2, AddSub93/2, AddSub88/2, AddSub82/2, AddSub80/2, AddSub69/2, AddSub68/2, AddSub67/2, AddSub66/2, AddSub65/2, AddSub111/2, AddSub78/2, AddSub76/2, AddSub75/2, AddSub74/2, AddSub73/2, AddSub72/2, AddSub71/2, AddSub58/2, AddSub53/2, AddSub51/2, AddSub50/2, AddSub49/2, AddSub48/2, AddSub47/2, AddSub46/2, AddSub41/2, AddSub34/2, AddSub32/2, AddSub17/2, AddSub16/2, AddSub15/2, AddSub14/2, AddSub13/2, AddSub8/2, AddSub30/2, AddSub29/2, AddSub28/2, AddSub27/2, AddSub26/2, AddSub25/2, AddSub24/2, AddSub23/2, Mux20/3
  Delay406/1 -> Mux192/1
  Delay434/1 -> Mux161/2
  Delay558/1 -> Mux105/2
  Delay253/1 -> Mux140/2
  Mux158/1 -> Delay389/1, AddSub163/1
  Delay410/1 -> Mux191/1
  Mux100/1 -> AddSub103/1, Delay456/1
  Delay471/1 -> Delay475/1, Relational180/1
  Delay576/1 -> Relational142/1, Delay246/1
  Delay554/1 -> Mux119/2
  Relational187/1 -> Delay498/1
  Delay407/1 -> Mux192/2
  Delay577/1 -> Relational130/1, Delay230/1
  Delay225/1 -> Mux104/1
  Mux171/1 -> AddSub175/1, Delay466/1
  Delay588/1 -> Mux117/1
  Mux177/1 -> AddSub181/1, Delay483/1
  Relational201/1 -> Delay433/1
  Mux123/1 -> AddSub126/1, Delay542/1
  logi_b85/1 -> Relational165/2, Relational164/2
  Delay403/1 -> Mux103/2
  Delay417/1 -> Mux159/1
  Relational95/1 -> Delay557/1
  Delay229/1 -> Mux105/1
  AddSub162/1 -> Mux96/3
  logi_b59/1 -> Relational111/2, Relational105/2
  Relational188/1 -> Delay501/1
  AddSub114/1 -> Mux111/3
  Delay523/1 -> Delay526/1, Relational171/1
  AddSub120/1 -> Mux128/3
  AddSub117/1 -> Mux114/3
  Delay365/1 -> Mux155/2
  Mux105/1 -> AddSub105/1, Delay561/1
  Delay445/1 -> Delay447/1, Relational102/1
  Mux115/1 -> AddSub119/1, Delay594/1
  Relational148/1 -> Delay379/1
  Delay348/1 -> Relational154/1, Delay352/1
  Delay509/1 -> Mux189/2
  Relational195/1 -> Delay412/1
  Delay536/1 -> Delay537/1, Relational127/1
  Delay418/1 -> Mux159/2
  AddSub199/1 -> Mux196/3
  Mux154/1 -> AddSub157/1, Delay365/1
  Delay234/1 -> Mux137/2
  Relational153/1 -> Delay254/1
  Mux38/1 -> Delay554/1, AddSub121/1
  Delay429/1 -> Mux161/1
  AddSub158/1 -> Mux156/3
  Delay370/1 -> Relational146/1, Delay374/1
  Delay535/1 -> Mux122/2
  Delay209/1 -> Mux117/2
  Relational143/1 -> Delay336/1
  Delay528/1 -> Relational125/1, Delay533/1
  Delay552/1 -> Delay555/1, Relational121/1
  Delay349/1 -> Relational152/1, Delay382/1
  Delay470/1 -> Delay471/1, Relational179/1
  Delay580/1 -> Mux112/2
  Delay419/1 -> Mux180/2
  Delay486/1 -> Relational165/1, Delay395/1
  Delay366/1 -> Relational161/1, Delay341/1
  Mux160/1 -> AddSub164/1, Delay488/1
  Mux190/1 -> AddSub191/1, Delay449/1
  Relational186/1 -> Delay493/1
  AddSub185/1 -> Mux185/3
  Mux200/1 -> AddSub140/1, Delay232/1
  Delay385/1 -> Relational153/1, Delay388/1
  AddSub187/1 -> Mux186/3
  Delay513/1 -> Mux166/2
  Delay504/1 -> Mux188/1
  Delay390/1 -> Mux182/1
  logi_b65/1 -> Relational117/2, Relational136/2
  Relational202/1 -> Delay426/1
  Delay468/1 -> Mux174/1
  Relational168/1 -> Delay515/1
  Delay409/1 -> Mux180/1
  AddSub174/1 -> Mux171/3
  AddSub125/1 -> Mux123/3
  Mux129/1 -> AddSub133/1, Delay211/1
  Delay518/1 -> Delay520/1, Relational169/1
  Mux194/1 -> Delay213/1, AddSub114/1
  Mux101/1 -> AddSub106/1, Delay459/1
  Relational140/1 -> Delay252/1
  Delay527/1 -> Mux181/1
  Delay598/1 -> Relational140/1, Delay250/1
  AddSub156/1 -> Mux154/3
  Mux102/1 -> AddSub182/1, Delay485/1
  Relational177/1 -> Delay465/1
  Relational184/1 -> Delay490/1
  AddSub179/1 -> Mux177/3
  Delay481/1 -> Relational162/1, Delay486/1
  Delay555/1 -> Delay528/1, Relational124/1
  Delay381/1 -> Delay385/1, Relational150/1
  Mux172/1 -> AddSub172/1, Delay484/1
  Delay533/1 -> Relational126/1, Delay536/1
  Relational120/1 -> Delay210/1
  Mux183/1 -> AddSub130/1, Delay550/1
  AddSub191/1 -> Mux198/3
  Mux159/1 -> AddSub195/1, Delay423/1
  Mux149/1 -> AddSub159/1, Delay346/1
  Delay568/1 -> Mux133/1
  Delay566/1 -> Mux95/2
  Delay246/1 -> Relational143/1, Delay339/1
  Delay505/1 -> Mux188/2
  logi_b93/1 -> Relational191/2, Relational193/2
  Delay228/1 -> Delay559/1, Relational118/1
  Mux120/1 -> AddSub123/1, Delay532/1
  Relational178/1 -> Delay468/1
  Delay382/1 -> Delay393/1, Relational163/1
  Delay562/1 -> Relational133/1, Delay565/1
  Delay448/1 -> Mux198/1
  Delay355/1 -> Delay356/1, Relational156/1
  Delay371/1 -> Mux139/2
  AddSub196/1 -> Mux199/3
  Mux116/1 -> AddSub131/1, Delay597/1
  Delay451/1 -> Mux172/2
  Relational104/1 -> Delay455/1
  Delay567/1 -> Delay570/1, Relational135/1
  Relational191/1 -> Delay410/1
  Delay346/1 -> Mux157/2
  Delay245/1 -> Mux194/2
  Delay575/1 -> Mux135/2
  Relational175/1 -> Delay461/1
  Delay551/1 -> Relational111/1, Delay223/1
  Delay425/1 -> Relational201/1, Delay445/1
  Mux157/1 -> Delay463/1, AddSub174/1
  Delay455/1 -> Mux101/1
  AddSub175/1 -> Mux173/3
  Delay447/1 -> Delay450/1, Relational103/1
  Delay353/1 -> Mux152/1
  Delay502/1 -> Mux187/2
  Delay537/1 -> Delay540/1, Relational128/1
  logi_b77/1 -> Relational176/2, Relational182/2
  AddSub113/1 -> Mux160/3
  logi_b87/1 -> Relational167/2, Relational184/2
  Delay510/1 -> Mux165/2
  AddSub186/1 -> Mux182/3
  Delay404/1 -> Mux150/1
  Delay482/1 -> Mux178/1
  Delay503/1 -> Relational190/1, Delay507/1
  AddSub132/1 -> Mux132/3
  Relational149/1 -> Delay383/1
  Mux128/1 -> AddSub128/1, Delay371/1
  logi_b63/1 -> Relational115/2, Relational134/2
  logi_b52/1 -> Relational125/2, Relational141/2
  Delay387/1 -> Mux148/2
  AddSub176/1 -> Mux174/3
  AddSub146/1 -> Mux143/3
  AddSub170/1 -> Mux168/3
  Delay472/1 -> Mux175/1
  Delay352/1 -> Relational155/1, Delay355/1
  Delay538/1 -> Mux123/1
  Relational160/1 -> Delay345/1
  Delay250/1 -> Relational144/1, Delay334/1
  AddSub159/1 -> Mux157/3
  AddSub177/1 -> Mux175/3
  Relational198/1 -> Delay438/1
  Delay487/1 -> Mux171/1
  Delay476/1 -> Mux176/1
  Delay211/1 -> Mux130/2
  AddSub153/1 -> Mux152/3
  Delay595/1 -> Relational120/1, Delay598/1
  Delay452/1 -> Mux100/1
  Delay446/1 -> Mux172/1
  Relational200/1 -> Delay421/1
  Delay449/1 -> Mux198/2
  Relational166/1 -> Delay396/1
  Delay572/1 -> Mux134/2
  Delay454/1 -> Relational106/1, Delay457/1
  Delay383/1 -> Mux147/1
  Mux176/1 -> AddSub179/1, Delay480/1
  logi_b55/1 -> Relational128/2, Relational174/2
  Mux143/1 -> AddSub147/1, Delay373/1
  Mux169/1 -> AddSub184/1, Delay529/1
  Delay336/1 -> Mux96/1
  Delay507/1 -> Relational193/1, Delay405/1
  Relational197/1 -> Delay416/1
  Mux148/1 -> AddSub154/1, Delay255/1
  AddSub194/1 -> Mux104/3
  Mux142/1 -> AddSub146/1, Delay369/1
  logi_b61/1 -> Relational113/2, Relational132/2
  Delay460/1 -> Relational164/1, Delay399/1
  Relational125/1 -> Delay531/1
  Relational165/1 -> Delay392/1
  Delay475/1 -> Delay478/1, Relational181/1
  Delay483/1 -> Mux178/2
  Relational105/1 -> Delay225/1
  Delay232/1 -> Mux138/2
  Relational122/1 -> Delay506/1
  Delay539/1 -> Mux123/2
  AddSub148/1 -> Mux145/3
  Mux141/1 -> Delay337/1, AddSub162/1
  AddSub141/1 -> Mux140/3
  Delay584/1 -> Relational114/1, Delay587/1
  Mux103/1 -> Delay394/1, AddSub166/1
  AddSub150/1 -> Mux161/3
  Mux189/1 -> AddSub193/1, Delay407/1
  logi_b73/1 -> Relational149/2, Relational157/2
  Relational163/1 -> Delay404/1
  Delay413/1 -> Mux150/2
  Delay530/1 -> Relational191/1, Delay408/1
  Delay360/1 -> Mux139/1
  logi_b91/1 -> Relational171/2, Relational189/2
  Mux193/1 -> AddSub198/1, Delay435/1
  logi_b82/1 -> Relational181/2, Relational104/2
  Mux180/1 -> AddSub180/1, Delay437/1
  Delay574/1 -> Mux135/1
  Mux185/1 -> AddSub187/1, Delay499/1
  Delay345/1 -> Mux157/1
  Delay393/1 -> Delay422/1, Relational174/1
  AddSub167/1 -> Mux165/3
  Delay531/1 -> Mux121/1
  logi_b90/1 -> Relational170/2, Relational188/2
  Mux188/1 -> AddSub190/1, Delay509/1
  AddSub178/1 -> Mux176/3
  Delay508/1 -> Mux189/1
  Delay212/1 -> Mux111/1
  Delay426/1 -> Mux199/1
  Delay581/1 -> Relational113/1, Delay584/1
  Relational142/1 -> Delay247/1
  Delay412/1 -> Mux193/1
  logi_b54/1 -> Relational127/2, Relational163/2
  Mux111/1 -> AddSub115/1, Delay580/1
  Mux96/1 -> AddSub143/1, Delay347/1
  logi_b50/1 -> Relational121/2, Relational95/2
  Delay251/1 -> Mux128/1
  Relational103/1 -> Delay452/1
  Delay431/1 -> Mux200/2
  AddSub145/1 -> Mux142/3
  Delay392/1 -> Mux164/1
  logi_b58/1 -> Relational98/2, Relational122/2
  Relational111/1 -> Delay212/1
  Mux195/1 -> AddSub199/1, Delay440/1
  Delay405/1 -> Relational194/1, Delay420/1
  AddSub142/1 -> Mux141/3
  Delay565/1 -> Delay567/1, Relational134/1
  Delay369/1 -> Mux143/2
  Delay433/1 -> Mux190/1
  Delay501/1 -> Mux187/1
  Relational139/1 -> Delay233/1
  Mux167/1 -> AddSub170/1, Delay522/1
  Delay465/1 -> Mux173/1
  Delay231/1 -> Mux138/1
  Delay479/1 -> Mux177/1
  AddSub138/1 -> Mux137/3
  Relational156/1 -> Delay357/1
  AddSub157/1 -> Mux155/3
  Delay540/1 -> Delay543/1, Relational129/1
  AddSub143/1 -> Mux110/3
  Delay372/1 -> Mux144/1
  Delay450/1 -> Delay454/1, Relational104/1
  Delay252/1 -> Mux140/1
  Delay556/1 -> Mux120/1
  Delay357/1 -> Mux153/1
  Delay485/1 -> Mux179/2
  Mux198/1 -> AddSub201/1, Delay453/1
  Delay546/1 -> Relational98/1, Delay551/1
  Delay338/1 -> Mux128/2
  logi_b98/1 -> Relational139/2, Relational138/2
  Relational180/1 -> Delay476/1
  Delay344/1 -> Delay464/1, Relational176/1
  Delay400/1 -> Mux162/1
  Delay395/1 -> Delay511/1, Relational166/1
  Delay514/1 -> Relational168/1, Delay518/1
  Mux145/1 -> AddSub149/1, Delay380/1
  Mux196/1 -> AddSub200/1, Delay443/1
  Mux155/1 -> AddSub158/1, Delay368/1
  AddSub103/1 -> Mux101/3
  Delay230/1 -> Relational141/1, Delay349/1
  Delay399/1 -> Delay489/1, Relational172/1
  Mux152/1 -> AddSub155/1, Delay358/1
  Delay561/1 -> Mux131/2
  Delay548/1 -> Mux126/1
  AddSub183/1 -> Mux194/3
  Delay401/1 -> Relational192/1, Delay425/1
  Delay499/1 -> Mux186/2
  Delay545/1 -> Mux125/2
  Delay474/1 -> Mux175/2
  Delay332/1 -> Mux142/1
  Relational182/1 -> Delay519/1
  Delay461/1 -> Mux179/1
  AddSub129/1 -> Mux126/3
  Delay495/1 -> Relational105/1, Delay228/1
  Delay532/1 -> Mux121/2
  Mux119/1 -> AddSub122/1, Delay517/1
  AddSub115/1 -> Mux112/3
  Delay543/1 -> Relational131/1, Delay546/1
  Delay498/1 -> Mux186/1
  Delay389/1 -> Mux170/2
  Relational124/1 -> Delay556/1
  Mux110/1 -> AddSub144/1, Delay351/1
  Delay361/1 -> Mux154/1
  AddSub126/1 -> Mux124/3
  Mux179/1 -> Delay398/1, AddSub113/1
  Delay416/1 -> Mux195/1
  Delay463/1 -> Mux171/2
  Delay343/1 -> Mux158/2
  Delay596/1 -> Mux129/1
  Mux147/1 -> AddSub152/1, Delay387/1
  Delay490/1 -> Mux184/1
  Delay396/1 -> Mux165/1
  Mux165/1 -> AddSub168/1, Delay513/1
  AddSub168/1 -> Mux166/3
  Mux199/1 -> AddSub102/1, Delay431/1
  Mux122/1 -> AddSub125/1, Delay539/1
  AddSub198/1 -> Mux195/3
  Delay521/1 -> Mux168/1
  AddSub135/1 -> Mux134/3
  Delay560/1 -> Mux131/1
  logi_b72/1 -> Relational148/2, Relational156/2
  logi_b97/1 -> Relational199/2, Relational101/2
  Relational158/1 -> Delay364/1
  Relational167/1 -> Delay512/1
  Delay597/1 -> Mux129/2
  Delay582/1 -> Mux113/1
  Relational179/1 -> Delay472/1
  AddSub192/1 -> Mux191/3
  Delay541/1 -> Mux124/1
  Delay435/1 -> Mux195/2
  Delay437/1 -> Mux190/2
  AddSub130/1 -> Mux127/3
  Delay374/1 -> Relational147/1, Delay377/1
  Delay512/1 -> Mux166/1
  AddSub105/1 -> Mux131/3
  Mux39/1 -> Delay566/1, AddSub98/1
  Delay398/1 -> Mux160/2
  Relational196/1 -> Delay473/1
  Relational155/1 -> Delay353/1
  logi_b96/1 -> Relational198/2, Relational202/2
  Mux178/1 -> AddSub107/1, Delay403/1
  AddSub182/1 -> Mux179/3
  Mux150/1 -> AddSub150/1, Delay434/1
  Delay342/1 -> Mux158/1
  Relational170/1 -> Delay524/1
  Delay578/1 -> Mux136/1
  Delay534/1 -> Mux122/1
  Delay571/1 -> Mux134/1
  Relational132/1 -> Delay560/1
  Relational181/1 -> Delay479/1
  Relational169/1 -> Delay521/1
  Relational152/1 -> Delay360/1
  Delay339/1 -> Delay348/1, Relational151/1
  AddSub173/1 -> Mux180/3
  Mux121/1 -> AddSub124/1, Delay535/1
  Relational135/1 -> Delay571/1
  Relational134/1 -> Delay568/1
  AddSub160/1 -> Mux158/3
  Mux164/1 -> AddSub167/1, Delay510/1
  AddSub197/1 -> Mux193/3
  Relational98/1 -> Delay235/1
  Mux139/1 -> AddSub139/1, Delay413/1
  Delay579/1 -> Mux136/2
  Relational194/1 -> Delay417/1
  Delay524/1 -> Mux169/1
  Delay408/1 -> Relational195/1, Delay415/1
  logi_b53/1 -> Relational126/2, Relational152/2
  Delay516/1 -> Mux167/2
  logi_b81/1 -> Relational180/2, Relational103/2
  AddSub104/1 -> Mux159/3
  Delay391/1 -> Mux182/2
  Delay356/1 -> Delay359/1, Relational157/1
  Delay593/1 -> Mux116/1
  Delay564/1 -> Mux132/2
  Relational101/1 -> Delay430/1
  Relational128/1 -> Delay541/1
  Delay506/1 -> Mux127/1
  Delay456/1 -> Mux101/2
  logi_b57/1 -> Relational131/2, Relational196/2
  logi_b88/1 -> Relational168/2, Relational186/2
  Delay438/1 -> Mux196/1
  Delay384/1 -> Mux147/2
  Delay340/1 -> Mux110/1
  Relational161/1 -> Delay342/1
  Mux134/1 -> AddSub136/1, Delay575/1
  Mux175/1 -> AddSub178/1, Delay477/1
  Relational173/1 -> Delay390/1
  AddSub131/1 -> Mux129/3
  Delay526/1 -> Relational173/1, Delay530/1
  Delay247/1 -> Mux141/1
  Delay341/1 -> Delay401/1, Relational182/1
  Mux166/1 -> AddSub169/1, Delay516/1
  Relational141/1 -> Delay251/1
  Relational116/1 -> Delay593/1
  logi_b68/1 -> Relational144/2, Relational143/2
  Mux140/1 -> Delay333/1, AddSub145/1
  Delay380/1 -> Mux146/2
  logi_b74/1 -> Relational150/2, Relational158/2
  Delay375/1 -> Mux145/1
  AddSub189/1 -> Mux188/3
  Mux174/1 -> AddSub177/1, Delay474/1
  Delay337/1 -> Mux96/2
